simulink model "kinovaMicoSimscapeModel"  (R2021b)
(part 39 of 50)

Y3_5_1=dq5*dqr2*sin(q5)*((300773*3^(1/2))/80000000 - 1369/4000000) - (25433*dq2*dqr2*sin(q3))/400000 - (25433*dq1*dqr1*sin(q3))/800000 + (25433*dq1*dqr1*cos(2*q2)*sin(q3))/800000 - (25433*dq1*dqr1*sin(2*q2)*cos(q3))/800000 - (1369*dq4*dqr2*cos(2*q5)*sin(2*q4))/3200000 + (1369*dq5*dqr1*cos(q2)*sin(q3))/4000000 - (1369*dq5*dqr1*cos(q3)*sin(q2))/4000000 - (4107*dq4*dqr1*cos(2*q5)*cos(q2)*sin(q3))/16000000 + (4107*dq4*dqr1*cos(2*q5)*cos(q3)*sin(q2))/16000000 + dq1*dqr1*cos(2*q2)*sin(2*q3)*((23717*3^(1/2))/40000000 - 36744657/1600000000) - dq1*dqr1*cos(2*q3)*sin(2*q2)*((23717*3^(1/2))/40000000 - 36744657/1600000000) + dq4*dqr1*cos(q2)*sin(q3)*((23717*3^(1/2))/20000000 + 2122493/800000000) - dq4*dqr1*cos(q3)*sin(q2)*((23717*3^(1/2))/20000000 + 2122493/800000000) - (1073*3^(1/2)*dq1*dqr1*cos(q5)*sin(q3))/400000 - (1073*3^(1/2)*dq2*dqr2*cos(q5)*sin(q3))/200000 + dq4*dqr2*cos(2*q4)*sin(q5)*((23717*3^(1/2))/20000000 + 1369/1000000) + dq4*dqr2*sin(2*q4)*cos(q5)*((23717*3^(1/2))/40000000 + 1369/2000000) + dq5*dqr2*sin(2*q4)*cos(q5)*((23717*3^(1/2))/40000000 + 1369/2000000) + dq5*dqr2*cos(2*q4)*sin(q5)*((23717*3^(1/2))/80000000 + 1369/4000000) + (1073*dq1*dqr1*cos(q3)*cos(q4)*sin(q5))/200000 + (1073*dq1*dqr1*cos(q3)*cos(q5)*sin(q4))/400000 + (1073*dq2*dqr2*cos(q3)*cos(q4)*sin(q5))/100000 + (1073*dq2*dqr2*cos(q3)*cos(q5)*sin(q4))/200000 - (12321*dq1*dqr1*cos(2*q2)*cos(2*q5)*sin(2*q3))/32000000 + (12321*dq1*dqr1*cos(2*q3)*cos(2*q5)*sin(2*q2))/32000000 - dq2*dqr2*cos(q3)*sin(q4)*((18589*3^(1/2))/2000000 + 1073/100000) - dq1*dqr1*cos(q3)*sin(q4)*((18589*3^(1/2))/4000000 + 1073/200000) - (1369*dq1*dqr1*cos(2*q2)*cos(2*q4)*cos(2*q5)*sin(2*q3))/6400000 + (1369*dq1*dqr1*cos(2*q3)*cos(2*q4)*cos(2*q5)*sin(2*q2))/6400000 - (1073*dq1*dqr1*sin(2*q2)*cos(q4)*sin(q3)*sin(q5))/200000 - (1073*dq1*dqr1*sin(2*q2)*cos(q5)*sin(q3)*sin(q4))/400000 + (1369*3^(1/2)*dq5*dqr1*cos(q2)*cos(q3)*sin(q4))/4000000 + (1369*dq1*dqr1*cos(2*q2)*sin(2*q3)*sin(2*q4)*sin(2*q5))/8000000 - (1369*dq1*dqr1*cos(2*q3)*sin(2*q2)*sin(2*q4)*sin(2*q5))/8000000 + dq1*dqr1*cos(2*q2)*cos(q3)*sin(q4)*((18589*3^(1/2))/4000000 + 1073/200000) + (1369*3^(1/2)*dq5*dqr1*sin(q2)*sin(q3)*sin(q4))/4000000 + (32449*dq1*dqr1*cos(2*q2)*cos(2*q3)*cos(q4)*sin(q5))/4000000 - (1369*dq4*dqr1*cos(2*q4)*cos(2*q5)*cos(q2)*sin(q3))/3200000 + (1369*dq4*dqr1*cos(2*q4)*cos(2*q5)*cos(q3)*sin(q2))/3200000 - (1369*dq5*dqr1*cos(2*q4)*cos(2*q5)*cos(q2)*sin(q3))/4000000 + (1369*dq5*dqr1*cos(2*q4)*cos(2*q5)*cos(q3)*sin(q2))/4000000 + dq1*dqr1*sin(2*q2)*sin(q3)*sin(q4)*((18589*3^(1/2))/4000000 + 1073/200000) - dq1*dqr1*cos(2*q2)*cos(2*q4)*sin(2*q3)*((23717*3^(1/2))/40000000 + 1574893/1600000000) + dq1*dqr1*cos(2*q3)*cos(2*q4)*sin(2*q2)*((23717*3^(1/2))/40000000 + 1574893/1600000000) - dq4*dqr1*cos(2*q4)*cos(q2)*sin(q3)*((23717*3^(1/2))/20000000 + 1574893/800000000) + dq4*dqr1*cos(2*q4)*cos(q3)*sin(q2)*((23717*3^(1/2))/20000000 + 1574893/800000000) + (32449*dq1*dqr1*sin(2*q2)*sin(2*q3)*cos(q4)*sin(q5))/4000000 + (1369*dq4*dqr1*sin(2*q4)*sin(2*q5)*cos(q2)*sin(q3))/4000000 - (1369*dq4*dqr1*sin(2*q4)*sin(2*q5)*cos(q3)*sin(q2))/4000000 + (1369*dq5*dqr1*sin(2*q4)*sin(2*q5)*cos(q2)*sin(q3))/3200000 - (1369*dq5*dqr1*sin(2*q4)*sin(2*q5)*cos(q3)*sin(q2))/3200000 + (1073*3^(1/2)*dq1*dqr1*cos(2*q2)*cos(q5)*sin(q3))/400000 - (1073*3^(1/2)*dq1*dqr1*sin(2*q2)*cos(q3)*cos(q5))/400000 + (32449*dq4*dqr1*cos(q2)*cos(q3)*cos(q4)*sin(q5))/4000000 + (32449*dq5*dqr1*cos(q2)*cos(q3)*cos(q4)*sin(q5))/8000000 + (32449*dq5*dqr1*cos(q2)*cos(q3)*cos(q5)*sin(q4))/4000000 - dq1*dqr1*cos(2*q2)*sin(2*q3)*cos(q5)*((348207*3^(1/2))/80000000 + 1369/4000000) + dq1*dqr1*cos(2*q3)*sin(2*q2)*cos(q5)*((348207*3^(1/2))/80000000 + 1369/4000000) - dq1*dqr1*cos(2*q2)*cos(2*q3)*sin(q4)*((548467*3^(1/2))/80000000 + 32449/4000000) + (32449*dq4*dqr1*cos(q4)*sin(q2)*sin(q3)*sin(q5))/4000000 + (32449*dq5*dqr1*cos(q4)*sin(q2)*sin(q3)*sin(q5))/8000000 + (32449*dq5*dqr1*cos(q5)*sin(q2)*sin(q3)*sin(q4))/4000000 - dq1*dqr1*sin(2*q2)*sin(2*q3)*sin(q4)*((548467*3^(1/2))/80000000 + 32449/4000000) - dq4*dqr1*cos(q2)*cos(q5)*sin(q3)*((23717*3^(1/2))/40000000 + 1369/2000000) + dq4*dqr1*cos(q3)*cos(q5)*sin(q2)*((23717*3^(1/2))/40000000 + 1369/2000000) - dq5*dqr1*cos(q2)*cos(q5)*sin(q3)*((23717*3^(1/2))/40000000 + 1369/2000000) + dq5*dqr1*cos(q3)*cos(q5)*sin(q2)*((23717*3^(1/2))/40000000 + 1369/2000000) - dq4*dqr1*cos(q2)*cos(q3)*sin(q4)*((548467*3^(1/2))/80000000 + 32449/4000000) - (1073*dq1*dqr1*cos(2*q2)*cos(q3)*cos(q4)*sin(q5))/200000 - (1073*dq1*dqr1*cos(2*q2)*cos(q3)*cos(q5)*sin(q4))/400000 - dq4*dqr1*sin(q2)*sin(q3)*sin(q4)*((548467*3^(1/2))/80000000 + 32449/4000000) + (1369*3^(1/2)*dq1*dqr1*cos(2*q2)*cos(2*q3)*cos(2*q5)*sin(q4))/8000000 + (1369*3^(1/2)*dq1*dqr1*cos(2*q2)*cos(2*q3)*sin(2*q5)*cos(q4))/4000000 + dq4*dqr1*cos(2*q4)*cos(q2)*cos(q5)*sin(q3)*((23717*3^(1/2))/40000000 + 1369/2000000) - dq4*dqr1*cos(2*q4)*cos(q3)*cos(q5)*sin(q2)*((23717*3^(1/2))/40000000 + 1369/2000000) + dq5*dqr1*cos(2*q4)*cos(q2)*cos(q5)*sin(q3)*((23717*3^(1/2))/40000000 + 1369/2000000) - dq5*dqr1*cos(2*q4)*cos(q3)*cos(q5)*sin(q2)*((23717*3^(1/2))/40000000 + 1369/2000000) + (1369*3^(1/2)*dq1*dqr1*cos(2*q5)*sin(2*q2)*sin(2*q3)*sin(q4))/8000000 + (1369*3^(1/2)*dq1*dqr1*sin(2*q2)*sin(2*q3)*sin(2*q5)*cos(q4))/4000000 - dq4*dqr1*sin(2*q4)*cos(q2)*sin(q3)*sin(q5)*((23717*3^(1/2))/20000000 + 1369/1000000) + dq4*dqr1*sin(2*q4)*cos(q3)*sin(q2)*sin(q5)*((23717*3^(1/2))/20000000 + 1369/1000000) - dq5*dqr1*sin(2*q4)*cos(q2)*sin(q3)*sin(q5)*((23717*3^(1/2))/80000000 + 1369/4000000) + dq5*dqr1*sin(2*q4)*cos(q3)*sin(q2)*sin(q5)*((23717*3^(1/2))/80000000 + 1369/4000000) + (1369*3^(1/2)*dq4*dqr1*cos(2*q5)*cos(q2)*cos(q3)*sin(q4))/8000000 + (1369*3^(1/2)*dq4*dqr1*sin(2*q5)*cos(q2)*cos(q3)*cos(q4))/4000000 + (1369*3^(1/2)*dq5*dqr1*cos(2*q5)*cos(q2)*cos(q3)*sin(q4))/4000000 + (1369*3^(1/2)*dq5*dqr1*sin(2*q5)*cos(q2)*cos(q3)*cos(q4))/8000000 - dq1*dqr1*cos(2*q2)*cos(2*q3)*cos(q5)*sin(q4)*((1369*3^(1/2))/2000000 - 45547/20000000) + (1369*3^(1/2)*dq4*dqr1*cos(2*q5)*sin(q2)*sin(q3)*sin(q4))/8000000 + (1369*3^(1/2)*dq4*dqr1*sin(2*q5)*cos(q4)*sin(q2)*sin(q3))/4000000 + (1369*3^(1/2)*dq5*dqr1*cos(2*q5)*sin(q2)*sin(q3)*sin(q4))/4000000 + (1369*3^(1/2)*dq5*dqr1*sin(2*q5)*cos(q4)*sin(q2)*sin(q3))/8000000 - dq1*dqr1*sin(2*q2)*sin(2*q3)*cos(q5)*sin(q4)*((1369*3^(1/2))/2000000 - 45547/20000000) - dq4*dqr1*cos(q2)*cos(q3)*cos(q5)*sin(q4)*((1369*3^(1/2))/2000000 - 45547/20000000) - dq4*dqr1*cos(q5)*sin(q2)*sin(q3)*sin(q4)*((1369*3^(1/2))/2000000 - 45547/20000000) + dq1*dqr1*cos(2*q2)*cos(2*q4)*sin(2*q3)*cos(q5)*((23717*3^(1/2))/80000000 + 1369/4000000) - dq1*dqr1*cos(2*q3)*cos(2*q4)*sin(2*q2)*cos(q5)*((23717*3^(1/2))/80000000 + 1369/4000000) - dq1*dqr1*cos(2*q2)*sin(2*q3)*sin(2*q4)*sin(q5)*((23717*3^(1/2))/40000000 + 1369/2000000) + dq1*dqr1*cos(2*q3)*sin(2*q2)*sin(2*q4)*sin(q5)*((23717*3^(1/2))/40000000 + 1369/2000000);
Y3_5_2=(4107*dq2*dqr5*sin(2*q5))/16000000 + (4107*dq5*dqr2*sin(2*q5))/16000000 - (4107*dq5*dqr3*sin(2*q5))/16000000 + dq2*dqr5*sin(q5)*((300773*3^(1/2))/80000000 - 1369/4000000) - dq3*dqr5*sin(q5)*((300773*3^(1/2))/80000000 - 1369/4000000) - dq5*dqr3*sin(q5)*((300773*3^(1/2))/80000000 - 1369/4000000) - dq4*dqr4*sin(q4)*((548467*3^(1/2))/80000000 + 32449/4000000) + (1369*3^(1/2)*dq4*dqr5*sin(q4))/4000000 + (1369*3^(1/2)*dq5*dqr4*sin(q4))/4000000 - (1369*dq2*dqr4*cos(2*q4)*sin(2*q5))/4000000 - (1369*dq2*dqr4*cos(2*q5)*sin(2*q4))/3200000 - (1369*dq4*dqr2*cos(2*q4)*sin(2*q5))/4000000 - (1369*dq2*dqr5*cos(2*q4)*sin(2*q5))/3200000 - (1369*dq2*dqr5*cos(2*q5)*sin(2*q4))/4000000 + (1369*dq3*dqr4*cos(2*q4)*sin(2*q5))/4000000 + (1369*dq3*dqr4*cos(2*q5)*sin(2*q4))/3200000 + (1369*dq4*dqr3*cos(2*q4)*sin(2*q5))/4000000 + (1369*dq4*dqr3*cos(2*q5)*sin(2*q4))/3200000 - (1369*dq5*dqr2*cos(2*q4)*sin(2*q5))/3200000 - (1369*dq5*dqr2*cos(2*q5)*sin(2*q4))/4000000 + (1369*dq5*dqr3*cos(2*q4)*sin(2*q5))/3200000 + (1369*dq5*dqr3*cos(2*q5)*sin(2*q4))/4000000 - dq2*dqr4*sin(2*q4)*((23717*3^(1/2))/20000000 + 1574893/800000000) - dq4*dqr2*sin(2*q4)*((23717*3^(1/2))/20000000 + 1574893/800000000) + dq3*dqr4*sin(2*q4)*((23717*3^(1/2))/20000000 + 1574893/800000000) + dq4*dqr3*sin(2*q4)*((23717*3^(1/2))/20000000 + 1574893/800000000) + (1369*dq1*dqr5*cos(q2)*sin(q3))/4000000 - (1369*dq1*dqr5*cos(q3)*sin(q2))/4000000 + (32449*dq4*dqr4*cos(q4)*sin(q5))/4000000 + (32449*dq4*dqr5*cos(q4)*sin(q5))/8000000 + (32449*dq4*dqr5*cos(q5)*sin(q4))/4000000 + (32449*dq5*dqr4*cos(q4)*sin(q5))/8000000 + (32449*dq5*dqr4*cos(q5)*sin(q4))/4000000 + (32449*dq5*dqr5*cos(q4)*sin(q5))/4000000 + dq5*dqr5*cos(q5)*sin(q4)*((1369*3^(1/2))/2000000 + 58349/10000000) - dq4*dqr4*cos(q5)*sin(q4)*((1369*3^(1/2))/2000000 - 45547/20000000) - (4107*dq1*dqr4*cos(2*q5)*cos(q2)*sin(q3))/16000000 + (4107*dq1*dqr4*cos(2*q5)*cos(q3)*sin(q2))/16000000 + dq1*dqr4*cos(q2)*sin(q3)*((23717*3^(1/2))/20000000 + 2122493/800000000) - dq1*dqr4*cos(q3)*sin(q2)*((23717*3^(1/2))/20000000 + 2122493/800000000) + dq2*dqr4*cos(2*q4)*sin(q5)*((23717*3^(1/2))/20000000 + 1369/1000000) - dq3*dqr4*cos(2*q4)*sin(q5)*((23717*3^(1/2))/20000000 + 1369/1000000) - dq4*dqr3*cos(2*q4)*sin(q5)*((23717*3^(1/2))/20000000 + 1369/1000000) + dq2*dqr4*sin(2*q4)*cos(q5)*((23717*3^(1/2))/40000000 + 1369/2000000) + dq2*dqr5*sin(2*q4)*cos(q5)*((23717*3^(1/2))/40000000 + 1369/2000000) - dq3*dqr4*sin(2*q4)*cos(q5)*((23717*3^(1/2))/40000000 + 1369/2000000) - dq4*dqr3*sin(2*q4)*cos(q5)*((23717*3^(1/2))/40000000 + 1369/2000000) - dq3*dqr5*sin(2*q4)*cos(q5)*((23717*3^(1/2))/40000000 + 1369/2000000) - dq5*dqr3*sin(2*q4)*cos(q5)*((23717*3^(1/2))/40000000 + 1369/2000000) + dq2*dqr5*cos(2*q4)*sin(q5)*((23717*3^(1/2))/80000000 + 1369/4000000) - dq3*dqr5*cos(2*q4)*sin(q5)*((23717*3^(1/2))/80000000 + 1369/4000000) - dq5*dqr3*cos(2*q4)*sin(q5)*((23717*3^(1/2))/80000000 + 1369/4000000) + (1369*3^(1/2)*dq4*dqr4*cos(2*q5)*sin(q4))/8000000 + (1369*3^(1/2)*dq4*dqr4*sin(2*q5)*cos(q4))/4000000 + (1369*3^(1/2)*dq4*dqr5*cos(2*q5)*sin(q4))/4000000 + (1369*3^(1/2)*dq4*dqr5*sin(2*q5)*cos(q4))/8000000 + (1369*3^(1/2)*dq5*dqr4*cos(2*q5)*sin(q4))/4000000 + (1369*3^(1/2)*dq5*dqr4*sin(2*q5)*cos(q4))/8000000 + (1369*3^(1/2)*dq1*dqr5*cos(q2)*cos(q3)*sin(q4))/4000000 + (1369*3^(1/2)*dq1*dqr5*sin(q2)*sin(q3)*sin(q4))/4000000 - (1369*dq1*dqr4*cos(2*q4)*cos(2*q5)*cos(q2)*sin(q3))/3200000 + (1369*dq1*dqr4*cos(2*q4)*cos(2*q5)*cos(q3)*sin(q2))/3200000 - (1369*dq1*dqr5*cos(2*q4)*cos(2*q5)*cos(q2)*sin(q3))/4000000 + (1369*dq1*dqr5*cos(2*q4)*cos(2*q5)*cos(q3)*sin(q2))/4000000 - dq1*dqr4*cos(2*q4)*cos(q2)*sin(q3)*((23717*3^(1/2))/20000000 + 1574893/800000000) + dq1*dqr4*cos(2*q4)*cos(q3)*sin(q2)*((23717*3^(1/2))/20000000 + 1574893/800000000) + (1369*dq1*dqr4*sin(2*q4)*sin(2*q5)*cos(q2)*sin(q3))/4000000 - (1369*dq1*dqr4*sin(2*q4)*sin(2*q5)*cos(q3)*sin(q2))/4000000 + (1369*dq1*dqr5*sin(2*q4)*sin(2*q5)*cos(q2)*sin(q3))/3200000 - (1369*dq1*dqr5*sin(2*q4)*sin(2*q5)*cos(q3)*sin(q2))/3200000 + (32449*dq1*dqr4*cos(q2)*cos(q3)*cos(q4)*sin(q5))/4000000 + (32449*dq1*dqr5*cos(q2)*cos(q3)*cos(q4)*sin(q5))/8000000 + (32449*dq1*dqr5*cos(q2)*cos(q3)*cos(q5)*sin(q4))/4000000 + (32449*dq1*dqr4*cos(q4)*sin(q2)*sin(q3)*sin(q5))/4000000 + (32449*dq1*dqr5*cos(q4)*sin(q2)*sin(q3)*sin(q5))/8000000 + (32449*dq1*dqr5*cos(q5)*sin(q2)*sin(q3)*sin(q4))/4000000 - dq1*dqr4*cos(q2)*cos(q5)*sin(q3)*((23717*3^(1/2))/40000000 + 1369/2000000) + dq1*dqr4*cos(q3)*cos(q5)*sin(q2)*((23717*3^(1/2))/40000000 + 1369/2000000) - dq1*dqr5*cos(q2)*cos(q5)*sin(q3)*((23717*3^(1/2))/40000000 + 1369/2000000) + dq1*dqr5*cos(q3)*cos(q5)*sin(q2)*((23717*3^(1/2))/40000000 + 1369/2000000) - dq1*dqr4*cos(q2)*cos(q3)*sin(q4)*((548467*3^(1/2))/80000000 + 32449/4000000) - dq1*dqr4*sin(q2)*sin(q3)*sin(q4)*((548467*3^(1/2))/80000000 + 32449/4000000) + dq1*dqr4*cos(2*q4)*cos(q2)*cos(q5)*sin(q3)*((23717*3^(1/2))/40000000 + 1369/2000000) - dq1*dqr4*cos(2*q4)*cos(q3)*cos(q5)*sin(q2)*((23717*3^(1/2))/40000000 + 1369/2000000) + dq1*dqr5*cos(2*q4)*cos(q2)*cos(q5)*sin(q3)*((23717*3^(1/2))/40000000 + 1369/2000000) - dq1*dqr5*cos(2*q4)*cos(q3)*cos(q5)*sin(q2)*((23717*3^(1/2))/40000000 + 1369/2000000) - dq1*dqr4*sin(2*q4)*cos(q2)*sin(q3)*sin(q5)*((23717*3^(1/2))/20000000 + 1369/1000000) + dq1*dqr4*sin(2*q4)*cos(q3)*sin(q2)*sin(q5)*((23717*3^(1/2))/20000000 + 1369/1000000) - dq1*dqr5*sin(2*q4)*cos(q2)*sin(q3)*sin(q5)*((23717*3^(1/2))/80000000 + 1369/4000000) + dq1*dqr5*sin(2*q4)*cos(q3)*sin(q2)*sin(q5)*((23717*3^(1/2))/80000000 + 1369/4000000) + (1369*3^(1/2)*dq1*dqr4*cos(2*q5)*cos(q2)*cos(q3)*sin(q4))/8000000 + (1369*3^(1/2)*dq1*dqr4*sin(2*q5)*cos(q2)*cos(q3)*cos(q4))/4000000 + (1369*3^(1/2)*dq1*dqr5*cos(2*q5)*cos(q2)*cos(q3)*sin(q4))/4000000 + (1369*3^(1/2)*dq1*dqr5*sin(2*q5)*cos(q2)*cos(q3)*cos(q4))/8000000 + (1369*3^(1/2)*dq1*dqr4*cos(2*q5)*sin(q2)*sin(q3)*sin(q4))/8000000 + (1369*3^(1/2)*dq1*dqr4*sin(2*q5)*cos(q4)*sin(q2)*sin(q3))/4000000 + (1369*3^(1/2)*dq1*dqr5*cos(2*q5)*sin(q2)*sin(q3)*sin(q4))/4000000 + (1369*3^(1/2)*dq1*dqr5*sin(2*q5)*cos(q4)*sin(q2)*sin(q3))/8000000 - dq1*dqr4*cos(q2)*cos(q3)*cos(q5)*sin(q4)*((1369*3^(1/2))/2000000 - 45547/20000000) - dq1*dqr4*cos(q5)*sin(q2)*sin(q3)*sin(q4)*((1369*3^(1/2))/2000000 - 45547/20000000);
Y3_5_3=(25433*ddqr2*cos(q3))/400000 - ddqr2*((23717*3^(1/2))/10000000 + 5252117/100000000) + ddqr3*((23717*3^(1/2))/10000000 + 5252117/100000000) - (1369*ddqr2*cos(q5)^2)/1000000 + (1369*ddqr3*cos(q5)^2)/1000000 + (1369*ddqr2*cos(q4)^2*cos(q5)^2)/800000 - (1369*ddqr3*cos(q4)^2*cos(q5)^2)/800000 + ddqr2*cos(q4)^2*((23717*3^(1/2))/10000000 + 1232643/400000000) - ddqr3*cos(q4)^2*((23717*3^(1/2))/10000000 + 1232643/400000000) - (4107*dq3*dqr5*sin(2*q5))/16000000 - (6139*ddqr1*cos(q2)*cos(q3))/4000000 - (32449*ddqr5*cos(q4)*cos(q5))/4000000 - (6139*ddqr1*sin(q2)*sin(q3))/4000000 + (32449*ddqr4*sin(q4)*sin(q5))/4000000 - ddqr2*cos(q5)*((4329*3^(1/2))/625000 - 1369/1000000) + ddqr3*cos(q5)*((4329*3^(1/2))/625000 - 1369/1000000) + ddqr4*cos(q4)*((562157*3^(1/2))/80000000 + 32449/4000000) - (1369*3^(1/2)*ddqr5*cos(q4))/2000000 - (1369*3^(1/2)*ddqr4*cos(q4)*cos(q5)^2)/4000000 + (1073*ddqr2*cos(q4)*sin(q3)*sin(q5))/100000 + (1073*ddqr2*cos(q5)*sin(q3)*sin(q4))/200000 + ddqr4*cos(q4)*cos(q5)*((1369*3^(1/2))/2000000 - 45547/20000000) + (1369*dq3*dqr5*cos(2*q4)*sin(2*q5))/3200000 + (1369*dq3*dqr5*cos(2*q5)*sin(2*q4))/4000000 - ddqr2*sin(q3)*sin(q4)*((18589*3^(1/2))/2000000 + 1073/100000) + ddqr5*sin(q4)*sin(q5)*((1369*3^(1/2))/2000000 + 58349/10000000) + (1073*3^(1/2)*ddqr2*cos(q3)*cos(q5))/200000 - ddqr2*cos(q4)^2*cos(q5)*((23717*3^(1/2))/20000000 + 1369/1000000) + ddqr3*cos(q4)^2*cos(q5)*((23717*3^(1/2))/20000000 + 1369/1000000) + (32449*ddqr1*cos(q2)*cos(q3)*sin(q4)*sin(q5))/4000000 - (259*ddqr1*cos(q2)*cos(q4)*sin(q3)*sin(q5))/1000000 - (259*ddqr1*cos(q2)*cos(q5)*sin(q3)*sin(q4))/2000000 + (259*ddqr1*cos(q3)*cos(q4)*sin(q2)*sin(q5))/1000000 + (259*ddqr1*cos(q3)*cos(q5)*sin(q2)*sin(q4))/2000000 + (1369*ddqr1*cos(q2)*cos(q5)*sin(q3)*sin(q5))/2000000 - (1369*ddqr1*cos(q3)*cos(q5)*sin(q2)*sin(q5))/2000000 - (1369*ddqr2*cos(q4)*cos(q5)*sin(q4)*sin(q5))/1000000 + (1369*ddqr3*cos(q4)*cos(q5)*sin(q4)*sin(q5))/1000000 + (32449*ddqr1*sin(q2)*sin(q3)*sin(q4)*sin(q5))/4000000 + ddqr1*cos(q2)*cos(q3)*cos(q4)*((562157*3^(1/2))/80000000 + 32449/4000000) + ddqr2*cos(q4)*sin(q4)*sin(q5)*((23717*3^(1/2))/10000000 + 1369/500000) - ddqr3*cos(q4)*sin(q4)*sin(q5)*((23717*3^(1/2))/10000000 + 1369/500000) + ddqr1*cos(q2)*sin(q3)*sin(q4)*((4487*3^(1/2))/20000000 + 259/1000000) - ddqr1*cos(q3)*sin(q2)*sin(q4)*((4487*3^(1/2))/20000000 + 259/1000000) - ddqr1*cos(q2)*sin(q3)*sin(q5)*((23717*3^(1/2))/20000000 + 1369/1000000) + ddqr1*cos(q3)*sin(q2)*sin(q5)*((23717*3^(1/2))/20000000 + 1369/1000000) + ddqr1*cos(q4)*sin(q2)*sin(q3)*((562157*3^(1/2))/80000000 + 32449/4000000) - (259*3^(1/2)*ddqr1*cos(q2)*cos(q3)*cos(q5))/2000000 - (259*3^(1/2)*ddqr1*cos(q5)*sin(q2)*sin(q3))/2000000 + (1369*3^(1/2)*ddqr4*cos(q5)*sin(q4)*sin(q5))/2000000 + ddqr1*cos(q2)*cos(q3)*cos(q4)*cos(q5)*((1369*3^(1/2))/2000000 - 45547/20000000) + ddqr1*cos(q4)*cos(q5)*sin(q2)*sin(q3)*((1369*3^(1/2))/2000000 - 45547/20000000) - (1369*ddqr1*cos(q2)*cos(q4)*cos(q5)^2*sin(q3)*sin(q4))/800000 + (1369*ddqr1*cos(q3)*cos(q4)*cos(q5)^2*sin(q2)*sin(q4))/800000 - (1369*ddqr1*cos(q2)*cos(q4)^2*cos(q5)*sin(q3)*sin(q5))/1000000 + (1369*ddqr1*cos(q3)*cos(q4)^2*cos(q5)*sin(q2)*sin(q5))/1000000 - ddqr1*cos(q2)*cos(q4)*sin(q3)*sin(q4)*((23717*3^(1/2))/10000000 + 1232643/400000000) + ddqr1*cos(q3)*cos(q4)*sin(q2)*sin(q4)*((23717*3^(1/2))/10000000 + 1232643/400000000) + ddqr1*cos(q2)*cos(q4)^2*sin(q3)*sin(q5)*((23717*3^(1/2))/10000000 + 1369/500000) - ddqr1*cos(q3)*cos(q4)^2*sin(q2)*sin(q5)*((23717*3^(1/2))/10000000 + 1369/500000) - (1369*3^(1/2)*ddqr1*cos(q2)*cos(q3)*cos(q4)*cos(q5)^2)/4000000 - (1369*3^(1/2)*ddqr1*cos(q4)*cos(q5)^2*sin(q2)*sin(q3))/4000000 + ddqr1*cos(q2)*cos(q4)*cos(q5)*sin(q3)*sin(q4)*((23717*3^(1/2))/20000000 + 1369/1000000) - ddqr1*cos(q3)*cos(q4)*cos(q5)*sin(q2)*sin(q4)*((23717*3^(1/2))/20000000 + 1369/1000000) + (1369*3^(1/2)*ddqr1*cos(q2)*cos(q3)*cos(q5)*sin(q4)*sin(q5))/2000000 + (1369*3^(1/2)*ddqr1*cos(q5)*sin(q2)*sin(q3)*sin(q4)*sin(q5))/2000000;
Y3_7_1=(29*ddqr2*cos(q3))/100 - (29*dq1*dqr1*sin(q3))/200 - (29*dq2*dqr2*sin(q3))/100 + (ddqr1*cos(q2)*cos(q3))/625 + (ddqr1*sin(q2)*sin(q3))/625 + (29*dq1*dqr1*cos(2*q2)*sin(q3))/200 - (29*dq1*dqr1*sin(2*q2)*cos(q3))/200;
Y3_8_1=(1231*dq4*dqr4*sin(q4))/10000 - (1231*ddqr4*cos(q4))/10000 + (29*ddqr2*sin(q3)*sin(q4))/100 - (1231*ddqr1*cos(q2)*cos(q3)*cos(q4))/10000 - (7*ddqr1*cos(q2)*sin(q3)*sin(q4))/1000 + (7*ddqr1*cos(q3)*sin(q2)*sin(q4))/1000 - (1231*ddqr1*cos(q4)*sin(q2)*sin(q3))/10000 + (29*dq1*dqr1*cos(q3)*sin(q4))/200 + (29*dq2*dqr2*cos(q3)*sin(q4))/100 - (29*dq1*dqr1*cos(2*q2)*cos(q3)*sin(q4))/200 - (29*dq1*dqr1*sin(2*q2)*sin(q3)*sin(q4))/200 + (1231*dq1*dqr1*cos(2*q2)*cos(2*q3)*sin(q4))/10000 + (1231*dq1*dqr1*sin(2*q2)*sin(2*q3)*sin(q4))/10000 + (1231*dq1*dqr4*cos(q2)*cos(q3)*sin(q4))/10000 + (1231*dq4*dqr1*cos(q2)*cos(q3)*sin(q4))/10000 + (1231*dq1*dqr4*sin(q2)*sin(q3)*sin(q4))/10000 + (1231*dq4*dqr1*sin(q2)*sin(q3)*sin(q4))/10000;
Y3_9_1=dq3*dqr5*sin(q5)*((117*3^(1/2))/1250 - 37/4000) - dq5*dqr2*sin(q5)*((117*3^(1/2))/1250 - 37/4000) - dq2*dqr5*sin(q5)*((117*3^(1/2))/1250 - 37/4000) + dq5*dqr3*sin(q5)*((117*3^(1/2))/1250 - 37/4000) - (37*dq2*dqr4*cos(2*q4)*sin(q5))/1000 - (37*dq2*dqr4*sin(2*q4)*cos(q5))/2000 - (37*dq4*dqr2*cos(2*q4)*sin(q5))/1000 - (37*dq4*dqr2*sin(2*q4)*cos(q5))/2000 - (37*dq2*dqr5*cos(2*q4)*sin(q5))/4000 - (37*dq2*dqr5*sin(2*q4)*cos(q5))/2000 + (37*dq3*dqr4*cos(2*q4)*sin(q5))/1000 + (37*dq3*dqr4*sin(2*q4)*cos(q5))/2000 + (37*dq4*dqr3*cos(2*q4)*sin(q5))/1000 + (37*dq4*dqr3*sin(2*q4)*cos(q5))/2000 - (37*dq5*dqr2*cos(2*q4)*sin(q5))/4000 - (37*dq5*dqr2*sin(2*q4)*cos(q5))/2000 + (37*dq3*dqr5*cos(2*q4)*sin(q5))/4000 + (37*dq3*dqr5*sin(2*q4)*cos(q5))/2000 + (37*dq5*dqr3*cos(2*q4)*sin(q5))/4000 + (37*dq5*dqr3*sin(2*q4)*cos(q5))/2000 - (37*ddqr1*cos(q3)*sin(q2)*sin(q5))/1000 - (117*dq4*dqr4*cos(q4)*sin(q5))/625 - (117*dq4*dqr5*cos(q4)*sin(q5))/1250 - (117*dq4*dqr5*cos(q5)*sin(q4))/625 - (117*dq5*dqr4*cos(q4)*sin(q5))/1250 - (117*dq5*dqr4*cos(q5)*sin(q4))/625 - (117*dq5*dqr5*cos(q4)*sin(q5))/625 + (7*ddqr1*cos(q2)*cos(q5)*sin(q3)*sin(q4))/2000 - (7*ddqr1*cos(q3)*cos(q4)*sin(q2)*sin(q5))/1000 - (7*ddqr1*cos(q3)*cos(q5)*sin(q2)*sin(q4))/2000 + (29*3^(1/2)*dq1*dqr1*cos(q5)*sin(q3))/400 + (29*3^(1/2)*dq2*dqr2*cos(q5)*sin(q3))/200 - (117*ddqr1*sin(q2)*sin(q3)*sin(q4)*sin(q5))/625 + (37*ddqr1*cos(q3)*cos(q4)^2*sin(q2)*sin(q5))/500 - (29*dq1*dqr1*cos(q3)*cos(q4)*sin(q5))/200 - (29*dq1*dqr1*cos(q3)*cos(q5)*sin(q4))/400 + (37*dq1*dqr4*cos(q2)*cos(q5)*sin(q3))/2000 - (37*dq1*dqr4*cos(q3)*cos(q5)*sin(q2))/2000 + (37*dq4*dqr1*cos(q2)*cos(q5)*sin(q3))/2000 - (37*dq4*dqr1*cos(q3)*cos(q5)*sin(q2))/2000 + (37*dq1*dqr5*cos(q2)*cos(q5)*sin(q3))/2000 - (37*dq1*dqr5*cos(q3)*cos(q5)*sin(q2))/2000 - (29*dq2*dqr2*cos(q3)*cos(q4)*sin(q5))/100 - (29*dq2*dqr2*cos(q3)*cos(q5)*sin(q4))/200 + (37*dq5*dqr1*cos(q2)*cos(q5)*sin(q3))/2000 - (37*dq5*dqr1*cos(q3)*cos(q5)*sin(q2))/2000 + (7*3^(1/2)*ddqr1*cos(q5)*sin(q2)*sin(q3))/2000 + dq4*dqr4*cos(q5)*sin(q4)*((37*3^(1/2))/2000 - 117/1250) - dq5*dqr5*cos(q5)*sin(q4)*((37*3^(1/2))/2000 + 117/1250) + (29*dq1*dqr1*sin(2*q2)*cos(q4)*sin(q3)*sin(q5))/200 + (29*dq1*dqr1*sin(2*q2)*cos(q5)*sin(q3)*sin(q4))/400 + (37*dq1*dqr4*sin(2*q4)*cos(q2)*sin(q3)*sin(q5))/1000 - (37*dq1*dqr4*sin(2*q4)*cos(q3)*sin(q2)*sin(q5))/1000 + (37*dq4*dqr1*sin(2*q4)*cos(q2)*sin(q3)*sin(q5))/1000 - (37*dq4*dqr1*sin(2*q4)*cos(q3)*sin(q2)*sin(q5))/1000 + (37*dq1*dqr5*sin(2*q4)*cos(q2)*sin(q3)*sin(q5))/4000 - (37*dq1*dqr5*sin(2*q4)*cos(q3)*sin(q2)*sin(q5))/4000 + (37*dq5*dqr1*sin(2*q4)*cos(q2)*sin(q3)*sin(q5))/4000 - (37*dq5*dqr1*sin(2*q4)*cos(q3)*sin(q2)*sin(q5))/4000 - (37*ddqr1*cos(q2)*cos(q4)*cos(q5)*sin(q3)*sin(q4))/1000 + (37*ddqr1*cos(q3)*cos(q4)*cos(q5)*sin(q2)*sin(q4))/1000 - (117*dq1*dqr1*cos(2*q2)*cos(2*q3)*cos(q4)*sin(q5))/625 - ddqr1*cos(q4)*cos(q5)*sin(q2)*sin(q3)*((37*3^(1/2))/2000 - 117/1250) - (117*dq1*dqr1*sin(2*q2)*sin(2*q3)*cos(q4)*sin(q5))/625 - (29*3^(1/2)*dq1*dqr1*cos(2*q2)*cos(q5)*sin(q3))/400 + (29*3^(1/2)*dq1*dqr1*sin(2*q2)*cos(q3)*cos(q5))/400 - (117*dq1*dqr4*cos(q2)*cos(q3)*cos(q4)*sin(q5))/625 - (117*dq4*dqr1*cos(q2)*cos(q3)*cos(q4)*sin(q5))/625 - (117*dq1*dqr5*cos(q2)*cos(q3)*cos(q4)*sin(q5))/1250 - (117*dq1*dqr5*cos(q2)*cos(q3)*cos(q5)*sin(q4))/625 - (117*dq5*dqr1*cos(q2)*cos(q3)*cos(q4)*sin(q5))/1250 - (117*dq5*dqr1*cos(q2)*cos(q3)*cos(q5)*sin(q4))/625 + dq1*dqr1*cos(2*q2)*sin(2*q3)*cos(q5)*((117*3^(1/2))/1250 + 37/4000) - dq1*dqr1*cos(2*q3)*sin(2*q2)*cos(q5)*((117*3^(1/2))/1250 + 37/4000) - (37*dq1*dqr1*cos(2*q2)*cos(2*q4)*sin(2*q3)*cos(q5))/4000 + (37*dq1*dqr1*cos(2*q3)*cos(2*q4)*sin(2*q2)*cos(q5))/4000 - (117*dq1*dqr4*cos(q4)*sin(q2)*sin(q3)*sin(q5))/625 - (117*dq4*dqr1*cos(q4)*sin(q2)*sin(q3)*sin(q5))/625 - (117*dq1*dqr5*cos(q4)*sin(q2)*sin(q3)*sin(q5))/1250 - (117*dq1*dqr5*cos(q5)*sin(q2)*sin(q3)*sin(q4))/625 - (117*dq5*dqr1*cos(q4)*sin(q2)*sin(q3)*sin(q5))/1250 - (117*dq5*dqr1*cos(q5)*sin(q2)*sin(q3)*sin(q4))/625 + (37*dq1*dqr1*cos(2*q2)*sin(2*q3)*sin(2*q4)*sin(q5))/2000 - (37*dq1*dqr1*cos(2*q3)*sin(2*q2)*sin(2*q4)*sin(q5))/2000 + (29*dq1*dqr1*cos(2*q2)*cos(q3)*cos(q4)*sin(q5))/200 + (29*dq1*dqr1*cos(2*q2)*cos(q3)*cos(q5)*sin(q4))/400 - (37*dq1*dqr4*cos(2*q4)*cos(q2)*cos(q5)*sin(q3))/2000 + (37*dq1*dqr4*cos(2*q4)*cos(q3)*cos(q5)*sin(q2))/2000 - (37*dq4*dqr1*cos(2*q4)*cos(q2)*cos(q5)*sin(q3))/2000 + (37*dq4*dqr1*cos(2*q4)*cos(q3)*cos(q5)*sin(q2))/2000 - (37*dq1*dqr5*cos(2*q4)*cos(q2)*cos(q5)*sin(q3))/2000 + (37*dq1*dqr5*cos(2*q4)*cos(q3)*cos(q5)*sin(q2))/2000 - (37*dq5*dqr1*cos(2*q4)*cos(q2)*cos(q5)*sin(q3))/2000 + (37*dq5*dqr1*cos(2*q4)*cos(q3)*cos(q5)*sin(q2))/2000 + dq1*dqr1*cos(2*q2)*cos(2*q3)*cos(q5)*sin(q4)*((37*3^(1/2))/2000 - 117/1250) + dq1*dqr1*sin(2*q2)*sin(2*q3)*cos(q5)*sin(q4)*((37*3^(1/2))/2000 - 117/1250) + dq1*dqr4*cos(q2)*cos(q3)*cos(q5)*sin(q4)*((37*3^(1/2))/2000 - 117/1250) + dq4*dqr1*cos(q2)*cos(q3)*cos(q5)*sin(q4)*((37*3^(1/2))/2000 - 117/1250) + dq1*dqr4*cos(q5)*sin(q2)*sin(q3)*sin(q4)*((37*3^(1/2))/2000 - 117/1250) + dq4*dqr1*cos(q5)*sin(q2)*sin(q3)*sin(q4)*((37*3^(1/2))/2000 - 117/1250);
Y3_9_2=(117*ddqr5*cos(q4)*cos(q5))/625 - (117*ddqr4*sin(q4)*sin(q5))/625 + ddqr2*cos(q5)*((117*3^(1/2))/625 - 37/1000) - ddqr3*cos(q5)*((117*3^(1/2))/625 - 37/1000) + (37*ddqr2*cos(q4)^2*cos(q5))/1000 - (37*ddqr3*cos(q4)^2*cos(q5))/1000 + (37*ddqr1*cos(q2)*sin(q3)*sin(q5))/1000 - (29*ddqr2*cos(q4)*sin(q3)*sin(q5))/100 - (29*ddqr2*cos(q5)*sin(q3)*sin(q4))/200 - (37*ddqr2*cos(q4)*sin(q4)*sin(q5))/500 + (37*ddqr3*cos(q4)*sin(q4)*sin(q5))/500 - ddqr4*cos(q4)*cos(q5)*((37*3^(1/2))/2000 - 117/1250) - ddqr5*sin(q4)*sin(q5)*((37*3^(1/2))/2000 + 117/1250) - (29*3^(1/2)*ddqr2*cos(q3)*cos(q5))/200 - (117*ddqr1*cos(q2)*cos(q3)*sin(q4)*sin(q5))/625 + (7*ddqr1*cos(q2)*cos(q4)*sin(q3)*sin(q5))/1000 - (37*ddqr1*cos(q2)*cos(q4)^2*sin(q3)*sin(q5))/500 + (7*3^(1/2)*ddqr1*cos(q2)*cos(q3)*cos(q5))/2000 - ddqr1*cos(q2)*cos(q3)*cos(q4)*cos(q5)*((37*3^(1/2))/2000 - 117/1250);
Y3_10_1=(111*dq4*dqr1*sin(2*q5)*cos(q2)*sin(q3)*sin(q6))/8000 - (37*dq6*dqr1*cos(q3)*cos(q6)*sin(q2))/4000 - (87*dq1*dqr1*sin(2*q2)*cos(q6)*sin(q3)*sin(q4))/800 - (37*dq5*dqr1*cos(q3)*cos(q6)*sin(q2))/4000 - (111*dq4*dqr1*sin(2*q5)*cos(q3)*sin(q2)*sin(q6))/8000 + (29*3^(1/2)*dq1*dqr1*sin(q3)*sin(q5)*sin(q6))/400 + dq4*dqr1*cos(q3)*cos(q6)*sin(q2)*((1923*3^(1/2))/80000 + 259/16000) + (111*dq4*dqr1*cos(2*q5)*cos(q3)*cos(q6)*sin(q2))/16000 - dq4*dqr1*cos(2*q4)*cos(q3)*cos(q6)*sin(q2)*((1923*3^(1/2))/80000 + 111/3200) + (37*3^(1/2)*dq5*dqr1*cos(q6)*sin(q2)*sin(q3)*sin(q4))/4000 + (37*3^(1/2)*dq6*dqr1*cos(q6)*sin(q2)*sin(q3)*sin(q4))/4000 - (37*dq4*dqr1*cos(2*q4)*cos(2*q5)*cos(q2)*cos(q6)*sin(q3))/3200 + (37*dq4*dqr1*cos(2*q4)*cos(2*q5)*cos(q3)*cos(q6)*sin(q2))/3200 + (37*dq5*dqr1*cos(2*q4)*cos(2*q5)*cos(q3)*cos(q6)*sin(q2))/4000 + (37*dq6*dqr1*cos(2*q4)*cos(2*q5)*cos(q3)*cos(q6)*sin(q2))/4000 - dq6*dqr1*sin(2*q4)*cos(q2)*sin(q3)*sin(q6)*((1923*3^(1/2))/160000 + 111/6400) + dq6*dqr1*sin(2*q4)*cos(q3)*sin(q2)*sin(q6)*((1923*3^(1/2))/160000 + 111/6400) + (37*dq4*dqr1*cos(2*q4)*sin(2*q5)*cos(q2)*sin(q3)*sin(q6))/1600 - (37*dq4*dqr1*cos(2*q4)*sin(2*q5)*cos(q3)*sin(q2)*sin(q6))/1600 + (37*dq4*dqr1*cos(2*q5)*sin(2*q4)*cos(q2)*sin(q3)*sin(q6))/2000 - (37*dq4*dqr1*cos(2*q5)*sin(2*q4)*cos(q3)*sin(q2)*sin(q6))/2000 + (37*dq4*dqr1*sin(2*q4)*sin(2*q5)*cos(q2)*cos(q6)*sin(q3))/4000 - (37*dq4*dqr1*sin(2*q4)*sin(2*q5)*cos(q3)*cos(q6)*sin(q2))/4000 + (37*dq5*dqr1*cos(2*q4)*sin(2*q5)*cos(q2)*sin(q3)*sin(q6))/2000 - (37*dq5*dqr1*cos(2*q4)*sin(2*q5)*cos(q3)*sin(q2)*sin(q6))/2000 + (37*dq5*dqr1*cos(2*q5)*sin(2*q4)*cos(q2)*sin(q3)*sin(q6))/1600 - (37*dq5*dqr1*cos(2*q5)*sin(2*q4)*cos(q3)*sin(q2)*sin(q6))/1600 - (37*dq5*dqr1*sin(2*q4)*sin(2*q5)*cos(q3)*cos(q6)*sin(q2))/3200 + (37*dq6*dqr1*cos(2*q4)*sin(2*q5)*cos(q2)*sin(q3)*sin(q6))/8000 - (37*dq6*dqr1*cos(2*q4)*sin(2*q5)*cos(q3)*sin(q2)*sin(q6))/8000 + (37*dq6*dqr1*cos(2*q5)*sin(2*q4)*cos(q2)*sin(q3)*sin(q6))/6400 - (37*dq6*dqr1*cos(2*q5)*sin(2*q4)*cos(q3)*sin(q2)*sin(q6))/6400 - (37*dq6*dqr1*sin(2*q4)*sin(2*q5)*cos(q3)*cos(q6)*sin(q2))/3200 - (29*3^(1/2)*dq1*dqr1*cos(2*q2)*sin(q3)*sin(q5)*sin(q6))/400 + (877*dq4*dqr1*cos(q4)*cos(q5)*sin(q2)*sin(q3)*sin(q6))/4000 + (1231*dq4*dqr1*cos(q5)*cos(q6)*sin(q2)*sin(q3)*sin(q4))/40000 + (877*dq5*dqr1*cos(q4)*cos(q5)*sin(q2)*sin(q3)*sin(q6))/8000 + (877*dq6*dqr1*cos(q4)*cos(q6)*sin(q2)*sin(q3)*sin(q5))/8000 + (877*dq6*dqr1*cos(q5)*cos(q6)*sin(q2)*sin(q3)*sin(q4))/4000 - (877*dq5*dqr1*sin(q2)*sin(q3)*sin(q4)*sin(q5)*sin(q6))/4000 - (877*dq6*dqr1*sin(q2)*sin(q3)*sin(q4)*sin(q5)*sin(q6))/8000 - dq6*dqr1*cos(q2)*cos(q5)*cos(q6)*sin(q3)*((641*3^(1/2))/40000 + 37/2000) + dq6*dqr1*cos(q3)*cos(q5)*cos(q6)*sin(q2)*((641*3^(1/2))/40000 + 37/2000) - dq4*dqr1*cos(q2)*cos(q5)*cos(q6)*sin(q3)*((641*3^(1/2))/80000 - 37/8000) + dq4*dqr1*cos(q3)*cos(q5)*cos(q6)*sin(q2)*((641*3^(1/2))/80000 - 37/8000) - dq5*dqr1*cos(q2)*cos(q5)*cos(q6)*sin(q3)*((641*3^(1/2))/80000 - 37/8000) + dq5*dqr1*cos(q3)*cos(q5)*cos(q6)*sin(q2)*((641*3^(1/2))/80000 - 37/8000) + dq6*dqr1*cos(q4)*sin(q2)*sin(q3)*sin(q6)*((37*3^(1/2))/16000 + 2631/16000) + dq4*dqr1*cos(q2)*sin(q3)*sin(q5)*sin(q6)*((641*3^(1/2))/40000 + 37/2000) - dq4*dqr1*cos(q3)*sin(q2)*sin(q5)*sin(q6)*((641*3^(1/2))/40000 + 37/2000) + dq5*dqr1*cos(q2)*sin(q3)*sin(q5)*sin(q6)*((641*3^(1/2))/40000 + 37/2000) - dq5*dqr1*cos(q3)*sin(q2)*sin(q5)*sin(q6)*((641*3^(1/2))/40000 + 37/2000) + dq4*dqr1*cos(q6)*sin(q2)*sin(q3)*sin(q4)*((111*3^(1/2))/8000 + 7539/40000) + dq6*dqr1*cos(q2)*sin(q3)*sin(q5)*sin(q6)*((641*3^(1/2))/80000 + 37/1600) - dq6*dqr1*cos(q3)*sin(q2)*sin(q5)*sin(q6)*((641*3^(1/2))/80000 + 37/1600) - (29*dq1*dqr1*sin(2*q2)*cos(q4)*cos(q5)*sin(q3)*sin(q6))/200 - (29*dq1*dqr1*sin(2*q2)*cos(q4)*cos(q6)*sin(q3)*sin(q5))/400 - (29*dq1*dqr1*sin(2*q2)*cos(q5)*cos(q6)*sin(q3)*sin(q4))/800 + (29*dq1*dqr1*sin(2*q2)*sin(q3)*sin(q4)*sin(q5)*sin(q6))/400 + (37*3^(1/2)*dq4*dqr1*cos(2*q5)*cos(q4)*sin(q2)*sin(q3)*sin(q6))/2000 + (37*3^(1/2)*dq4*dqr1*cos(2*q5)*cos(q6)*sin(q2)*sin(q3)*sin(q4))/8000 + (37*3^(1/2)*dq4*dqr1*sin(2*q5)*cos(q4)*cos(q6)*sin(q2)*sin(q3))/4000 + (37*3^(1/2)*dq5*dqr1*cos(2*q5)*cos(q4)*sin(q2)*sin(q3)*sin(q6))/4000 + (37*3^(1/2)*dq5*dqr1*cos(2*q5)*cos(q6)*sin(q2)*sin(q3)*sin(q4))/4000 + (37*3^(1/2)*dq5*dqr1*sin(2*q5)*cos(q4)*cos(q6)*sin(q2)*sin(q3))/8000 + (37*3^(1/2)*dq6*dqr1*cos(2*q5)*cos(q4)*sin(q2)*sin(q3)*sin(q6))/16000 + (37*3^(1/2)*dq6*dqr1*cos(2*q5)*cos(q6)*sin(q2)*sin(q3)*sin(q4))/4000 + (37*3^(1/2)*dq6*dqr1*sin(2*q5)*cos(q4)*cos(q6)*sin(q2)*sin(q3))/8000 - (37*3^(1/2)*dq4*dqr1*sin(2*q5)*sin(q2)*sin(q3)*sin(q4)*sin(q6))/4000 - (37*3^(1/2)*dq5*dqr1*sin(2*q5)*sin(q2)*sin(q3)*sin(q4)*sin(q6))/2000 - (37*3^(1/2)*dq6*dqr1*sin(2*q5)*sin(q2)*sin(q3)*sin(q4)*sin(q6))/8000 - dq4*dqr1*cos(q4)*cos(q6)*sin(q2)*sin(q3)*sin(q5)*((37*3^(1/2))/4000 - 877/8000) - dq5*dqr1*cos(q5)*cos(q6)*sin(q2)*sin(q3)*sin(q4)*((37*3^(1/2))/4000 - 877/8000) - dq5*dqr1*cos(q4)*cos(q6)*sin(q2)*sin(q3)*sin(q5)*((37*3^(1/2))/8000 - 877/16000) + dq6*dqr1*cos(q4)*cos(q5)*sin(q2)*sin(q3)*sin(q6)*((111*3^(1/2))/8000 + 877/16000) + dq4*dqr1*sin(q2)*sin(q3)*sin(q4)*sin(q5)*sin(q6)*((37*3^(1/2))/2000 - 1231/20000) + dq6*dqr1*cos(2*q4)*cos(q2)*cos(q5)*cos(q6)*sin(q3)*((641*3^(1/2))/40000 + 37/2000) - dq6*dqr1*cos(2*q4)*cos(q3)*cos(q5)*cos(q6)*sin(q2)*((641*3^(1/2))/40000 + 37/2000) + dq4*dqr1*cos(2*q4)*cos(q2)*cos(q5)*cos(q6)*sin(q3)*((641*3^(1/2))/80000 - 37/8000) - dq4*dqr1*cos(2*q4)*cos(q3)*cos(q5)*cos(q6)*sin(q2)*((641*3^(1/2))/80000 - 37/8000) + dq5*dqr1*cos(2*q4)*cos(q2)*cos(q5)*cos(q6)*sin(q3)*((641*3^(1/2))/80000 - 37/8000) - dq5*dqr1*cos(2*q4)*cos(q3)*cos(q5)*cos(q6)*sin(q2)*((641*3^(1/2))/80000 - 37/8000) - dq4*dqr1*sin(2*q4)*cos(q2)*cos(q5)*sin(q3)*sin(q6)*((641*3^(1/2))/20000 + 37/1000) + dq4*dqr1*sin(2*q4)*cos(q3)*cos(q5)*sin(q2)*sin(q6)*((641*3^(1/2))/20000 + 37/1000) - dq4*dqr1*cos(2*q4)*cos(q2)*sin(q3)*sin(q5)*sin(q6)*((641*3^(1/2))/40000 + 37/2000) + dq4*dqr1*cos(2*q4)*cos(q3)*sin(q2)*sin(q5)*sin(q6)*((641*3^(1/2))/40000 + 37/2000) - dq5*dqr1*cos(2*q4)*cos(q2)*sin(q3)*sin(q5)*sin(q6)*((641*3^(1/2))/40000 + 37/2000) + dq5*dqr1*cos(2*q4)*cos(q3)*sin(q2)*sin(q5)*sin(q6)*((641*3^(1/2))/40000 + 37/2000) - dq4*dqr1*sin(2*q4)*cos(q2)*cos(q6)*sin(q3)*sin(q5)*((641*3^(1/2))/40000 - 37/4000) + dq4*dqr1*sin(2*q4)*cos(q3)*cos(q6)*sin(q2)*sin(q5)*((641*3^(1/2))/40000 - 37/4000) - dq5*dqr1*sin(2*q4)*cos(q2)*cos(q5)*sin(q3)*sin(q6)*((641*3^(1/2))/80000 + 37/4000) + dq5*dqr1*sin(2*q4)*cos(q3)*cos(q5)*sin(q2)*sin(q6)*((641*3^(1/2))/80000 + 37/4000) - dq6*dqr1*sin(2*q4)*cos(q2)*cos(q6)*sin(q3)*sin(q5)*((641*3^(1/2))/80000 + 37/4000) + dq6*dqr1*sin(2*q4)*cos(q3)*cos(q6)*sin(q2)*sin(q5)*((641*3^(1/2))/80000 + 37/4000) - dq6*dqr1*cos(2*q4)*cos(q2)*sin(q3)*sin(q5)*sin(q6)*((641*3^(1/2))/80000 - 37/8000) + dq6*dqr1*cos(2*q4)*cos(q3)*sin(q2)*sin(q5)*sin(q6)*((641*3^(1/2))/80000 - 37/8000) - dq5*dqr1*sin(2*q4)*cos(q2)*cos(q6)*sin(q3)*sin(q5)*((641*3^(1/2))/160000 - 37/16000) + dq5*dqr1*sin(2*q4)*cos(q3)*cos(q6)*sin(q2)*sin(q5)*((641*3^(1/2))/160000 - 37/16000) - dq6*dqr1*sin(2*q4)*cos(q2)*cos(q5)*sin(q3)*sin(q6)*((641*3^(1/2))/160000 - 37/16000) + dq6*dqr1*sin(2*q4)*cos(q3)*cos(q5)*sin(q2)*sin(q6)*((641*3^(1/2))/160000 - 37/16000);
Y3_10_2=(29*3^(1/2)*dq1*dqr1*cos(q6)*sin(q3))/800 + (87*dq1*dqr1*cos(q3)*cos(q6)*sin(q4))/800 + (37*dq5*dqr1*cos(q2)*cos(q6)*sin(q3))/4000 + (37*dq6*dqr1*cos(q2)*cos(q6)*sin(q3))/4000 - (29*3^(1/2)*dq1*dqr1*cos(q5)*cos(q6)*sin(q3))/800 - (29*3^(1/2)*dq1*dqr1*cos(2*q2)*cos(q6)*sin(q3))/800 + (29*3^(1/2)*dq1*dqr1*sin(2*q2)*cos(q3)*cos(q6))/800 + (29*dq1*dqr1*cos(q3)*cos(q4)*cos(q5)*sin(q6))/200 + (29*dq1*dqr1*cos(q3)*cos(q4)*cos(q6)*sin(q5))/400 + (29*dq1*dqr1*cos(q3)*cos(q5)*cos(q6)*sin(q4))/800 + dq1*dqr1*cos(2*q2)*sin(2*q3)*cos(q6)*((6847*3^(1/2))/160000 - 481/32000) - dq1*dqr1*cos(2*q3)*sin(2*q2)*cos(q6)*((6847*3^(1/2))/160000 - 481/32000) - (333*dq1*dqr1*cos(2*q2)*cos(2*q5)*sin(2*q3)*cos(q6))/32000 + (333*dq1*dqr1*cos(2*q3)*cos(2*q5)*sin(2*q2)*cos(q6))/32000 - (29*dq1*dqr1*cos(q3)*sin(q4)*sin(q5)*sin(q6))/400 + (333*dq1*dqr1*cos(2*q2)*sin(2*q3)*sin(2*q5)*sin(q6))/16000 - (333*dq1*dqr1*cos(2*q3)*sin(2*q2)*sin(2*q5)*sin(q6))/16000 - dq4*dqr1*cos(q2)*cos(q6)*sin(q3)*((1923*3^(1/2))/80000 + 259/16000) - (87*dq1*dqr1*cos(2*q2)*cos(q3)*cos(q6)*sin(q4))/800 - (111*dq4*dqr1*cos(2*q5)*cos(q2)*cos(q6)*sin(q3))/16000 + dq4*dqr1*cos(2*q4)*cos(q2)*cos(q6)*sin(q3)*((1923*3^(1/2))/80000 + 111/3200) + (877*dq1*dqr1*cos(2*q2)*cos(2*q3)*cos(q4)*cos(q5)*sin(q6))/4000 + (1231*dq1*dqr1*cos(2*q2)*cos(2*q3)*cos(q5)*cos(q6)*sin(q4))/40000 - (37*dq5*dqr1*cos(2*q4)*cos(2*q5)*cos(q2)*cos(q6)*sin(q3))/4000 - (37*dq6*dqr1*cos(2*q4)*cos(2*q5)*cos(q2)*cos(q6)*sin(q3))/4000 + (877*dq1*dqr1*sin(2*q2)*sin(2*q3)*cos(q4)*cos(q5)*sin(q6))/4000 + (1231*dq1*dqr1*sin(2*q2)*sin(2*q3)*cos(q5)*cos(q6)*sin(q4))/40000 + (37*dq5*dqr1*sin(2*q4)*sin(2*q5)*cos(q2)*cos(q6)*sin(q3))/3200 + (37*dq6*dqr1*sin(2*q4)*sin(2*q5)*cos(q2)*cos(q6)*sin(q3))/3200 + (29*3^(1/2)*dq1*dqr1*cos(2*q2)*cos(q5)*cos(q6)*sin(q3))/800 - (29*3^(1/2)*dq1*dqr1*sin(2*q2)*cos(q3)*cos(q5)*cos(q6))/800 + (877*dq4*dqr1*cos(q2)*cos(q3)*cos(q4)*cos(q5)*sin(q6))/4000 + (1231*dq4*dqr1*cos(q2)*cos(q3)*cos(q5)*cos(q6)*sin(q4))/40000 + (877*dq5*dqr1*cos(q2)*cos(q3)*cos(q4)*cos(q5)*sin(q6))/8000 + (877*dq6*dqr1*cos(q2)*cos(q3)*cos(q4)*cos(q6)*sin(q5))/8000 + (877*dq6*dqr1*cos(q2)*cos(q3)*cos(q5)*cos(q6)*sin(q4))/4000 + dq1*dqr1*cos(2*q2)*cos(2*q3)*cos(q6)*sin(q4)*((111*3^(1/2))/8000 + 7539/40000) - dq1*dqr1*cos(2*q2)*sin(2*q3)*cos(q5)*cos(q6)*((9411*3^(1/2))/160000 - 259/16000) + dq1*dqr1*cos(2*q3)*sin(2*q2)*cos(q5)*cos(q6)*((9411*3^(1/2))/160000 - 259/16000) + (29*3^(1/2)*dq1*dqr1*sin(2*q2)*cos(q3)*sin(q5)*sin(q6))/400 - (877*dq5*dqr1*cos(q2)*cos(q3)*sin(q4)*sin(q5)*sin(q6))/4000 - (877*dq6*dqr1*cos(q2)*cos(q3)*sin(q4)*sin(q5)*sin(q6))/8000 + dq1*dqr1*sin(2*q2)*sin(2*q3)*cos(q6)*sin(q4)*((111*3^(1/2))/8000 + 7539/40000) + dq1*dqr1*cos(2*q2)*sin(2*q3)*sin(q5)*sin(q6)*((9411*3^(1/2))/80000 + 37/4000) - dq1*dqr1*cos(2*q3)*sin(2*q2)*sin(q5)*sin(q6)*((9411*3^(1/2))/80000 + 37/4000) + dq6*dqr1*cos(q2)*cos(q3)*cos(q4)*sin(q6)*((37*3^(1/2))/16000 + 2631/16000) + dq4*dqr1*cos(q2)*cos(q3)*cos(q6)*sin(q4)*((111*3^(1/2))/8000 + 7539/40000) - (29*dq1*dqr1*cos(2*q2)*cos(q3)*cos(q4)*cos(q5)*sin(q6))/200 - (29*dq1*dqr1*cos(2*q2)*cos(q3)*cos(q4)*cos(q6)*sin(q5))/400 - (29*dq1*dqr1*cos(2*q2)*cos(q3)*cos(q5)*cos(q6)*sin(q4))/800 + dq1*dqr1*cos(2*q2)*cos(2*q4)*sin(2*q3)*cos(q6)*((1923*3^(1/2))/160000 + 111/6400) - dq1*dqr1*cos(2*q3)*cos(2*q4)*sin(2*q2)*cos(q6)*((1923*3^(1/2))/160000 + 111/6400) - (37*dq1*dqr1*cos(2*q2)*cos(2*q4)*cos(2*q5)*sin(2*q3)*cos(q6))/6400 + (37*dq1*dqr1*cos(2*q3)*cos(2*q4)*cos(2*q5)*sin(2*q2)*cos(q6))/6400 + (29*dq1*dqr1*cos(2*q2)*cos(q3)*sin(q4)*sin(q5)*sin(q6))/400 + (37*3^(1/2)*dq5*dqr1*cos(q2)*cos(q3)*cos(q6)*sin(q4))/4000 + (37*3^(1/2)*dq6*dqr1*cos(q2)*cos(q3)*cos(q6)*sin(q4))/4000 + (37*dq1*dqr1*cos(2*q2)*cos(2*q4)*sin(2*q3)*sin(2*q5)*sin(q6))/3200 + (37*dq1*dqr1*cos(2*q2)*cos(2*q5)*sin(2*q3)*sin(2*q4)*sin(q6))/4000 + (37*dq1*dqr1*cos(2*q2)*sin(2*q3)*sin(2*q4)*sin(2*q5)*cos(q6))/8000 - (37*dq1*dqr1*cos(2*q3)*cos(2*q4)*sin(2*q2)*sin(2*q5)*sin(q6))/3200 - (37*dq1*dqr1*cos(2*q3)*cos(2*q5)*sin(2*q2)*sin(2*q4)*sin(q6))/4000 - (37*dq1*dqr1*cos(2*q3)*sin(2*q2)*sin(2*q4)*sin(2*q5)*cos(q6))/8000 - (37*3^(1/2)*dq1*dqr1*sin(2*q2)*sin(2*q3)*sin(2*q5)*sin(q4)*sin(q6))/4000 + (37*3^(1/2)*dq4*dqr1*cos(2*q5)*cos(q2)*cos(q3)*cos(q4)*sin(q6))/2000 + (37*3^(1/2)*dq4*dqr1*cos(2*q5)*cos(q2)*cos(q3)*cos(q6)*sin(q4))/8000 + (37*3^(1/2)*dq4*dqr1*sin(2*q5)*cos(q2)*cos(q3)*cos(q4)*cos(q6))/4000 + (37*3^(1/2)*dq5*dqr1*cos(2*q5)*cos(q2)*cos(q3)*cos(q4)*sin(q6))/4000 + (37*3^(1/2)*dq5*dqr1*cos(2*q5)*cos(q2)*cos(q3)*cos(q6)*sin(q4))/4000 + (37*3^(1/2)*dq5*dqr1*sin(2*q5)*cos(q2)*cos(q3)*cos(q4)*cos(q6))/8000 + (37*3^(1/2)*dq6*dqr1*cos(2*q5)*cos(q2)*cos(q3)*cos(q4)*sin(q6))/16000 + (37*3^(1/2)*dq6*dqr1*cos(2*q5)*cos(q2)*cos(q3)*cos(q6)*sin(q4))/4000 + (37*3^(1/2)*dq6*dqr1*sin(2*q5)*cos(q2)*cos(q3)*cos(q4)*cos(q6))/8000 - dq1*dqr1*cos(2*q2)*cos(2*q3)*cos(q4)*cos(q6)*sin(q5)*((37*3^(1/2))/4000 - 877/8000) - (37*3^(1/2)*dq4*dqr1*sin(2*q5)*cos(q2)*cos(q3)*sin(q4)*sin(q6))/4000 - (37*3^(1/2)*dq5*dqr1*sin(2*q5)*cos(q2)*cos(q3)*sin(q4)*sin(q6))/2000 - (37*3^(1/2)*dq6*dqr1*sin(2*q5)*cos(q2)*cos(q3)*sin(q4)*sin(q6))/8000 - dq1*dqr1*sin(2*q2)*sin(2*q3)*cos(q4)*cos(q6)*sin(q5)*((37*3^(1/2))/4000 - 877/8000) + dq1*dqr1*cos(2*q2)*cos(2*q3)*sin(q4)*sin(q5)*sin(q6)*((37*3^(1/2))/2000 - 1231/20000) + dq1*dqr1*sin(2*q2)*sin(2*q3)*sin(q4)*sin(q5)*sin(q6)*((37*3^(1/2))/2000 - 1231/20000) - dq4*dqr1*cos(q2)*cos(q3)*cos(q4)*cos(q6)*sin(q5)*((37*3^(1/2))/4000 - 877/8000) - dq5*dqr1*cos(q2)*cos(q3)*cos(q5)*cos(q6)*sin(q4)*((37*3^(1/2))/4000 - 877/8000) - dq5*dqr1*cos(q2)*cos(q3)*cos(q4)*cos(q6)*sin(q5)*((37*3^(1/2))/8000 - 877/16000) + dq6*dqr1*cos(q2)*cos(q3)*cos(q4)*cos(q5)*sin(q6)*((111*3^(1/2))/8000 + 877/16000) + dq1*dqr1*cos(2*q2)*cos(2*q4)*sin(2*q3)*cos(q5)*cos(q6)*((641*3^(1/2))/160000 - 37/16000) - dq1*dqr1*cos(2*q3)*cos(2*q4)*sin(2*q2)*cos(q5)*cos(q6)*((641*3^(1/2))/160000 - 37/16000) + dq4*dqr1*cos(q2)*cos(q3)*sin(q4)*sin(q5)*sin(q6)*((37*3^(1/2))/2000 - 1231/20000) - dq1*dqr1*cos(2*q2)*sin(2*q3)*sin(2*q4)*cos(q5)*sin(q6)*((641*3^(1/2))/40000 + 37/2000) + dq1*dqr1*cos(2*q3)*sin(2*q2)*sin(2*q4)*cos(q5)*sin(q6)*((641*3^(1/2))/40000 + 37/2000) - dq1*dqr1*cos(2*q2)*cos(2*q4)*sin(2*q3)*sin(q5)*sin(q6)*((641*3^(1/2))/80000 + 37/4000) + dq1*dqr1*cos(2*q3)*cos(2*q4)*sin(2*q2)*sin(q5)*sin(q6)*((641*3^(1/2))/80000 + 37/4000) - dq1*dqr1*cos(2*q2)*sin(2*q3)*sin(2*q4)*cos(q6)*sin(q5)*((641*3^(1/2))/80000 - 37/8000) + dq1*dqr1*cos(2*q3)*sin(2*q2)*sin(2*q4)*cos(q6)*sin(q5)*((641*3^(1/2))/80000 - 37/8000) + (37*3^(1/2)*dq1*dqr1*cos(2*q2)*cos(2*q3)*cos(2*q5)*cos(q4)*sin(q6))/2000 + (37*3^(1/2)*dq1*dqr1*cos(2*q2)*cos(2*q3)*cos(2*q5)*cos(q6)*sin(q4))/8000 + (37*3^(1/2)*dq1*dqr1*cos(2*q2)*cos(2*q3)*sin(2*q5)*cos(q4)*cos(q6))/4000 - (37*3^(1/2)*dq1*dqr1*cos(2*q2)*cos(2*q3)*sin(2*q5)*sin(q4)*sin(q6))/4000 + (37*3^(1/2)*dq1*dqr1*cos(2*q5)*sin(2*q2)*sin(2*q3)*cos(q4)*sin(q6))/2000 + (37*3^(1/2)*dq1*dqr1*cos(2*q5)*sin(2*q2)*sin(2*q3)*cos(q6)*sin(q4))/8000 + (37*3^(1/2)*dq1*dqr1*sin(2*q2)*sin(2*q3)*sin(2*q5)*cos(q4)*cos(q6))/4000;
Y3_10_3=dq6*dqr3*sin(q6)*((10693*3^(1/2))/160000 + 37/32000) - dq6*dqr2*sin(q6)*((10693*3^(1/2))/160000 + 37/32000) + (111*dq5*dqr2*cos(2*q5)*sin(q6))/8000 + (111*dq5*dqr2*sin(2*q5)*cos(q6))/16000 - (111*dq5*dqr3*cos(2*q5)*sin(q6))/8000 - (111*dq5*dqr3*sin(2*q5)*cos(q6))/16000 + (111*dq6*dqr2*cos(2*q5)*sin(q6))/32000 + (111*dq6*dqr2*sin(2*q5)*cos(q6))/16000 - (111*dq6*dqr3*cos(2*q5)*sin(q6))/32000 - (111*dq6*dqr3*sin(2*q5)*cos(q6))/16000 + (29*3^(1/2)*dq2*dqr2*cos(q6)*sin(q3))/400 + dq4*dqr2*sin(2*q4)*cos(q6)*((1923*3^(1/2))/80000 + 111/3200) - dq4*dqr3*sin(2*q4)*cos(q6)*((1923*3^(1/2))/80000 + 111/3200) + dq6*dqr2*cos(2*q4)*sin(q6)*((1923*3^(1/2))/160000 + 111/6400) - dq6*dqr3*cos(2*q4)*sin(q6)*((1923*3^(1/2))/160000 + 111/6400) - (37*dq4*dqr2*cos(2*q4)*cos(2*q5)*sin(q6))/2000 - (37*dq4*dqr2*cos(2*q4)*sin(2*q5)*cos(q6))/4000 - (37*dq4*dqr2*cos(2*q5)*sin(2*q4)*cos(q6))/3200 + (37*dq4*dqr3*cos(2*q4)*cos(2*q5)*sin(q6))/2000 + (37*dq4*dqr3*cos(2*q4)*sin(2*q5)*cos(q6))/4000 + (37*dq4*dqr3*cos(2*q5)*sin(2*q4)*cos(q6))/3200 - (37*dq5*dqr2*cos(2*q4)*cos(2*q5)*sin(q6))/1600 - (37*dq5*dqr2*cos(2*q4)*sin(2*q5)*cos(q6))/3200 - (37*dq5*dqr2*cos(2*q5)*sin(2*q4)*cos(q6))/4000 + (37*dq5*dqr3*cos(2*q4)*cos(2*q5)*sin(q6))/1600 + (37*dq5*dqr3*cos(2*q4)*sin(2*q5)*cos(q6))/3200 + (37*dq5*dqr3*cos(2*q5)*sin(2*q4)*cos(q6))/4000 - (37*dq6*dqr2*cos(2*q4)*cos(2*q5)*sin(q6))/6400 - (37*dq6*dqr2*cos(2*q4)*sin(2*q5)*cos(q6))/3200 - (37*dq6*dqr2*cos(2*q5)*sin(2*q4)*cos(q6))/4000 + (37*dq6*dqr3*cos(2*q4)*cos(2*q5)*sin(q6))/6400 + (37*dq6*dqr3*cos(2*q4)*sin(2*q5)*cos(q6))/3200 + (37*dq6*dqr3*cos(2*q5)*sin(2*q4)*cos(q6))/4000 + (37*dq4*dqr2*sin(2*q4)*sin(2*q5)*sin(q6))/1600 - (37*dq4*dqr3*sin(2*q4)*sin(2*q5)*sin(q6))/1600 + (37*dq5*dqr2*sin(2*q4)*sin(2*q5)*sin(q6))/2000 - (37*dq5*dqr3*sin(2*q4)*sin(2*q5)*sin(q6))/2000 + (37*dq6*dqr2*sin(2*q4)*sin(2*q5)*sin(q6))/8000 - (37*dq6*dqr3*sin(2*q4)*sin(2*q5)*sin(q6))/8000 + (87*dq2*dqr2*cos(q3)*cos(q6)*sin(q4))/400 + dq5*dqr2*cos(q5)*sin(q6)*((8129*3^(1/2))/80000 - 37/4000) - dq5*dqr3*cos(q5)*sin(q6)*((8129*3^(1/2))/80000 - 37/4000) + dq6*dqr2*cos(q6)*sin(q5)*((8129*3^(1/2))/80000 - 37/4000) - dq6*dqr3*cos(q6)*sin(q5)*((8129*3^(1/2))/80000 - 37/4000) + dq5*dqr2*cos(q6)*sin(q5)*((8129*3^(1/2))/160000 - 37/3200) - dq5*dqr3*cos(q6)*sin(q5)*((8129*3^(1/2))/160000 - 37/3200) + dq6*dqr2*cos(q5)*sin(q6)*((8129*3^(1/2))/160000 - 37/3200) - dq6*dqr3*cos(q5)*sin(q6)*((8129*3^(1/2))/160000 - 37/3200) - (111*dq1*dqr4*sin(2*q5)*cos(q3)*sin(q2)*sin(q6))/8000 - (29*3^(1/2)*dq2*dqr2*cos(q5)*cos(q6)*sin(q3))/400 + dq4*dqr2*cos(2*q4)*cos(q5)*sin(q6)*((641*3^(1/2))/20000 + 37/1000) - dq4*dqr3*cos(2*q4)*cos(q5)*sin(q6)*((641*3^(1/2))/20000 + 37/1000) + dq6*dqr2*sin(2*q4)*cos(q5)*cos(q6)*((641*3^(1/2))/40000 + 37/2000) - dq6*dqr3*sin(2*q4)*cos(q5)*cos(q6)*((641*3^(1/2))/40000 + 37/2000) + dq4*dqr2*cos(2*q4)*cos(q6)*sin(q5)*((641*3^(1/2))/40000 - 37/4000) - dq4*dqr3*cos(2*q4)*cos(q6)*sin(q5)*((641*3^(1/2))/40000 - 37/4000) + dq5*dqr2*cos(2*q4)*cos(q5)*sin(q6)*((641*3^(1/2))/80000 + 37/4000) - dq5*dqr3*cos(2*q4)*cos(q5)*sin(q6)*((641*3^(1/2))/80000 + 37/4000) + dq6*dqr2*cos(2*q4)*cos(q6)*sin(q5)*((641*3^(1/2))/80000 + 37/4000) - dq6*dqr3*cos(2*q4)*cos(q6)*sin(q5)*((641*3^(1/2))/80000 + 37/4000) + dq4*dqr2*sin(2*q4)*cos(q5)*cos(q6)*((641*3^(1/2))/80000 - 37/8000) - dq4*dqr3*sin(2*q4)*cos(q5)*cos(q6)*((641*3^(1/2))/80000 - 37/8000) + dq5*dqr2*sin(2*q4)*cos(q5)*cos(q6)*((641*3^(1/2))/80000 - 37/8000) - dq5*dqr3*sin(2*q4)*cos(q5)*cos(q6)*((641*3^(1/2))/80000 - 37/8000) + dq5*dqr2*cos(2*q4)*cos(q6)*sin(q5)*((641*3^(1/2))/160000 - 37/16000) - dq5*dqr3*cos(2*q4)*cos(q6)*sin(q5)*((641*3^(1/2))/160000 - 37/16000) + dq6*dqr2*cos(2*q4)*cos(q5)*sin(q6)*((641*3^(1/2))/160000 - 37/16000) - dq6*dqr3*cos(2*q4)*cos(q5)*sin(q6)*((641*3^(1/2))/160000 - 37/16000) + (29*3^(1/2)*dq2*dqr2*sin(q3)*sin(q5)*sin(q6))/200 - dq4*dqr2*sin(2*q4)*sin(q5)*sin(q6)*((641*3^(1/2))/40000 + 37/2000) + dq4*dqr3*sin(2*q4)*sin(q5)*sin(q6)*((641*3^(1/2))/40000 + 37/2000) - dq5*dqr2*sin(2*q4)*sin(q5)*sin(q6)*((641*3^(1/2))/40000 + 37/2000) + dq5*dqr3*sin(2*q4)*sin(q5)*sin(q6)*((641*3^(1/2))/40000 + 37/2000) - dq6*dqr2*sin(2*q4)*sin(q5)*sin(q6)*((641*3^(1/2))/80000 - 37/8000) + dq6*dqr3*sin(2*q4)*sin(q5)*sin(q6)*((641*3^(1/2))/80000 - 37/8000) + (29*dq2*dqr2*cos(q3)*cos(q4)*cos(q5)*sin(q6))/100 + (29*dq2*dqr2*cos(q3)*cos(q4)*cos(q6)*sin(q5))/200 + (29*dq2*dqr2*cos(q3)*cos(q5)*cos(q6)*sin(q4))/400 - (29*dq2*dqr2*cos(q3)*sin(q4)*sin(q5)*sin(q6))/200 + (111*dq1*dqr4*cos(2*q5)*cos(q3)*cos(q6)*sin(q2))/16000 - dq1*dqr4*cos(2*q4)*cos(q3)*cos(q6)*sin(q2)*((1923*3^(1/2))/80000 + 111/3200) + (37*dq1*dqr4*cos(2*q4)*cos(2*q5)*cos(q3)*cos(q6)*sin(q2))/3200 - (37*dq1*dqr4*cos(2*q4)*sin(2*q5)*cos(q3)*sin(q2)*sin(q6))/1600 - (37*dq1*dqr4*cos(2*q5)*sin(2*q4)*cos(q3)*sin(q2)*sin(q6))/2000 - (37*dq1*dqr4*sin(2*q4)*sin(2*q5)*cos(q3)*cos(q6)*sin(q2))/4000 + (877*dq1*dqr4*cos(q4)*cos(q5)*sin(q2)*sin(q3)*sin(q6))/4000 + (1231*dq1*dqr4*cos(q5)*cos(q6)*sin(q2)*sin(q3)*sin(q4))/40000 + dq1*dqr4*cos(q3)*cos(q5)*cos(q6)*sin(q2)*((641*3^(1/2))/80000 - 37/8000) - dq1*dqr4*cos(q3)*sin(q2)*sin(q5)*sin(q6)*((641*3^(1/2))/40000 + 37/2000) + dq1*dqr4*cos(q6)*sin(q2)*sin(q3)*sin(q4)*((111*3^(1/2))/8000 + 7539/40000) + (37*3^(1/2)*dq1*dqr4*cos(2*q5)*cos(q4)*sin(q2)*sin(q3)*sin(q6))/2000 + (37*3^(1/2)*dq1*dqr4*cos(2*q5)*cos(q6)*sin(q2)*sin(q3)*sin(q4))/8000 + (37*3^(1/2)*dq1*dqr4*sin(2*q5)*cos(q4)*cos(q6)*sin(q2)*sin(q3))/4000 - (37*3^(1/2)*dq1*dqr4*sin(2*q5)*sin(q2)*sin(q3)*sin(q4)*sin(q6))/4000 - dq1*dqr4*cos(q4)*cos(q6)*sin(q2)*sin(q3)*sin(q5)*((37*3^(1/2))/4000 - 877/8000) + dq1*dqr4*sin(q2)*sin(q3)*sin(q4)*sin(q5)*sin(q6)*((37*3^(1/2))/2000 - 1231/20000) - dq1*dqr4*cos(2*q4)*cos(q3)*cos(q5)*cos(q6)*sin(q2)*((641*3^(1/2))/80000 - 37/8000) + dq1*dqr4*sin(2*q4)*cos(q3)*cos(q5)*sin(q2)*sin(q6)*((641*3^(1/2))/20000 + 37/1000) + dq1*dqr4*cos(2*q4)*cos(q3)*sin(q2)*sin(q5)*sin(q6)*((641*3^(1/2))/40000 + 37/2000) + dq1*dqr4*sin(2*q4)*cos(q3)*cos(q6)*sin(q2)*sin(q5)*((641*3^(1/2))/40000 - 37/4000);
Y3_10_4=(37*3^(1/2)*dq5*dqr4*cos(q6)*sin(q4))/4000 + (37*3^(1/2)*dq6*dqr4*cos(q6)*sin(q4))/4000 + dq2*dqr4*sin(2*q4)*cos(q6)*((1923*3^(1/2))/80000 + 111/3200) - dq3*dqr4*sin(2*q4)*cos(q6)*((1923*3^(1/2))/80000 + 111/3200) - (37*dq2*dqr4*cos(2*q4)*cos(2*q5)*sin(q6))/2000 - (37*dq2*dqr4*cos(2*q4)*sin(2*q5)*cos(q6))/4000 - (37*dq2*dqr4*cos(2*q5)*sin(2*q4)*cos(q6))/3200 + (37*dq3*dqr4*cos(2*q4)*cos(2*q5)*sin(q6))/2000 + (37*dq3*dqr4*cos(2*q4)*sin(2*q5)*cos(q6))/4000 + (37*dq3*dqr4*cos(2*q5)*sin(2*q4)*cos(q6))/3200 + (37*dq2*dqr4*sin(2*q4)*sin(2*q5)*sin(q6))/1600 - (37*dq3*dqr4*sin(2*q4)*sin(2*q5)*sin(q6))/1600 - (37*dq1*dqr5*cos(q3)*cos(q6)*sin(q2))/4000 + (877*dq4*dqr4*cos(q4)*cos(q5)*sin(q6))/4000 + (1231*dq4*dqr4*cos(q5)*cos(q6)*sin(q4))/40000 + (877*dq5*dqr4*cos(q4)*cos(q5)*sin(q6))/8000 + (877*dq6*dqr4*cos(q4)*cos(q6)*sin(q5))/8000 + (877*dq6*dqr4*cos(q5)*cos(q6)*sin(q4))/4000 - (877*dq5*dqr4*sin(q4)*sin(q5)*sin(q6))/4000 - (877*dq6*dqr4*sin(q4)*sin(q5)*sin(q6))/8000 + dq6*dqr4*cos(q4)*sin(q6)*((37*3^(1/2))/16000 + 2631/16000) + dq4*dqr4*cos(q6)*sin(q4)*((111*3^(1/2))/8000 + 7539/40000) + (111*dq1*dqr4*sin(2*q5)*cos(q2)*sin(q3)*sin(q6))/8000 + dq2*dqr4*cos(2*q4)*cos(q5)*sin(q6)*((641*3^(1/2))/20000 + 37/1000) - dq3*dqr4*cos(2*q4)*cos(q5)*sin(q6)*((641*3^(1/2))/20000 + 37/1000) + dq2*dqr4*cos(2*q4)*cos(q6)*sin(q5)*((641*3^(1/2))/40000 - 37/4000) - dq3*dqr4*cos(2*q4)*cos(q6)*sin(q5)*((641*3^(1/2))/40000 - 37/4000) + dq2*dqr4*sin(2*q4)*cos(q5)*cos(q6)*((641*3^(1/2))/80000 - 37/8000) - dq3*dqr4*sin(2*q4)*cos(q5)*cos(q6)*((641*3^(1/2))/80000 - 37/8000) - dq2*dqr4*sin(2*q4)*sin(q5)*sin(q6)*((641*3^(1/2))/40000 + 37/2000) + dq3*dqr4*sin(2*q4)*sin(q5)*sin(q6)*((641*3^(1/2))/40000 + 37/2000) + (37*3^(1/2)*dq4*dqr4*cos(2*q5)*cos(q4)*sin(q6))/2000 + (37*3^(1/2)*dq4*dqr4*cos(2*q5)*cos(q6)*sin(q4))/8000 + (37*3^(1/2)*dq4*dqr4*sin(2*q5)*cos(q4)*cos(q6))/4000 + (37*3^(1/2)*dq5*dqr4*cos(2*q5)*cos(q4)*sin(q6))/4000 + (37*3^(1/2)*dq5*dqr4*cos(2*q5)*cos(q6)*sin(q4))/4000 + (37*3^(1/2)*dq5*dqr4*sin(2*q5)*cos(q4)*cos(q6))/8000 + (37*3^(1/2)*dq6*dqr4*cos(2*q5)*cos(q4)*sin(q6))/16000 + (37*3^(1/2)*dq6*dqr4*cos(2*q5)*cos(q6)*sin(q4))/4000 + (37*3^(1/2)*dq6*dqr4*sin(2*q5)*cos(q4)*cos(q6))/8000 - (37*3^(1/2)*dq4*dqr4*sin(2*q5)*sin(q4)*sin(q6))/4000 - (37*3^(1/2)*dq5*dqr4*sin(2*q5)*sin(q4)*sin(q6))/2000 - (37*3^(1/2)*dq6*dqr4*sin(2*q5)*sin(q4)*sin(q6))/8000 - dq4*dqr4*cos(q4)*cos(q6)*sin(q5)*((37*3^(1/2))/4000 - 877/8000) - dq5*dqr4*cos(q5)*cos(q6)*sin(q4)*((37*3^(1/2))/4000 - 877/8000) - dq5*dqr4*cos(q4)*cos(q6)*sin(q5)*((37*3^(1/2))/8000 - 877/16000) + dq6*dqr4*cos(q4)*cos(q5)*sin(q6)*((111*3^(1/2))/8000 + 877/16000) - dq1*dqr4*cos(q2)*cos(q6)*sin(q3)*((1923*3^(1/2))/80000 + 259/16000) + dq1*dqr4*cos(q3)*cos(q6)*sin(q2)*((1923*3^(1/2))/80000 + 259/16000) - (111*dq1*dqr4*cos(2*q5)*cos(q2)*cos(q6)*sin(q3))/16000 + dq4*dqr4*sin(q4)*sin(q5)*sin(q6)*((37*3^(1/2))/2000 - 1231/20000) + dq1*dqr4*cos(2*q4)*cos(q2)*cos(q6)*sin(q3)*((1923*3^(1/2))/80000 + 111/3200) + (37*3^(1/2)*dq1*dqr5*cos(q6)*sin(q2)*sin(q3)*sin(q4))/4000 - (37*dq1*dqr4*cos(2*q4)*cos(2*q5)*cos(q2)*cos(q6)*sin(q3))/3200 - (37*dq1*dqr5*cos(2*q4)*cos(2*q5)*cos(q2)*cos(q6)*sin(q3))/4000 + (37*dq1*dqr5*cos(2*q4)*cos(2*q5)*cos(q3)*cos(q6)*sin(q2))/4000 + (37*dq1*dqr4*cos(2*q4)*sin(2*q5)*cos(q2)*sin(q3)*sin(q6))/1600 + (37*dq1*dqr4*cos(2*q5)*sin(2*q4)*cos(q2)*sin(q3)*sin(q6))/2000 + (37*dq1*dqr4*sin(2*q4)*sin(2*q5)*cos(q2)*cos(q6)*sin(q3))/4000 + (37*dq1*dqr5*cos(2*q4)*sin(2*q5)*cos(q2)*sin(q3)*sin(q6))/2000 - (37*dq1*dqr5*cos(2*q4)*sin(2*q5)*cos(q3)*sin(q2)*sin(q6))/2000 + (37*dq1*dqr5*cos(2*q5)*sin(2*q4)*cos(q2)*sin(q3)*sin(q6))/1600 - (37*dq1*dqr5*cos(2*q5)*sin(2*q4)*cos(q3)*sin(q2)*sin(q6))/1600 + (37*dq1*dqr5*sin(2*q4)*sin(2*q5)*cos(q2)*cos(q6)*sin(q3))/3200 - (37*dq1*dqr5*sin(2*q4)*sin(2*q5)*cos(q3)*cos(q6)*sin(q2))/3200 + (877*dq1*dqr4*cos(q2)*cos(q3)*cos(q4)*cos(q5)*sin(q6))/4000 + (1231*dq1*dqr4*cos(q2)*cos(q3)*cos(q5)*cos(q6)*sin(q4))/40000 + (877*dq1*dqr5*cos(q4)*cos(q5)*sin(q2)*sin(q3)*sin(q6))/8000 - (877*dq1*dqr5*sin(q2)*sin(q3)*sin(q4)*sin(q5)*sin(q6))/4000 + dq1*dqr4*cos(q2)*cos(q3)*cos(q6)*sin(q4)*((111*3^(1/2))/8000 + 7539/40000) - dq1*dqr4*cos(q2)*cos(q5)*cos(q6)*sin(q3)*((641*3^(1/2))/80000 - 37/8000) - dq1*dqr5*cos(q2)*cos(q5)*cos(q6)*sin(q3)*((641*3^(1/2))/80000 - 37/8000) + dq1*dqr5*cos(q3)*cos(q5)*cos(q6)*sin(q2)*((641*3^(1/2))/80000 - 37/8000) + dq1*dqr4*cos(q2)*sin(q3)*sin(q5)*sin(q6)*((641*3^(1/2))/40000 + 37/2000) + dq1*dqr5*cos(q2)*sin(q3)*sin(q5)*sin(q6)*((641*3^(1/2))/40000 + 37/2000) - dq1*dqr5*cos(q3)*sin(q2)*sin(q5)*sin(q6)*((641*3^(1/2))/40000 + 37/2000) + (37*3^(1/2)*dq1*dqr4*cos(2*q5)*cos(q2)*cos(q3)*cos(q4)*sin(q6))/2000 + (37*3^(1/2)*dq1*dqr4*cos(2*q5)*cos(q2)*cos(q3)*cos(q6)*sin(q4))/8000 + (37*3^(1/2)*dq1*dqr4*sin(2*q5)*cos(q2)*cos(q3)*cos(q4)*cos(q6))/4000 - (37*3^(1/2)*dq1*dqr4*sin(2*q5)*cos(q2)*cos(q3)*sin(q4)*sin(q6))/4000 + (37*3^(1/2)*dq1*dqr5*cos(2*q5)*cos(q4)*sin(q2)*sin(q3)*sin(q6))/4000 + (37*3^(1/2)*dq1*dqr5*cos(2*q5)*cos(q6)*sin(q2)*sin(q3)*sin(q4))/4000 + (37*3^(1/2)*dq1*dqr5*sin(2*q5)*cos(q4)*cos(q6)*sin(q2)*sin(q3))/8000 - (37*3^(1/2)*dq1*dqr5*sin(2*q5)*sin(q2)*sin(q3)*sin(q4)*sin(q6))/2000 - dq1*dqr4*cos(q2)*cos(q3)*cos(q4)*cos(q6)*sin(q5)*((37*3^(1/2))/4000 - 877/8000) - dq1*dqr5*cos(q5)*cos(q6)*sin(q2)*sin(q3)*sin(q4)*((37*3^(1/2))/4000 - 877/8000) + dq1*dqr4*cos(q2)*cos(q3)*sin(q4)*sin(q5)*sin(q6)*((37*3^(1/2))/2000 - 1231/20000) - dq1*dqr5*cos(q4)*cos(q6)*sin(q2)*sin(q3)*sin(q5)*((37*3^(1/2))/8000 - 877/16000) + dq1*dqr4*cos(2*q4)*cos(q2)*cos(q5)*cos(q6)*sin(q3)*((641*3^(1/2))/80000 - 37/8000) + dq1*dqr5*cos(2*q4)*cos(q2)*cos(q5)*cos(q6)*sin(q3)*((641*3^(1/2))/80000 - 37/8000) - dq1*dqr5*cos(2*q4)*cos(q3)*cos(q5)*cos(q6)*sin(q2)*((641*3^(1/2))/80000 - 37/8000) - dq1*dqr4*sin(2*q4)*cos(q2)*cos(q5)*sin(q3)*sin(q6)*((641*3^(1/2))/20000 + 37/1000) - dq1*dqr4*cos(2*q4)*cos(q2)*sin(q3)*sin(q5)*sin(q6)*((641*3^(1/2))/40000 + 37/2000) - dq1*dqr5*cos(2*q4)*cos(q2)*sin(q3)*sin(q5)*sin(q6)*((641*3^(1/2))/40000 + 37/2000) + dq1*dqr5*cos(2*q4)*cos(q3)*sin(q2)*sin(q5)*sin(q6)*((641*3^(1/2))/40000 + 37/2000) - dq1*dqr4*sin(2*q4)*cos(q2)*cos(q6)*sin(q3)*sin(q5)*((641*3^(1/2))/40000 - 37/4000) - dq1*dqr5*sin(2*q4)*cos(q2)*cos(q5)*sin(q3)*sin(q6)*((641*3^(1/2))/80000 + 37/4000) + dq1*dqr5*sin(2*q4)*cos(q3)*cos(q5)*sin(q2)*sin(q6)*((641*3^(1/2))/80000 + 37/4000) - dq1*dqr5*sin(2*q4)*cos(q2)*cos(q6)*sin(q3)*sin(q5)*((641*3^(1/2))/160000 - 37/16000) + dq1*dqr5*sin(2*q4)*cos(q3)*cos(q6)*sin(q2)*sin(q5)*((641*3^(1/2))/160000 - 37/16000);
Y3_10_5=(111*dq2*dqr5*cos(2*q5)*sin(q6))/8000 + (111*dq2*dqr5*sin(2*q5)*cos(q6))/16000 - (111*dq3*dqr5*cos(2*q5)*sin(q6))/8000 - (111*dq3*dqr5*sin(2*q5)*cos(q6))/16000 + (37*3^(1/2)*dq4*dqr5*cos(q6)*sin(q4))/4000 + (37*3^(1/2)*dq4*dqr6*cos(q6)*sin(q4))/4000 + (37*3^(1/2)*dq6*dqr5*cos(q4)*sin(q6))/4000 - (37*dq2*dqr5*cos(2*q4)*cos(2*q5)*sin(q6))/1600 - (37*dq2*dqr5*cos(2*q4)*sin(2*q5)*cos(q6))/3200 - (37*dq2*dqr5*cos(2*q5)*sin(2*q4)*cos(q6))/4000 + (37*dq3*dqr5*cos(2*q4)*cos(2*q5)*sin(q6))/1600 + (37*dq3*dqr5*cos(2*q4)*sin(2*q5)*cos(q6))/3200 + (37*dq3*dqr5*cos(2*q5)*sin(2*q4)*cos(q6))/4000 + (37*dq2*dqr5*sin(2*q4)*sin(2*q5)*sin(q6))/2000 - (37*dq3*dqr5*sin(2*q4)*sin(2*q5)*sin(q6))/2000 + (37*dq1*dqr5*cos(q2)*cos(q6)*sin(q3))/4000 + (37*dq1*dqr6*cos(q2)*cos(q6)*sin(q3))/4000 - (37*dq1*dqr6*cos(q3)*cos(q6)*sin(q2))/4000 + (877*dq4*dqr5*cos(q4)*cos(q5)*sin(q6))/8000 + (877*dq4*dqr6*cos(q5)*cos(q6)*sin(q4))/4000 + (877*dq5*dqr5*cos(q4)*cos(q5)*sin(q6))/4000 + (877*dq6*dqr5*cos(q4)*cos(q5)*sin(q6))/8000 + (877*dq6*dqr5*cos(q4)*cos(q6)*sin(q5))/4000 - (877*dq4*dqr5*sin(q4)*sin(q5)*sin(q6))/4000 - (877*dq4*dqr6*sin(q4)*sin(q5)*sin(q6))/8000 + dq2*dqr5*cos(q5)*sin(q6)*((8129*3^(1/2))/80000 - 37/4000) - dq3*dqr5*cos(q5)*sin(q6)*((8129*3^(1/2))/80000 - 37/4000) + dq2*dqr5*cos(q6)*sin(q5)*((8129*3^(1/2))/160000 - 37/3200) - dq3*dqr5*cos(q6)*sin(q5)*((8129*3^(1/2))/160000 - 37/3200) + dq2*dqr5*cos(2*q4)*cos(q5)*sin(q6)*((641*3^(1/2))/80000 + 37/4000) - dq3*dqr5*cos(2*q4)*cos(q5)*sin(q6)*((641*3^(1/2))/80000 + 37/4000) + dq2*dqr5*sin(2*q4)*cos(q5)*cos(q6)*((641*3^(1/2))/80000 - 37/8000) - dq3*dqr5*sin(2*q4)*cos(q5)*cos(q6)*((641*3^(1/2))/80000 - 37/8000) + dq2*dqr5*cos(2*q4)*cos(q6)*sin(q5)*((641*3^(1/2))/160000 - 37/16000) - dq3*dqr5*cos(2*q4)*cos(q6)*sin(q5)*((641*3^(1/2))/160000 - 37/16000) - dq2*dqr5*sin(2*q4)*sin(q5)*sin(q6)*((641*3^(1/2))/40000 + 37/2000) + dq3*dqr5*sin(2*q4)*sin(q5)*sin(q6)*((641*3^(1/2))/40000 + 37/2000) + (37*3^(1/2)*dq4*dqr5*cos(2*q5)*cos(q4)*sin(q6))/4000 + (37*3^(1/2)*dq4*dqr5*cos(2*q5)*cos(q6)*sin(q4))/4000 + (37*3^(1/2)*dq4*dqr5*sin(2*q5)*cos(q4)*cos(q6))/8000 + (37*3^(1/2)*dq4*dqr6*cos(2*q5)*cos(q6)*sin(q4))/4000 - (37*3^(1/2)*dq4*dqr5*sin(2*q5)*sin(q4)*sin(q6))/2000 - (37*3^(1/2)*dq4*dqr6*sin(2*q5)*sin(q4)*sin(q6))/8000 - dq4*dqr5*cos(q5)*cos(q6)*sin(q4)*((37*3^(1/2))/4000 - 877/8000) - dq5*dqr5*cos(q4)*cos(q6)*sin(q5)*((37*3^(1/2))/4000 - 877/8000) + dq5*dqr6*cos(q5)*cos(q6)*sin(q4)*((37*3^(1/2))/2000 + 1577/10000) + dq6*dqr5*cos(q5)*cos(q6)*sin(q4)*((37*3^(1/2))/2000 + 1577/10000) - dq4*dqr5*cos(q4)*cos(q6)*sin(q5)*((37*3^(1/2))/8000 - 877/16000) - dq5*dqr5*cos(q5)*cos(q6)*sin(q4)*((37*3^(1/2))/4000 - 1577/20000) + dq6*dqr6*cos(q5)*cos(q6)*sin(q4)*((111*3^(1/2))/4000 + 1577/20000) - dq5*dqr5*sin(q4)*sin(q5)*sin(q6)*((37*3^(1/2))/2000 + 1577/10000) - dq6*dqr6*sin(q4)*sin(q5)*sin(q6)*((37*3^(1/2))/2000 + 1577/10000) - dq5*dqr6*sin(q4)*sin(q5)*sin(q6)*((37*3^(1/2))/4000 + 1577/20000) - dq6*dqr5*sin(q4)*sin(q5)*sin(q6)*((37*3^(1/2))/4000 + 1577/20000) + (37*3^(1/2)*dq1*dqr6*cos(q6)*sin(q2)*sin(q3)*sin(q4))/4000 - (37*dq1*dqr6*cos(2*q4)*cos(2*q5)*cos(q2)*cos(q6)*sin(q3))/4000 + (37*dq1*dqr6*cos(2*q4)*cos(2*q5)*cos(q3)*cos(q6)*sin(q2))/4000 - dq1*dqr6*sin(2*q4)*cos(q2)*sin(q3)*sin(q6)*((1923*3^(1/2))/160000 + 111/6400) + dq1*dqr6*sin(2*q4)*cos(q3)*sin(q2)*sin(q6)*((1923*3^(1/2))/160000 + 111/6400) + (37*dq1*dqr6*cos(2*q4)*sin(2*q5)*cos(q2)*sin(q3)*sin(q6))/8000 - (37*dq1*dqr6*cos(2*q4)*sin(2*q5)*cos(q3)*sin(q2)*sin(q6))/8000 + (37*dq1*dqr6*cos(2*q5)*sin(2*q4)*cos(q2)*sin(q3)*sin(q6))/6400 - (37*dq1*dqr6*cos(2*q5)*sin(2*q4)*cos(q3)*sin(q2)*sin(q6))/6400 + (37*dq1*dqr6*sin(2*q4)*sin(2*q5)*cos(q2)*cos(q6)*sin(q3))/3200 - (37*dq1*dqr6*sin(2*q4)*sin(2*q5)*cos(q3)*cos(q6)*sin(q2))/3200 + (877*dq1*dqr5*cos(q2)*cos(q3)*cos(q4)*cos(q5)*sin(q6))/8000 + (877*dq1*dqr6*cos(q2)*cos(q3)*cos(q5)*cos(q6)*sin(q4))/4000 - (877*dq1*dqr5*cos(q2)*cos(q3)*sin(q4)*sin(q5)*sin(q6))/4000 - (877*dq1*dqr6*cos(q2)*cos(q3)*sin(q4)*sin(q5)*sin(q6))/8000 + (877*dq1*dqr6*cos(q4)*cos(q6)*sin(q2)*sin(q3)*sin(q5))/8000 + (877*dq1*dqr6*cos(q5)*cos(q6)*sin(q2)*sin(q3)*sin(q4))/4000 - (877*dq1*dqr6*sin(q2)*sin(q3)*sin(q4)*sin(q5)*sin(q6))/8000 - dq1*dqr6*cos(q2)*cos(q5)*cos(q6)*sin(q3)*((641*3^(1/2))/40000 + 37/2000) + dq1*dqr6*cos(q3)*cos(q5)*cos(q6)*sin(q2)*((641*3^(1/2))/40000 + 37/2000) + dq1*dqr6*cos(q4)*sin(q2)*sin(q3)*sin(q6)*((37*3^(1/2))/16000 + 2631/16000) + dq1*dqr6*cos(q2)*sin(q3)*sin(q5)*sin(q6)*((641*3^(1/2))/80000 + 37/1600) - dq1*dqr6*cos(q3)*sin(q2)*sin(q5)*sin(q6)*((641*3^(1/2))/80000 + 37/1600) + (37*3^(1/2)*dq1*dqr5*cos(q2)*cos(q3)*cos(q6)*sin(q4))/4000 + (37*3^(1/2)*dq1*dqr6*cos(q2)*cos(q3)*cos(q6)*sin(q4))/4000 + (37*3^(1/2)*dq1*dqr5*cos(2*q5)*cos(q2)*cos(q3)*cos(q4)*sin(q6))/4000 + (37*3^(1/2)*dq1*dqr5*cos(2*q5)*cos(q2)*cos(q3)*cos(q6)*sin(q4))/4000 + (37*3^(1/2)*dq1*dqr5*sin(2*q5)*cos(q2)*cos(q3)*cos(q4)*cos(q6))/8000 + (37*3^(1/2)*dq1*dqr6*cos(2*q5)*cos(q2)*cos(q3)*cos(q6)*sin(q4))/4000 - (37*3^(1/2)*dq1*dqr5*sin(2*q5)*cos(q2)*cos(q3)*sin(q4)*sin(q6))/2000 + (37*3^(1/2)*dq1*dqr6*cos(2*q5)*cos(q4)*sin(q2)*sin(q3)*sin(q6))/16000 + (37*3^(1/2)*dq1*dqr6*cos(2*q5)*cos(q6)*sin(q2)*sin(q3)*sin(q4))/4000 - (37*3^(1/2)*dq1*dqr6*sin(2*q5)*cos(q2)*cos(q3)*sin(q4)*sin(q6))/8000 + (37*3^(1/2)*dq1*dqr6*sin(2*q5)*cos(q4)*cos(q6)*sin(q2)*sin(q3))/8000 - (37*3^(1/2)*dq1*dqr6*sin(2*q5)*sin(q2)*sin(q3)*sin(q4)*sin(q6))/8000 - dq1*dqr5*cos(q2)*cos(q3)*cos(q5)*cos(q6)*sin(q4)*((37*3^(1/2))/4000 - 877/8000) - dq1*dqr5*cos(q2)*cos(q3)*cos(q4)*cos(q6)*sin(q5)*((37*3^(1/2))/8000 - 877/16000) + dq1*dqr6*cos(q4)*cos(q5)*sin(q2)*sin(q3)*sin(q6)*((111*3^(1/2))/8000 + 877/16000) + dq1*dqr6*cos(2*q4)*cos(q2)*cos(q5)*cos(q6)*sin(q3)*((641*3^(1/2))/40000 + 37/2000) - dq1*dqr6*cos(2*q4)*cos(q3)*cos(q5)*cos(q6)*sin(q2)*((641*3^(1/2))/40000 + 37/2000) - dq1*dqr6*sin(2*q4)*cos(q2)*cos(q6)*sin(q3)*sin(q5)*((641*3^(1/2))/80000 + 37/4000) + dq1*dqr6*sin(2*q4)*cos(q3)*cos(q6)*sin(q2)*sin(q5)*((641*3^(1/2))/80000 + 37/4000) - dq1*dqr6*cos(2*q4)*cos(q2)*sin(q3)*sin(q5)*sin(q6)*((641*3^(1/2))/80000 - 37/8000) + dq1*dqr6*cos(2*q4)*cos(q3)*sin(q2)*sin(q5)*sin(q6)*((641*3^(1/2))/80000 - 37/8000) - dq1*dqr6*sin(2*q4)*cos(q2)*cos(q5)*sin(q3)*sin(q6)*((641*3^(1/2))/160000 - 37/16000) + dq1*dqr6*sin(2*q4)*cos(q3)*cos(q5)*sin(q2)*sin(q6)*((641*3^(1/2))/160000 - 37/16000);
Y3_10_6=dq3*dqr6*sin(q6)*((10693*3^(1/2))/160000 + 37/32000) - dq2*dqr6*sin(q6)*((10693*3^(1/2))/160000 + 37/32000) + (111*dq2*dqr6*cos(2*q5)*sin(q6))/32000 + (111*dq2*dqr6*sin(2*q5)*cos(q6))/16000 - (111*dq3*dqr6*cos(2*q5)*sin(q6))/32000 - (111*dq3*dqr6*sin(2*q5)*cos(q6))/16000 + (37*ddqr1*cos(q3)*sin(q2)*sin(q6))/2000 + (87*ddqr2*cos(q6)*sin(q3)*sin(q4))/400 - (21*ddqr1*cos(q2)*cos(q6)*sin(q3)*sin(q4))/4000 + (21*ddqr1*cos(q3)*cos(q6)*sin(q2)*sin(q4))/4000 + (29*ddqr2*cos(q4)*cos(q6)*sin(q3)*sin(q5))/200 + (29*ddqr2*cos(q5)*cos(q6)*sin(q3)*sin(q4))/400 + (37*3^(1/2)*dq5*dqr6*cos(q4)*sin(q6))/4000 + (37*3^(1/2)*dq6*dqr6*cos(q4)*sin(q6))/2000 - (29*ddqr2*sin(q3)*sin(q4)*sin(q5)*sin(q6))/200 + dq2*dqr6*cos(2*q4)*sin(q6)*((1923*3^(1/2))/160000 + 111/6400) - dq3*dqr6*cos(2*q4)*sin(q6)*((1923*3^(1/2))/160000 + 111/6400) - (37*dq2*dqr6*cos(2*q4)*cos(2*q5)*sin(q6))/6400 - (37*dq2*dqr6*cos(2*q4)*sin(2*q5)*cos(q6))/3200 - (37*dq2*dqr6*cos(2*q5)*sin(2*q4)*cos(q6))/4000 + (37*dq3*dqr6*cos(2*q4)*cos(2*q5)*sin(q6))/6400 + (37*dq3*dqr6*cos(2*q4)*sin(2*q5)*cos(q6))/3200 + (37*dq3*dqr6*cos(2*q5)*sin(2*q4)*cos(q6))/4000 + (37*dq2*dqr6*sin(2*q4)*sin(2*q5)*sin(q6))/8000 - (37*dq3*dqr6*sin(2*q4)*sin(2*q5)*sin(q6))/8000 + (37*ddqr1*cos(q2)*cos(q4)^2*sin(q3)*sin(q6))/1000 - (37*ddqr1*cos(q3)*cos(q4)^2*sin(q2)*sin(q6))/1000 + (37*ddqr1*cos(q2)*cos(q5)^2*sin(q3)*sin(q6))/1000 - (37*ddqr1*cos(q3)*cos(q5)^2*sin(q2)*sin(q6))/1000 + (877*dq4*dqr6*cos(q4)*cos(q6)*sin(q5))/8000 + (877*dq5*dqr6*cos(q4)*cos(q5)*sin(q6))/8000 + (877*dq5*dqr6*cos(q4)*cos(q6)*sin(q5))/4000 + (877*dq6*dqr6*cos(q4)*cos(q5)*sin(q6))/4000 + (7*3^(1/2)*ddqr1*cos(q6)*sin(q2)*sin(q3))/4000 - dq6*dqr6*cos(q6)*sin(q4)*((37*3^(1/2))/4000 - 351/2500) + dq4*dqr6*cos(q4)*sin(q6)*((37*3^(1/2))/16000 + 2631/16000) + dq2*dqr6*cos(q6)*sin(q5)*((8129*3^(1/2))/80000 - 37/4000) - dq3*dqr6*cos(q6)*sin(q5)*((8129*3^(1/2))/80000 - 37/4000) + dq2*dqr6*cos(q5)*sin(q6)*((8129*3^(1/2))/160000 - 37/3200) - dq3*dqr6*cos(q5)*sin(q6)*((8129*3^(1/2))/160000 - 37/3200) - (7*ddqr1*cos(q2)*cos(q4)*cos(q5)*sin(q3)*sin(q6))/1000 - (7*ddqr1*cos(q2)*cos(q4)*cos(q6)*sin(q3)*sin(q5))/2000 - (7*ddqr1*cos(q2)*cos(q5)*cos(q6)*sin(q3)*sin(q4))/4000 + (7*ddqr1*cos(q3)*cos(q4)*cos(q5)*sin(q2)*sin(q6))/1000 + (7*ddqr1*cos(q3)*cos(q4)*cos(q6)*sin(q2)*sin(q5))/2000 + (7*ddqr1*cos(q3)*cos(q5)*cos(q6)*sin(q2)*sin(q4))/4000 - (1231*ddqr1*cos(q4)*cos(q5)*cos(q6)*sin(q2)*sin(q3))/40000 + (37*ddqr1*cos(q2)*cos(q5)*cos(q6)*sin(q3)*sin(q5))/2000 - (37*ddqr1*cos(q3)*cos(q5)*cos(q6)*sin(q2)*sin(q5))/2000 + (7*ddqr1*cos(q2)*sin(q3)*sin(q4)*sin(q5)*sin(q6))/2000 - (7*ddqr1*cos(q3)*sin(q2)*sin(q4)*sin(q5)*sin(q6))/2000 + (877*ddqr1*cos(q5)*sin(q2)*sin(q3)*sin(q4)*sin(q6))/4000 + dq2*dqr6*sin(2*q4)*cos(q5)*cos(q6)*((641*3^(1/2))/40000 + 37/2000) - dq3*dqr6*sin(2*q4)*cos(q5)*cos(q6)*((641*3^(1/2))/40000 + 37/2000) + dq2*dqr6*cos(2*q4)*cos(q6)*sin(q5)*((641*3^(1/2))/80000 + 37/4000) - dq3*dqr6*cos(2*q4)*cos(q6)*sin(q5)*((641*3^(1/2))/80000 + 37/4000) + dq2*dqr6*cos(2*q4)*cos(q5)*sin(q6)*((641*3^(1/2))/160000 - 37/16000) - dq3*dqr6*cos(2*q4)*cos(q5)*sin(q6)*((641*3^(1/2))/160000 - 37/16000) - dq2*dqr6*sin(2*q4)*sin(q5)*sin(q6)*((641*3^(1/2))/80000 - 37/8000) + dq3*dqr6*sin(2*q4)*sin(q5)*sin(q6)*((641*3^(1/2))/80000 - 37/8000) + ddqr1*cos(q3)*cos(q5)*sin(q2)*sin(q6)*((641*3^(1/2))/20000 + 37/1000) - ddqr1*cos(q2)*cos(q6)*sin(q3)*sin(q5)*((641*3^(1/2))/40000 - 37/4000) + ddqr1*cos(q3)*cos(q6)*sin(q2)*sin(q5)*((641*3^(1/2))/40000 - 37/4000) - ddqr1*cos(q4)*cos(q6)*sin(q2)*sin(q3)*((37*3^(1/2))/4000 + 7539/40000) + (37*3^(1/2)*dq4*dqr6*cos(2*q5)*cos(q4)*sin(q6))/16000 + (37*3^(1/2)*dq4*dqr6*sin(2*q5)*cos(q4)*cos(q6))/8000 - (7*3^(1/2)*ddqr1*cos(q5)*cos(q6)*sin(q2)*sin(q3))/4000 - (37*3^(1/2)*ddqr1*sin(q2)*sin(q3)*sin(q4)*sin(q6))/2000 + (7*3^(1/2)*ddqr1*sin(q2)*sin(q3)*sin(q5)*sin(q6))/2000 - (37*ddqr1*cos(q2)*cos(q4)^2*cos(q5)^2*sin(q3)*sin(q6))/500 + (37*ddqr1*cos(q3)*cos(q4)^2*cos(q5)^2*sin(q2)*sin(q6))/500 + dq6*dqr6*cos(q4)*cos(q6)*sin(q5)*((37*3^(1/2))/4000 + 877/8000) + dq4*dqr6*cos(q4)*cos(q5)*sin(q6)*((111*3^(1/2))/8000 + 877/16000) + ddqr1*cos(q2)*cos(q4)*cos(q6)*sin(q3)*sin(q4)*((1923*3^(1/2))/40000 + 37/400) - ddqr1*cos(q3)*cos(q4)*cos(q6)*sin(q2)*sin(q4)*((1923*3^(1/2))/40000 + 37/400) - (37*ddqr1*cos(q2)*cos(q4)*cos(q5)^2*cos(q6)*sin(q3)*sin(q4))/800 + (37*ddqr1*cos(q3)*cos(q4)*cos(q5)^2*cos(q6)*sin(q2)*sin(q4))/800 - (37*ddqr1*cos(q2)*cos(q4)^2*cos(q5)*cos(q6)*sin(q3)*sin(q5))/1000 + (37*ddqr1*cos(q3)*cos(q4)^2*cos(q5)*cos(q6)*sin(q2)*sin(q5))/1000 - ddqr1*cos(q6)*sin(q2)*sin(q3)*sin(q4)*sin(q5)*((37*3^(1/2))/4000 - 877/8000) - ddqr1*cos(q4)*sin(q2)*sin(q3)*sin(q5)*sin(q6)*((37*3^(1/2))/2000 - 1231/20000) + (877*dq1*dqr6*cos(q2)*cos(q3)*cos(q4)*cos(q6)*sin(q5))/8000 + ddqr1*cos(q2)*cos(q4)^2*cos(q5)*sin(q3)*sin(q6)*((641*3^(1/2))/10000 + 37/500) - ddqr1*cos(q3)*cos(q4)^2*cos(q5)*sin(q2)*sin(q6)*((641*3^(1/2))/10000 + 37/500) + ddqr1*cos(q2)*cos(q4)^2*cos(q6)*sin(q3)*sin(q5)*((641*3^(1/2))/20000 - 37/2000) - ddqr1*cos(q3)*cos(q4)^2*cos(q6)*sin(q2)*sin(q5)*((641*3^(1/2))/20000 - 37/2000) + dq1*dqr6*cos(q2)*cos(q3)*cos(q4)*sin(q6)*((37*3^(1/2))/16000 + 2631/16000) - (37*3^(1/2)*ddqr1*cos(q4)*cos(q5)^2*cos(q6)*sin(q2)*sin(q3))/4000 + (37*3^(1/2)*ddqr1*cos(q5)^2*sin(q2)*sin(q3)*sin(q4)*sin(q6))/1000 - ddqr1*cos(q2)*cos(q4)*sin(q3)*sin(q4)*sin(q5)*sin(q6)*((641*3^(1/2))/20000 + 37/1000) + ddqr1*cos(q3)*cos(q4)*sin(q2)*sin(q4)*sin(q5)*sin(q6)*((641*3^(1/2))/20000 + 37/1000) + (37*3^(1/2)*dq1*dqr6*cos(2*q5)*cos(q2)*cos(q3)*cos(q4)*sin(q6))/16000 + (37*3^(1/2)*dq1*dqr6*sin(2*q5)*cos(q2)*cos(q3)*cos(q4)*cos(q6))/8000 + (37*3^(1/2)*ddqr1*cos(q4)*cos(q5)*sin(q2)*sin(q3)*sin(q5)*sin(q6))/2000 + (37*3^(1/2)*ddqr1*cos(q5)*cos(q6)*sin(q2)*sin(q3)*sin(q4)*sin(q5))/2000 + dq1*dqr6*cos(q2)*cos(q3)*cos(q4)*cos(q5)*sin(q6)*((111*3^(1/2))/8000 + 877/16000) + (37*ddqr1*cos(q2)*cos(q4)*cos(q5)*sin(q3)*sin(q4)*sin(q5)*sin(q6))/400 - (37*ddqr1*cos(q3)*cos(q4)*cos(q5)*sin(q2)*sin(q4)*sin(q5)*sin(q6))/400 + ddqr1*cos(q2)*cos(q4)*cos(q5)*cos(q6)*sin(q3)*sin(q4)*((641*3^(1/2))/40000 - 37/4000) - ddqr1*cos(q3)*cos(q4)*cos(q5)*cos(q6)*sin(q2)*sin(q4)*((641*3^(1/2))/40000 - 37/4000);
Y3_10_7=ddqr2*cos(q6)*((1577*3^(1/2))/10000 + 111/2000) - ddqr3*cos(q6)*((1577*3^(1/2))/10000 + 111/2000) - (37*ddqr2*cos(q5)^2*cos(q6))/1000 + (37*ddqr3*cos(q5)^2*cos(q6))/1000 + (37*ddqr2*cos(q4)^2*cos(q5)^2*cos(q6))/800 - (37*ddqr3*cos(q4)^2*cos(q5)^2*cos(q6))/800 - (1231*ddqr4*cos(q4)*cos(q5)*cos(q6))/40000 - (877*ddqr6*cos(q4)*cos(q5)*cos(q6))/4000 - (37*ddqr1*cos(q2)*sin(q3)*sin(q6))/2000 + (37*ddqr2*cos(q4)*sin(q4)*sin(q6))/1000 - (37*ddqr3*cos(q4)*sin(q4)*sin(q6))/1000 + (37*ddqr2*cos(q5)*sin(q5)*sin(q6))/500 - (37*ddqr3*cos(q5)*sin(q5)*sin(q6))/500 + (877*ddqr4*cos(q5)*sin(q4)*sin(q6))/4000 + (877*ddqr5*cos(q4)*sin(q5)*sin(q6))/4000 - ddqr2*cos(q5)*cos(q6)*((117*3^(1/2))/1250 - 37/2000) + ddqr3*cos(q5)*cos(q6)*((117*3^(1/2))/1250 - 37/2000) - ddqr4*cos(q4)*cos(q6)*((37*3^(1/2))/4000 + 7539/40000) + ddqr2*sin(q5)*sin(q6)*((117*3^(1/2))/625 - 37/1000) - ddqr3*sin(q5)*sin(q6)*((117*3^(1/2))/625 - 37/1000) - ddqr6*sin(q4)*sin(q6)*((37*3^(1/2))/4000 - 351/2500) - (29*3^(1/2)*ddqr2*cos(q3)*cos(q6))/400 - (37*3^(1/2)*ddqr5*cos(q4)*cos(q6))/2000 - (37*3^(1/2)*ddqr6*cos(q4)*cos(q6))/2000 - ddqr2*cos(q4)^2*cos(q6)*((1923*3^(1/2))/40000 + 37/400) + ddqr3*cos(q4)^2*cos(q6)*((1923*3^(1/2))/40000 + 37/400) - (37*3^(1/2)*ddqr4*sin(q4)*sin(q6))/2000 - (37*3^(1/2)*ddqr4*cos(q4)*cos(q5)^2*cos(q6))/4000 + (37*3^(1/2)*ddqr4*cos(q5)^2*sin(q4)*sin(q6))/1000 + (29*ddqr2*cos(q4)*cos(q5)*sin(q3)*sin(q6))/100 + ddqr5*cos(q4)*cos(q5)*cos(q6)*((37*3^(1/2))/4000 - 877/8000) - ddqr4*cos(q6)*sin(q4)*sin(q5)*((37*3^(1/2))/4000 - 877/8000) + ddqr6*cos(q4)*sin(q5)*sin(q6)*((37*3^(1/2))/4000 + 877/8000) + ddqr5*cos(q5)*sin(q4)*sin(q6)*((37*3^(1/2))/2000 + 1577/10000) + ddqr6*cos(q6)*sin(q4)*sin(q5)*((37*3^(1/2))/2000 + 1577/10000) - ddqr4*cos(q4)*sin(q5)*sin(q6)*((37*3^(1/2))/2000 - 1231/20000) - ddqr5*cos(q6)*sin(q4)*sin(q5)*((37*3^(1/2))/4000 - 1577/20000) + ddqr6*cos(q5)*sin(q4)*sin(q6)*((111*3^(1/2))/4000 + 1577/20000) - (37*ddqr2*cos(q4)*cos(q5)^2*sin(q4)*sin(q6))/500 - (37*ddqr2*cos(q4)^2*cos(q5)*sin(q5)*sin(q6))/400 + (37*ddqr3*cos(q4)*cos(q5)^2*sin(q4)*sin(q6))/500 + (37*ddqr3*cos(q4)^2*cos(q5)*sin(q5)*sin(q6))/400 + (7*3^(1/2)*ddqr1*cos(q2)*cos(q3)*cos(q6))/4000 + (29*3^(1/2)*ddqr2*cos(q3)*cos(q5)*cos(q6))/400 - ddqr2*cos(q4)^2*cos(q5)*cos(q6)*((641*3^(1/2))/40000 - 37/4000) + ddqr3*cos(q4)^2*cos(q5)*cos(q6)*((641*3^(1/2))/40000 - 37/4000) - (29*3^(1/2)*ddqr2*cos(q3)*sin(q5)*sin(q6))/200 + ddqr2*cos(q4)^2*sin(q5)*sin(q6)*((641*3^(1/2))/20000 + 37/1000) - ddqr3*cos(q4)^2*sin(q5)*sin(q6)*((641*3^(1/2))/20000 + 37/1000) + (877*ddqr1*cos(q2)*cos(q3)*cos(q5)*sin(q4)*sin(q6))/4000 - (37*ddqr2*cos(q4)*cos(q5)*cos(q6)*sin(q4)*sin(q5))/1000 + (37*ddqr3*cos(q4)*cos(q5)*cos(q6)*sin(q4)*sin(q5))/1000 - ddqr1*cos(q2)*cos(q3)*cos(q4)*cos(q6)*((37*3^(1/2))/4000 + 7539/40000) + ddqr2*cos(q4)*cos(q5)*sin(q4)*sin(q6)*((641*3^(1/2))/10000 + 37/500) - ddqr3*cos(q4)*cos(q5)*sin(q4)*sin(q6)*((641*3^(1/2))/10000 + 37/500) - ddqr1*cos(q2)*cos(q5)*sin(q3)*sin(q6)*((641*3^(1/2))/20000 + 37/1000) + ddqr2*cos(q4)*cos(q6)*sin(q4)*sin(q5)*((641*3^(1/2))/20000 - 37/2000) - ddqr3*cos(q4)*cos(q6)*sin(q4)*sin(q5)*((641*3^(1/2))/20000 - 37/2000) - (7*3^(1/2)*ddqr1*cos(q2)*cos(q3)*cos(q5)*cos(q6))/4000 - (37*3^(1/2)*ddqr1*cos(q2)*cos(q3)*sin(q4)*sin(q6))/2000 + (7*3^(1/2)*ddqr1*cos(q2)*cos(q3)*sin(q5)*sin(q6))/2000 + (37*3^(1/2)*ddqr4*cos(q4)*cos(q5)*sin(q5)*sin(q6))/2000 + (37*3^(1/2)*ddqr4*cos(q5)*cos(q6)*sin(q4)*sin(q5))/2000 - (1231*ddqr1*cos(q2)*cos(q3)*cos(q4)*cos(q5)*cos(q6))/40000 - ddqr1*cos(q2)*cos(q3)*cos(q6)*sin(q4)*sin(q5)*((37*3^(1/2))/4000 - 877/8000) - ddqr1*cos(q2)*cos(q3)*cos(q4)*sin(q5)*sin(q6)*((37*3^(1/2))/2000 - 1231/20000) - (37*3^(1/2)*ddqr1*cos(q2)*cos(q3)*cos(q4)*cos(q5)^2*cos(q6))/4000 + (37*3^(1/2)*ddqr1*cos(q2)*cos(q3)*cos(q5)^2*sin(q4)*sin(q6))/1000 + (37*3^(1/2)*ddqr1*cos(q2)*cos(q3)*cos(q4)*cos(q5)*sin(q5)*sin(q6))/2000 + (37*3^(1/2)*ddqr1*cos(q2)*cos(q3)*cos(q5)*cos(q6)*sin(q4)*sin(q5))/2000;
Y3_12_1=(1231*cos(q3)*sin(q2))/10000 - (1231*cos(q2)*sin(q3))/10000;
Y3_13_1=(117*cos(q3)*sin(q2))/625 - (117*cos(q2)*sin(q3))/625 - (37*sin(q2)*sin(q3)*sin(q4))/1000 - (37*cos(q2)*cos(q3)*sin(q4))/1000;
Y3_14_1=(877*cos(q3)*sin(q2))/4000 - (877*cos(q2)*sin(q3))/4000 - cos(q2)*cos(q3)*sin(q4)*((641*3^(1/2))/20000 + 37/1000) - sin(q2)*sin(q3)*sin(q4)*((641*3^(1/2))/20000 + 37/1000) - (37*3^(1/2)*cos(q2)*cos(q5)*sin(q3))/2000 + (37*3^(1/2)*cos(q3)*cos(q5)*sin(q2))/2000 + (37*cos(q2)*cos(q3)*cos(q4)*sin(q5))/1000 + (37*cos(q2)*cos(q3)*cos(q5)*sin(q4))/2000 + (37*cos(q4)*sin(q2)*sin(q3)*sin(q5))/1000 + (37*cos(q5)*sin(q2)*sin(q3)*sin(q4))/2000;
Y3_17_1=ddqr3 - ddqr2 - (dq1*dqr1*cos(2*q2)*sin(2*q3))/2 + (dq1*dqr1*cos(2*q3)*sin(2*q2))/2;
Y3_18_1=ddqr3 - ddqr2 + ddqr2*cos(q4)^2 - ddqr3*cos(q4)^2 - (dq2*dqr4*sin(2*q4))/2 - (dq4*dqr2*sin(2*q4))/2 + (dq3*dqr4*sin(2*q4))/2 + (dq4*dqr3*sin(2*q4))/2 + (dq1*dqr1*cos(2*q2)*sin(2*q3))/4 - (dq1*dqr1*cos(2*q3)*sin(2*q2))/4 + (dq1*dqr4*cos(q2)*sin(q3))/2 - (dq1*dqr4*cos(q3)*sin(q2))/2 + (dq4*dqr1*cos(q2)*sin(q3))/2 - (dq4*dqr1*cos(q3)*sin(q2))/2 - (dq1*dqr4*cos(2*q4)*cos(q2)*sin(q3))/2 + (dq1*dqr4*cos(2*q4)*cos(q3)*sin(q2))/2 - (dq4*dqr1*cos(2*q4)*cos(q2)*sin(q3))/2 + (dq4*dqr1*cos(2*q4)*cos(q3)*sin(q2))/2 - ddqr1*cos(q2)*cos(q4)*sin(q3)*sin(q4) + ddqr1*cos(q3)*cos(q4)*sin(q2)*sin(q4) - (dq1*dqr1*cos(2*q2)*cos(2*q4)*sin(2*q3))/4 + (dq1*dqr1*cos(2*q3)*cos(2*q4)*sin(2*q2))/4;
Y3_19_1=(3*dq2*dqr4*sin(2*q4))/16 + (3*dq4*dqr2*sin(2*q4))/16 - (3*dq3*dqr4*sin(2*q4))/16 - (3*dq4*dqr3*sin(2*q4))/16 + (3*dq5*dqr2*sin(2*q5))/16 - (3*dq5*dqr3*sin(2*q5))/16 + (3^(1/2)*dq4*dqr4*sin(q4))/8 + (3^(1/2)*dq4*dqr5*sin(q4))/4 + (3^(1/2)*dq5*dqr4*sin(q4))/4 - (dq1*dqr1*cos(2*q2)*sin(2*q3))/32 + (dq1*dqr1*cos(2*q3)*sin(2*q2))/32 - (dq2*dqr4*cos(2*q4)*sin(2*q5))/4 - (5*dq2*dqr4*cos(2*q5)*sin(2*q4))/16 - (dq4*dqr2*cos(2*q4)*sin(2*q5))/4 - (5*dq4*dqr2*cos(2*q5)*sin(2*q4))/16 - (dq2*dqr5*cos(2*q5)*sin(2*q4))/4 + (dq3*dqr4*cos(2*q4)*sin(2*q5))/4 + (5*dq3*dqr4*cos(2*q5)*sin(2*q4))/16 + (dq4*dqr3*cos(2*q4)*sin(2*q5))/4 + (5*dq4*dqr3*cos(2*q5)*sin(2*q4))/16 - (5*dq5*dqr2*cos(2*q4)*sin(2*q5))/16 - (dq5*dqr2*cos(2*q5)*sin(2*q4))/4 + (5*dq5*dqr3*cos(2*q4)*sin(2*q5))/16 + (dq5*dqr3*cos(2*q5)*sin(2*q4))/4 + (5*dq1*dqr4*cos(q2)*sin(q3))/16 - (5*dq1*dqr4*cos(q3)*sin(q2))/16 + (5*dq4*dqr1*cos(q2)*sin(q3))/16 - (5*dq4*dqr1*cos(q3)*sin(q2))/16 + (dq1*dqr5*cos(q2)*sin(q3))/4 - (dq1*dqr5*cos(q3)*sin(q2))/4 + (dq5*dqr1*cos(q2)*sin(q3))/4 - (dq5*dqr1*cos(q3)*sin(q2))/4 + (3*dq1*dqr4*cos(2*q4)*cos(q2)*sin(q3))/16 - (3*dq1*dqr4*cos(2*q4)*cos(q3)*sin(q2))/16 + (3*dq4*dqr1*cos(2*q4)*cos(q2)*sin(q3))/16 - (3*dq4*dqr1*cos(2*q4)*cos(q3)*sin(q2))/16 - (3*dq1*dqr4*cos(2*q5)*cos(q2)*sin(q3))/16 + (3*dq1*dqr4*cos(2*q5)*cos(q3)*sin(q2))/16 - (3*dq4*dqr1*cos(2*q5)*cos(q2)*sin(q3))/16 + (3*dq4*dqr1*cos(2*q5)*cos(q3)*sin(q2))/16 + (3^(1/2)*dq4*dqr4*cos(2*q5)*sin(q4))/8 + (3^(1/2)*dq4*dqr4*sin(2*q5)*cos(q4))/4 + (3^(1/2)*dq4*dqr5*cos(2*q5)*sin(q4))/4 + (3^(1/2)*dq4*dqr5*sin(2*q5)*cos(q4))/8 + (3^(1/2)*dq5*dqr4*cos(2*q5)*sin(q4))/4 + (3^(1/2)*dq5*dqr4*sin(2*q5)*cos(q4))/8 + (3*dq1*dqr1*cos(2*q2)*cos(2*q4)*sin(2*q3))/32 - (3*dq1*dqr1*cos(2*q3)*cos(2*q4)*sin(2*q2))/32 - (9*dq1*dqr1*cos(2*q2)*cos(2*q5)*sin(2*q3))/32 + (9*dq1*dqr1*cos(2*q3)*cos(2*q5)*sin(2*q2))/32 - (5*dq1*dqr1*cos(2*q2)*cos(2*q4)*cos(2*q5)*sin(2*q3))/32 + (5*dq1*dqr1*cos(2*q3)*cos(2*q4)*cos(2*q5)*sin(2*q2))/32 + (3^(1/2)*dq1*dqr4*cos(q2)*cos(q3)*sin(q4))/8 + (3^(1/2)*dq4*dqr1*cos(q2)*cos(q3)*sin(q4))/8 + (3^(1/2)*dq1*dqr5*cos(q2)*cos(q3)*sin(q4))/4 + (3^(1/2)*dq5*dqr1*cos(q2)*cos(q3)*sin(q4))/4 + (dq1*dqr1*cos(2*q2)*sin(2*q3)*sin(2*q4)*sin(2*q5))/8 - (dq1*dqr1*cos(2*q3)*sin(2*q2)*sin(2*q4)*sin(2*q5))/8 + (3^(1/2)*dq1*dqr4*sin(q2)*sin(q3)*sin(q4))/8 + (3^(1/2)*dq4*dqr1*sin(q2)*sin(q3)*sin(q4))/8 + (3^(1/2)*dq1*dqr5*sin(q2)*sin(q3)*sin(q4))/4 + (3^(1/2)*dq5*dqr1*sin(q2)*sin(q3)*sin(q4))/4 - (5*dq1*dqr4*cos(2*q4)*cos(2*q5)*cos(q2)*sin(q3))/16 + (5*dq1*dqr4*cos(2*q4)*cos(2*q5)*cos(q3)*sin(q2))/16 - (5*dq4*dqr1*cos(2*q4)*cos(2*q5)*cos(q2)*sin(q3))/16 + (5*dq4*dqr1*cos(2*q4)*cos(2*q5)*cos(q3)*sin(q2))/16 - (dq1*dqr5*cos(2*q4)*cos(2*q5)*cos(q2)*sin(q3))/4 + (dq1*dqr5*cos(2*q4)*cos(2*q5)*cos(q3)*sin(q2))/4 - (dq5*dqr1*cos(2*q4)*cos(2*q5)*cos(q2)*sin(q3))/4 + (dq5*dqr1*cos(2*q4)*cos(2*q5)*cos(q3)*sin(q2))/4 + (dq1*dqr4*sin(2*q4)*sin(2*q5)*cos(q2)*sin(q3))/4 - (dq1*dqr4*sin(2*q4)*sin(2*q5)*cos(q3)*sin(q2))/4 + (dq4*dqr1*sin(2*q4)*sin(2*q5)*cos(q2)*sin(q3))/4 - (dq4*dqr1*sin(2*q4)*sin(2*q5)*cos(q3)*sin(q2))/4 + (5*dq1*dqr5*sin(2*q4)*sin(2*q5)*cos(q2)*sin(q3))/16 - (5*dq1*dqr5*sin(2*q4)*sin(2*q5)*cos(q3)*sin(q2))/16 + (5*dq5*dqr1*sin(2*q4)*sin(2*q5)*cos(q2)*sin(q3))/16 - (5*dq5*dqr1*sin(2*q4)*sin(2*q5)*cos(q3)*sin(q2))/16 + (3^(1/2)*dq1*dqr1*cos(2*q2)*cos(2*q3)*sin(q4))/8 + (3^(1/2)*dq1*dqr1*sin(2*q2)*sin(2*q3)*sin(q4))/8 + (3^(1/2)*dq1*dqr1*cos(2*q2)*cos(2*q3)*cos(2*q5)*sin(q4))/8 + (3^(1/2)*dq1*dqr1*cos(2*q2)*cos(2*q3)*sin(2*q5)*cos(q4))/4 + (3^(1/2)*dq1*dqr1*cos(2*q5)*sin(2*q2)*sin(2*q3)*sin(q4))/8 + (3^(1/2)*dq1*dqr1*sin(2*q2)*sin(2*q3)*sin(2*q5)*cos(q4))/4 + (3^(1/2)*dq1*dqr4*cos(2*q5)*cos(q2)*cos(q3)*sin(q4))/8 + (3^(1/2)*dq1*dqr4*sin(2*q5)*cos(q2)*cos(q3)*cos(q4))/4 + (3^(1/2)*dq4*dqr1*cos(2*q5)*cos(q2)*cos(q3)*sin(q4))/8 + (3^(1/2)*dq4*dqr1*sin(2*q5)*cos(q2)*cos(q3)*cos(q4))/4 + (3^(1/2)*dq1*dqr5*cos(2*q5)*cos(q2)*cos(q3)*sin(q4))/4 + (3^(1/2)*dq1*dqr5*sin(2*q5)*cos(q2)*cos(q3)*cos(q4))/8 + (3^(1/2)*dq5*dqr1*cos(2*q5)*cos(q2)*cos(q3)*sin(q4))/4 + (3^(1/2)*dq5*dqr1*sin(2*q5)*cos(q2)*cos(q3)*cos(q4))/8 + (3^(1/2)*dq1*dqr4*cos(2*q5)*sin(q2)*sin(q3)*sin(q4))/8 + (3^(1/2)*dq1*dqr4*sin(2*q5)*cos(q4)*sin(q2)*sin(q3))/4 + (3^(1/2)*dq4*dqr1*cos(2*q5)*sin(q2)*sin(q3)*sin(q4))/8 + (3^(1/2)*dq4*dqr1*sin(2*q5)*cos(q4)*sin(q2)*sin(q3))/4 + (3^(1/2)*dq1*dqr5*cos(2*q5)*sin(q2)*sin(q3)*sin(q4))/4 + (3^(1/2)*dq1*dqr5*sin(2*q5)*cos(q4)*sin(q2)*sin(q3))/8 + (3^(1/2)*dq5*dqr1*cos(2*q5)*sin(q2)*sin(q3)*sin(q4))/4 + (3^(1/2)*dq5*dqr1*sin(2*q5)*cos(q4)*sin(q2)*sin(q3))/8;
Y3_19_2=ddqr3*cos(q4)^2 - ddqr2*cos(q5)^2 - ddqr2*cos(q4)^2 + ddqr3*cos(q5)^2 + (5*ddqr2*cos(q4)^2*cos(q5)^2)/4 - (5*ddqr3*cos(q4)^2*cos(q5)^2)/4 + (3*dq2*dqr5*sin(2*q5))/16 - (3*dq3*dqr5*sin(2*q5))/16 - (3^(1/2)*ddqr5*cos(q4))/2 - (3^(1/2)*ddqr4*cos(q4)*cos(q5)^2)/4 - (5*dq2*dqr5*cos(2*q4)*sin(2*q5))/16 + (5*dq3*dqr5*cos(2*q4)*sin(2*q5))/16 + (dq3*dqr5*cos(2*q5)*sin(2*q4))/4 + ddqr1*cos(q2)*cos(q4)*sin(q3)*sin(q4) - ddqr1*cos(q3)*cos(q4)*sin(q2)*sin(q4) + (ddqr1*cos(q2)*cos(q5)*sin(q3)*sin(q5))/2 - (ddqr1*cos(q3)*cos(q5)*sin(q2)*sin(q5))/2 - ddqr2*cos(q4)*cos(q5)*sin(q4)*sin(q5) + ddqr3*cos(q4)*cos(q5)*sin(q4)*sin(q5) + (3^(1/2)*ddqr4*cos(q5)*sin(q4)*sin(q5))/2 - (5*ddqr1*cos(q2)*cos(q4)*cos(q5)^2*sin(q3)*sin(q4))/4 + (5*ddqr1*cos(q3)*cos(q4)*cos(q5)^2*sin(q2)*sin(q4))/4 - ddqr1*cos(q2)*cos(q4)^2*cos(q5)*sin(q3)*sin(q5) + ddqr1*cos(q3)*cos(q4)^2*cos(q5)*sin(q2)*sin(q5) - (3^(1/2)*ddqr1*cos(q2)*cos(q3)*cos(q4)*cos(q5)^2)/4 - (3^(1/2)*ddqr1*cos(q4)*cos(q5)^2*sin(q2)*sin(q3))/4 + (3^(1/2)*ddqr1*cos(q2)*cos(q3)*cos(q5)*sin(q4)*sin(q5))/2 + (3^(1/2)*ddqr1*cos(q5)*sin(q2)*sin(q3)*sin(q4)*sin(q5))/2;
Y3_20_1=(3*dq4*dqr1*cos(2*q4)*cos(q3)*sin(q2))/128 - (5*dq5*dqr1*cos(q3)*sin(q2))/32 - (dq6*dqr1*cos(q3)*sin(q2))/8 - (43*dq4*dqr1*cos(q3)*sin(q2))/128 - (9*dq4*dqr1*cos(2*q5)*cos(q3)*sin(q2))/128 - (3*dq4*dqr1*cos(2*q6)*cos(q3)*sin(q2))/128 + (3*dq5*dqr1*cos(2*q6)*cos(q3)*sin(q2))/32 - (3*dq4*dqr1*cos(q3)*cos(q5)*sin(q2))/32 - (3*dq5*dqr1*cos(q3)*cos(q5)*sin(q2))/32 - (3*dq6*dqr1*cos(q3)*cos(q5)*sin(q2))/8 + (3*dq4*dqr1*sin(2*q4)*cos(q2)*sin(q3)*sin(q5))/16 - (3*dq4*dqr1*sin(2*q4)*cos(q3)*sin(q2)*sin(q5))/16 + (3*dq5*dqr1*sin(2*q4)*cos(q2)*sin(q3)*sin(q5))/64 - (3*dq5*dqr1*sin(2*q4)*cos(q3)*sin(q2)*sin(q5))/64 - (3*dq4*dqr1*sin(2*q6)*cos(q2)*sin(q3)*sin(q5))/16 + (3*dq4*dqr1*sin(2*q6)*cos(q3)*sin(q2)*sin(q5))/16 - (3*dq5*dqr1*sin(2*q6)*cos(q2)*sin(q3)*sin(q5))/16 + (3*dq5*dqr1*sin(2*q6)*cos(q3)*sin(q2)*sin(q5))/16 - (3^(1/2)*dq4*dqr1*sin(q2)*sin(q3)*sin(q4))/64 + (5*3^(1/2)*dq5*dqr1*sin(q2)*sin(q3)*sin(q4))/32 + (3^(1/2)*dq6*dqr1*sin(q2)*sin(q3)*sin(q4))/8 - (15*dq4*dqr1*cos(2*q4)*cos(2*q5)*cos(q3)*sin(q2))/128 + (27*dq4*dqr1*cos(2*q4)*cos(2*q6)*cos(q3)*sin(q2))/128 - (3*dq5*dqr1*cos(2*q4)*cos(2*q5)*cos(q3)*sin(q2))/32 + (15*dq4*dqr1*cos(2*q5)*cos(2*q6)*cos(q3)*sin(q2))/128 + (3*dq4*dqr1*sin(2*q4)*sin(2*q5)*cos(q3)*sin(q2))/32 + (15*dq5*dqr1*sin(2*q4)*sin(2*q5)*cos(q3)*sin(q2))/128 - (3*dq4*dqr1*sin(2*q5)*sin(2*q6)*cos(q3)*sin(q2))/32 - (27*dq6*dqr1*sin(2*q4)*sin(2*q6)*cos(q3)*sin(q2))/128 + (3*dq4*dqr1*cos(2*q4)*cos(q3)*cos(q5)*sin(q2))/32 + (3*dq5*dqr1*cos(2*q4)*cos(q3)*cos(q5)*sin(q2))/32 - (3*dq4*dqr1*cos(2*q6)*cos(q3)*cos(q5)*sin(q2))/32 - (3*dq5*dqr1*cos(2*q6)*cos(q3)*cos(q5)*sin(q2))/32 - (3^(1/2)*dq4*dqr1*cos(q4)*sin(q2)*sin(q3)*sin(q5))/16 + (3^(1/2)*dq4*dqr1*cos(q5)*sin(q2)*sin(q3)*sin(q4))/16 - (3^(1/2)*dq5*dqr1*cos(q4)*sin(q2)*sin(q3)*sin(q5))/32 - (3^(1/2)*dq5*dqr1*cos(q5)*sin(q2)*sin(q3)*sin(q4))/16 - (3^(1/2)*dq6*dqr1*cos(q4)*sin(q2)*sin(q3)*sin(q5))/4 - (3^(1/2)*dq6*dqr1*cos(q5)*sin(q2)*sin(q3)*sin(q4))/8 + (3*dq4*dqr1*cos(2*q4)*cos(2*q6)*cos(q3)*cos(q5)*sin(q2))/32 + (3*dq5*dqr1*cos(2*q4)*cos(2*q6)*cos(q3)*cos(q5)*sin(q2))/32 + (3*dq6*dqr1*cos(2*q4)*cos(2*q6)*cos(q3)*cos(q5)*sin(q2))/8 + (3*dq4*dqr1*cos(2*q4)*sin(2*q6)*cos(q2)*sin(q3)*sin(q5))/16 - (3*dq4*dqr1*cos(2*q4)*sin(2*q6)*cos(q3)*sin(q2)*sin(q5))/16 + (3*dq4*dqr1*cos(2*q6)*sin(2*q4)*cos(q2)*sin(q3)*sin(q5))/16 - (3*dq4*dqr1*cos(2*q6)*sin(2*q4)*cos(q3)*sin(q2)*sin(q5))/16 - (3*dq4*dqr1*sin(2*q4)*sin(2*q6)*cos(q3)*cos(q5)*sin(q2))/8 + (3*dq5*dqr1*cos(2*q4)*sin(2*q6)*cos(q2)*sin(q3)*sin(q5))/16 - (3*dq5*dqr1*cos(2*q4)*sin(2*q6)*cos(q3)*sin(q2)*sin(q5))/16 + (3*dq5*dqr1*cos(2*q6)*sin(2*q4)*cos(q2)*sin(q3)*sin(q5))/64 - (3*dq5*dqr1*cos(2*q6)*sin(2*q4)*cos(q3)*sin(q2)*sin(q5))/64 - (3*dq5*dqr1*sin(2*q4)*sin(2*q6)*cos(q3)*cos(q5)*sin(q2))/32 + (3*dq6*dqr1*cos(2*q4)*sin(2*q6)*cos(q2)*sin(q3)*sin(q5))/16 - (3*dq6*dqr1*cos(2*q4)*sin(2*q6)*cos(q3)*sin(q2)*sin(q5))/16 + (3*dq6*dqr1*cos(2*q6)*sin(2*q4)*cos(q2)*sin(q3)*sin(q5))/16 - (3*dq6*dqr1*cos(2*q6)*sin(2*q4)*cos(q3)*sin(q2)*sin(q5))/16 - (3*dq6*dqr1*sin(2*q4)*sin(2*q6)*cos(q3)*cos(q5)*sin(q2))/32 - (3*3^(1/2)*dq4*dqr1*cos(2*q5)*sin(q2)*sin(q3)*sin(q4))/64 - (3*3^(1/2)*dq4*dqr1*sin(2*q5)*cos(q4)*sin(q2)*sin(q3))/32 - (9*3^(1/2)*dq4*dqr1*cos(2*q6)*sin(q2)*sin(q3)*sin(q4))/64 - (3*3^(1/2)*dq5*dqr1*cos(2*q5)*sin(q2)*sin(q3)*sin(q4))/32 - (3*3^(1/2)*dq5*dqr1*sin(2*q5)*cos(q4)*sin(q2)*sin(q3))/64 - (3*3^(1/2)*dq5*dqr1*cos(2*q6)*sin(q2)*sin(q3)*sin(q4))/32 - (9*3^(1/2)*dq6*dqr1*sin(2*q6)*cos(q4)*sin(q2)*sin(q3))/64 + (25*dq4*dqr1*cos(2*q4)*cos(2*q5)*cos(2*q6)*cos(q3)*sin(q2))/128 + (5*dq5*dqr1*cos(2*q4)*cos(2*q5)*cos(2*q6)*cos(q3)*sin(q2))/32 + (dq6*dqr1*cos(2*q4)*cos(2*q5)*cos(2*q6)*cos(q3)*sin(q2))/8 - (5*dq4*dqr1*cos(2*q4)*sin(2*q5)*sin(2*q6)*cos(q3)*sin(q2))/32 - (dq4*dqr1*cos(2*q5)*sin(2*q4)*sin(2*q6)*cos(q3)*sin(q2))/8 - (5*dq4*dqr1*cos(2*q6)*sin(2*q4)*sin(2*q5)*cos(q3)*sin(q2))/32 - (dq5*dqr1*cos(2*q4)*sin(2*q5)*sin(2*q6)*cos(q3)*sin(q2))/8 - (5*dq5*dqr1*cos(2*q5)*sin(2*q4)*sin(2*q6)*cos(q3)*sin(q2))/32 - (25*dq5*dqr1*cos(2*q6)*sin(2*q4)*sin(2*q5)*cos(q3)*sin(q2))/128 - (5*dq6*dqr1*cos(2*q4)*sin(2*q5)*sin(2*q6)*cos(q3)*sin(q2))/32 - (25*dq6*dqr1*cos(2*q5)*sin(2*q4)*sin(2*q6)*cos(q3)*sin(q2))/128 - (5*dq6*dqr1*cos(2*q6)*sin(2*q4)*sin(2*q5)*cos(q3)*sin(q2))/32 - (3^(1/2)*dq4*dqr1*cos(2*q6)*cos(q4)*sin(q2)*sin(q3)*sin(q5))/16 + (3^(1/2)*dq4*dqr1*cos(2*q6)*cos(q5)*sin(q2)*sin(q3)*sin(q4))/16 - (3^(1/2)*dq4*dqr1*sin(2*q6)*cos(q4)*cos(q5)*sin(q2)*sin(q3))/8 - (3^(1/2)*dq5*dqr1*cos(2*q6)*cos(q4)*sin(q2)*sin(q3)*sin(q5))/32 - (3^(1/2)*dq5*dqr1*cos(2*q6)*cos(q5)*sin(q2)*sin(q3)*sin(q4))/16 - (3^(1/2)*dq5*dqr1*sin(2*q6)*cos(q4)*cos(q5)*sin(q2)*sin(q3))/16 + (3^(1/2)*dq6*dqr1*cos(2*q6)*cos(q4)*sin(q2)*sin(q3)*sin(q5))/8 - (3^(1/2)*dq6*dqr1*cos(2*q6)*cos(q5)*sin(q2)*sin(q3)*sin(q4))/8 + (3^(1/2)*dq6*dqr1*sin(2*q6)*cos(q4)*cos(q5)*sin(q2)*sin(q3))/16 - (3^(1/2)*dq4*dqr1*sin(2*q6)*sin(q2)*sin(q3)*sin(q4)*sin(q5))/8 + (3^(1/2)*dq5*dqr1*sin(2*q6)*sin(q2)*sin(q3)*sin(q4)*sin(q5))/8 + (3^(1/2)*dq6*dqr1*sin(2*q6)*sin(q2)*sin(q3)*sin(q4)*sin(q5))/16 + (5*3^(1/2)*dq4*dqr1*cos(2*q5)*cos(2*q6)*sin(q2)*sin(q3)*sin(q4))/64 + (3^(1/2)*dq4*dqr1*cos(2*q5)*sin(2*q6)*cos(q4)*sin(q2)*sin(q3))/8 + (5*3^(1/2)*dq4*dqr1*cos(2*q6)*sin(2*q5)*cos(q4)*sin(q2)*sin(q3))/32 + (5*3^(1/2)*dq5*dqr1*cos(2*q5)*cos(2*q6)*sin(q2)*sin(q3)*sin(q4))/32 + (3^(1/2)*dq5*dqr1*cos(2*q5)*sin(2*q6)*cos(q4)*sin(q2)*sin(q3))/16 + (5*3^(1/2)*dq5*dqr1*cos(2*q6)*sin(2*q5)*cos(q4)*sin(q2)*sin(q3))/64 + (3^(1/2)*dq6*dqr1*cos(2*q5)*cos(2*q6)*sin(q2)*sin(q3)*sin(q4))/8 + (5*3^(1/2)*dq6*dqr1*cos(2*q5)*sin(2*q6)*cos(q4)*sin(q2)*sin(q3))/64 + (3^(1/2)*dq6*dqr1*cos(2*q6)*sin(2*q5)*cos(q4)*sin(q2)*sin(q3))/16 - (3^(1/2)*dq4*dqr1*sin(2*q5)*sin(2*q6)*sin(q2)*sin(q3)*sin(q4))/16 - (3^(1/2)*dq5*dqr1*sin(2*q5)*sin(2*q6)*sin(q2)*sin(q3)*sin(q4))/8 - (5*3^(1/2)*dq6*dqr1*sin(2*q5)*sin(2*q6)*sin(q2)*sin(q3)*sin(q4))/32;
Y3_20_2=(43*dq4*dqr1*cos(q2)*sin(q3))/128 + (5*dq5*dqr1*cos(q2)*sin(q3))/32 + (dq6*dqr1*cos(q2)*sin(q3))/8 - (3*dq4*dqr1*cos(2*q4)*cos(q2)*sin(q3))/128 + (9*dq4*dqr1*cos(2*q5)*cos(q2)*sin(q3))/128 + (3*dq4*dqr1*cos(2*q6)*cos(q2)*sin(q3))/128 - (3*dq5*dqr1*cos(2*q6)*cos(q2)*sin(q3))/32 + (3*dq4*dqr1*cos(q2)*cos(q5)*sin(q3))/32 + (3*dq5*dqr1*cos(q2)*cos(q5)*sin(q3))/32 + (3*dq6*dqr1*cos(q2)*cos(q5)*sin(q3))/8 - (3^(1/2)*dq4*dqr1*cos(q2)*cos(q3)*sin(q4))/64 + (5*3^(1/2)*dq5*dqr1*cos(q2)*cos(q3)*sin(q4))/32 + (3^(1/2)*dq6*dqr1*cos(q2)*cos(q3)*sin(q4))/8 + (15*dq4*dqr1*cos(2*q4)*cos(2*q5)*cos(q2)*sin(q3))/128 - (27*dq4*dqr1*cos(2*q4)*cos(2*q6)*cos(q2)*sin(q3))/128 + (3*dq5*dqr1*cos(2*q4)*cos(2*q5)*cos(q2)*sin(q3))/32 - (15*dq4*dqr1*cos(2*q5)*cos(2*q6)*cos(q2)*sin(q3))/128 - (3*dq4*dqr1*sin(2*q4)*sin(2*q5)*cos(q2)*sin(q3))/32 - (15*dq5*dqr1*sin(2*q4)*sin(2*q5)*cos(q2)*sin(q3))/128 + (3*dq4*dqr1*sin(2*q5)*sin(2*q6)*cos(q2)*sin(q3))/32 + (27*dq6*dqr1*sin(2*q4)*sin(2*q6)*cos(q2)*sin(q3))/128 + (3*dq1*dqr1*cos(2*q2)*sin(2*q3)*sin(2*q4)*sin(q5))/32 - (3*dq1*dqr1*cos(2*q3)*sin(2*q2)*sin(2*q4)*sin(q5))/32 - (9*dq1*dqr1*cos(2*q2)*sin(2*q3)*sin(2*q6)*sin(q5))/32 + (9*dq1*dqr1*cos(2*q3)*sin(2*q2)*sin(2*q6)*sin(q5))/32 - (3^(1/2)*dq1*dqr1*cos(2*q2)*cos(2*q3)*sin(q4))/64 - (3*dq4*dqr1*cos(2*q4)*cos(q2)*cos(q5)*sin(q3))/32 - (3*dq5*dqr1*cos(2*q4)*cos(q2)*cos(q5)*sin(q3))/32 + (3*dq4*dqr1*cos(2*q6)*cos(q2)*cos(q5)*sin(q3))/32 + (3*dq5*dqr1*cos(2*q6)*cos(q2)*cos(q5)*sin(q3))/32 - (3^(1/2)*dq1*dqr1*sin(2*q2)*sin(2*q3)*sin(q4))/64 - (3*3^(1/2)*dq1*dqr1*cos(2*q2)*cos(2*q3)*cos(2*q5)*sin(q4))/64 - (9*3^(1/2)*dq1*dqr1*cos(2*q2)*cos(2*q3)*cos(2*q6)*sin(q4))/64 - (3*dq4*dqr1*cos(2*q4)*cos(2*q6)*cos(q2)*cos(q5)*sin(q3))/32 - (3*dq5*dqr1*cos(2*q4)*cos(2*q6)*cos(q2)*cos(q5)*sin(q3))/32 - (3*dq6*dqr1*cos(2*q4)*cos(2*q6)*cos(q2)*cos(q5)*sin(q3))/8 - (3*3^(1/2)*dq1*dqr1*cos(2*q5)*sin(2*q2)*sin(2*q3)*sin(q4))/64 - (9*3^(1/2)*dq1*dqr1*cos(2*q6)*sin(2*q2)*sin(2*q3)*sin(q4))/64 + (3*dq4*dqr1*sin(2*q4)*sin(2*q6)*cos(q2)*cos(q5)*sin(q3))/8 + (3*dq5*dqr1*sin(2*q4)*sin(2*q6)*cos(q2)*cos(q5)*sin(q3))/32 + (3*dq6*dqr1*sin(2*q4)*sin(2*q6)*cos(q2)*cos(q5)*sin(q3))/32 - (3*3^(1/2)*dq4*dqr1*cos(2*q5)*cos(q2)*cos(q3)*sin(q4))/64 - (9*3^(1/2)*dq4*dqr1*cos(2*q6)*cos(q2)*cos(q3)*sin(q4))/64 - (3*3^(1/2)*dq5*dqr1*cos(2*q5)*cos(q2)*cos(q3)*sin(q4))/32 - (3*3^(1/2)*dq5*dqr1*cos(2*q6)*cos(q2)*cos(q3)*sin(q4))/32 - (25*dq4*dqr1*cos(2*q4)*cos(2*q5)*cos(2*q6)*cos(q2)*sin(q3))/128 - (5*dq5*dqr1*cos(2*q4)*cos(2*q5)*cos(2*q6)*cos(q2)*sin(q3))/32 - (dq6*dqr1*cos(2*q4)*cos(2*q5)*cos(2*q6)*cos(q2)*sin(q3))/8 + (5*dq4*dqr1*cos(2*q4)*sin(2*q5)*sin(2*q6)*cos(q2)*sin(q3))/32 + (dq4*dqr1*cos(2*q5)*sin(2*q4)*sin(2*q6)*cos(q2)*sin(q3))/8 + (5*dq4*dqr1*cos(2*q6)*sin(2*q4)*sin(2*q5)*cos(q2)*sin(q3))/32 + (dq5*dqr1*cos(2*q4)*sin(2*q5)*sin(2*q6)*cos(q2)*sin(q3))/8 + (5*dq5*dqr1*cos(2*q5)*sin(2*q4)*sin(2*q6)*cos(q2)*sin(q3))/32 + (25*dq5*dqr1*cos(2*q6)*sin(2*q4)*sin(2*q5)*cos(q2)*sin(q3))/128 + (5*dq6*dqr1*cos(2*q4)*sin(2*q5)*sin(2*q6)*cos(q2)*sin(q3))/32 + (25*dq6*dqr1*cos(2*q5)*sin(2*q4)*sin(2*q6)*cos(q2)*sin(q3))/128 + (5*dq6*dqr1*cos(2*q6)*sin(2*q4)*sin(2*q5)*cos(q2)*sin(q3))/32 - (3^(1/2)*dq1*dqr1*cos(2*q2)*cos(2*q3)*cos(q4)*sin(q5))/16 + (3^(1/2)*dq1*dqr1*cos(2*q2)*cos(2*q3)*cos(q5)*sin(q4))/16 - (3^(1/2)*dq1*dqr1*sin(2*q2)*sin(2*q3)*cos(q4)*sin(q5))/16 + (3^(1/2)*dq1*dqr1*sin(2*q2)*sin(2*q3)*cos(q5)*sin(q4))/16 - (3^(1/2)*dq4*dqr1*cos(q2)*cos(q3)*cos(q4)*sin(q5))/16 + (3^(1/2)*dq4*dqr1*cos(q2)*cos(q3)*cos(q5)*sin(q4))/16 - (3^(1/2)*dq5*dqr1*cos(q2)*cos(q3)*cos(q4)*sin(q5))/32 - (3^(1/2)*dq5*dqr1*cos(q2)*cos(q3)*cos(q5)*sin(q4))/16 - (3^(1/2)*dq6*dqr1*cos(q2)*cos(q3)*cos(q4)*sin(q5))/4 - (3^(1/2)*dq6*dqr1*cos(q2)*cos(q3)*cos(q5)*sin(q4))/8 + (3*dq1*dqr1*cos(2*q2)*cos(2*q4)*sin(2*q3)*sin(2*q6)*sin(q5))/32 + (3*dq1*dqr1*cos(2*q2)*cos(2*q6)*sin(2*q3)*sin(2*q4)*sin(q5))/32 - (3*dq1*dqr1*cos(2*q3)*cos(2*q4)*sin(2*q2)*sin(2*q6)*sin(q5))/32 - (3*dq1*dqr1*cos(2*q3)*cos(2*q6)*sin(2*q2)*sin(2*q4)*sin(q5))/32 - (3^(1/2)*dq1*dqr1*sin(2*q2)*sin(2*q3)*sin(2*q6)*sin(q4)*sin(q5))/8 - (3^(1/2)*dq4*dqr1*cos(2*q6)*cos(q2)*cos(q3)*cos(q4)*sin(q5))/16 + (3^(1/2)*dq4*dqr1*cos(2*q6)*cos(q2)*cos(q3)*cos(q5)*sin(q4))/16 - (3^(1/2)*dq4*dqr1*sin(2*q6)*cos(q2)*cos(q3)*cos(q4)*cos(q5))/8 - (3^(1/2)*dq5*dqr1*cos(2*q6)*cos(q2)*cos(q3)*cos(q4)*sin(q5))/32 - (3^(1/2)*dq5*dqr1*cos(2*q6)*cos(q2)*cos(q3)*cos(q5)*sin(q4))/16 - (3^(1/2)*dq5*dqr1*sin(2*q6)*cos(q2)*cos(q3)*cos(q4)*cos(q5))/16 + (3^(1/2)*dq6*dqr1*cos(2*q6)*cos(q2)*cos(q3)*cos(q4)*sin(q5))/8 - (3^(1/2)*dq6*dqr1*cos(2*q6)*cos(q2)*cos(q3)*cos(q5)*sin(q4))/8 + (3^(1/2)*dq6*dqr1*sin(2*q6)*cos(q2)*cos(q3)*cos(q4)*cos(q5))/16 + (5*3^(1/2)*dq1*dqr1*cos(2*q2)*cos(2*q3)*cos(2*q5)*cos(2*q6)*sin(q4))/64 - (3^(1/2)*dq4*dqr1*sin(2*q6)*cos(q2)*cos(q3)*sin(q4)*sin(q5))/8 + (3^(1/2)*dq5*dqr1*sin(2*q6)*cos(q2)*cos(q3)*sin(q4)*sin(q5))/8 + (3^(1/2)*dq6*dqr1*sin(2*q6)*cos(q2)*cos(q3)*sin(q4)*sin(q5))/16 - (3^(1/2)*dq1*dqr1*cos(2*q2)*cos(2*q3)*sin(2*q5)*sin(2*q6)*sin(q4))/16 + (5*3^(1/2)*dq1*dqr1*cos(2*q5)*cos(2*q6)*sin(2*q2)*sin(2*q3)*sin(q4))/64 - (3^(1/2)*dq1*dqr1*sin(2*q2)*sin(2*q3)*sin(2*q5)*sin(2*q6)*sin(q4))/16 + (5*3^(1/2)*dq4*dqr1*cos(2*q5)*cos(2*q6)*cos(q2)*cos(q3)*sin(q4))/64 + (5*3^(1/2)*dq4*dqr1*cos(2*q6)*sin(2*q5)*cos(q2)*cos(q3)*cos(q4))/32 + (5*3^(1/2)*dq5*dqr1*cos(2*q5)*cos(2*q6)*cos(q2)*cos(q3)*sin(q4))/32 + (3^(1/2)*dq6*dqr1*cos(2*q5)*cos(2*q6)*cos(q2)*cos(q3)*sin(q4))/8 - (3^(1/2)*dq4*dqr1*sin(2*q5)*sin(2*q6)*cos(q2)*cos(q3)*sin(q4))/16 - (3^(1/2)*dq5*dqr1*sin(2*q5)*sin(2*q6)*cos(q2)*cos(q3)*sin(q4))/8 - (5*3^(1/2)*dq6*dqr1*sin(2*q5)*sin(2*q6)*cos(q2)*cos(q3)*sin(q4))/32 - (3^(1/2)*dq1*dqr1*cos(2*q2)*cos(2*q3)*cos(2*q6)*cos(q4)*sin(q5))/16 + (3^(1/2)*dq1*dqr1*cos(2*q2)*cos(2*q3)*cos(2*q6)*cos(q5)*sin(q4))/16 - (3^(1/2)*dq1*dqr1*cos(2*q2)*cos(2*q3)*sin(2*q6)*sin(q4)*sin(q5))/8 - (3^(1/2)*dq1*dqr1*cos(2*q6)*sin(2*q2)*sin(2*q3)*cos(q4)*sin(q5))/16 + (3^(1/2)*dq1*dqr1*cos(2*q6)*sin(2*q2)*sin(2*q3)*cos(q5)*sin(q4))/16;
Y3_20_3=(dq1*dqr1*cos(2*q2)*sin(2*q3))/256 - (3*dq4*dqr2*sin(2*q4))/128 - (9*dq5*dqr2*sin(2*q5))/128 - (3*dq6*dqr2*sin(2*q6))/128 - (3*dq4*dqr2*cos(2*q4)*sin(q5))/16 - (3*dq4*dqr2*sin(2*q4)*cos(q5))/32 - (3*dq5*dqr2*cos(2*q4)*sin(q5))/64 - (3*dq5*dqr2*sin(2*q4)*cos(q5))/32 - (3*dq5*dqr2*cos(2*q6)*sin(q5))/64 - (3*dq5*dqr2*sin(2*q6)*cos(q5))/32 - (3*dq6*dqr2*cos(2*q6)*sin(q5))/16 - (3*dq6*dqr2*sin(2*q6)*cos(q5))/32 - (3*dq5*dqr2*sin(q5))/64 - (dq1*dqr1*cos(2*q3)*sin(2*q2))/256 + (3*dq4*dqr2*cos(2*q4)*sin(2*q5))/32 + (15*dq4*dqr2*cos(2*q5)*sin(2*q4))/128 - (27*dq4*dqr2*cos(2*q6)*sin(2*q4))/128 + (15*dq5*dqr2*cos(2*q4)*sin(2*q5))/128 + (3*dq5*dqr2*cos(2*q5)*sin(2*q4))/32 + (3*dq5*dqr2*cos(2*q5)*sin(2*q6))/32 + (15*dq5*dqr2*cos(2*q6)*sin(2*q5))/128 - (27*dq6*dqr2*cos(2*q4)*sin(2*q6))/128 + (15*dq6*dqr2*cos(2*q5)*sin(2*q6))/128 + (3*dq6*dqr2*cos(2*q6)*sin(2*q5))/32 + (9*dq1*dqr1*cos(2*q2)*sin(2*q3)*cos(q5))/64 - (9*dq1*dqr1*cos(2*q3)*sin(2*q2)*cos(q5))/64 - (3*dq4*dqr2*cos(2*q4)*cos(2*q6)*sin(q5))/16 - (3*dq4*dqr2*cos(2*q4)*sin(2*q6)*cos(q5))/8 - (3*dq4*dqr2*cos(2*q6)*sin(2*q4)*cos(q5))/32 + (3*dq4*dqr3*cos(2*q4)*cos(2*q6)*sin(q5))/16 - (3*dq5*dqr2*cos(2*q4)*cos(2*q6)*sin(q5))/64 - (3*dq5*dqr2*cos(2*q4)*sin(2*q6)*cos(q5))/32 - (3*dq5*dqr2*cos(2*q6)*sin(2*q4)*cos(q5))/32 - (3*dq6*dqr2*cos(2*q4)*cos(2*q6)*sin(q5))/16 - (3*dq6*dqr2*cos(2*q4)*sin(2*q6)*cos(q5))/32 - (3*dq6*dqr2*cos(2*q6)*sin(2*q4)*cos(q5))/8 + (3*dq4*dqr2*sin(2*q4)*sin(2*q6)*sin(q5))/16 - (3*dq4*dqr3*sin(2*q4)*sin(2*q6)*sin(q5))/16 + (3*dq5*dqr2*sin(2*q4)*sin(2*q6)*sin(q5))/16 + (3*dq6*dqr2*sin(2*q4)*sin(2*q6)*sin(q5))/16 - (3*dq1*dqr1*cos(2*q2)*cos(2*q4)*sin(2*q3))/256 + (3*dq1*dqr1*cos(2*q3)*cos(2*q4)*sin(2*q2))/256 + (27*dq1*dqr1*cos(2*q2)*cos(2*q5)*sin(2*q3))/256 - (27*dq1*dqr1*cos(2*q3)*cos(2*q5)*sin(2*q2))/256 + (9*dq1*dqr1*cos(2*q2)*cos(2*q6)*sin(2*q3))/256 - (9*dq1*dqr1*cos(2*q3)*cos(2*q6)*sin(2*q2))/256 - (dq4*dqr2*cos(2*q4)*cos(2*q5)*sin(2*q6))/8 - (5*dq4*dqr2*cos(2*q4)*cos(2*q6)*sin(2*q5))/32 - (25*dq4*dqr2*cos(2*q5)*cos(2*q6)*sin(2*q4))/128 - (5*dq5*dqr2*cos(2*q4)*cos(2*q5)*sin(2*q6))/32 - (25*dq5*dqr2*cos(2*q4)*cos(2*q6)*sin(2*q5))/128 - (5*dq5*dqr2*cos(2*q5)*cos(2*q6)*sin(2*q4))/32 - (25*dq6*dqr2*cos(2*q4)*cos(2*q5)*sin(2*q6))/128 - (5*dq6*dqr2*cos(2*q4)*cos(2*q6)*sin(2*q5))/32 - (dq6*dqr2*cos(2*q5)*cos(2*q6)*sin(2*q4))/8 + (5*dq4*dqr2*sin(2*q4)*sin(2*q5)*sin(2*q6))/32 + (dq5*dqr2*sin(2*q4)*sin(2*q5)*sin(2*q6))/8 + (5*dq6*dqr2*sin(2*q4)*sin(2*q5)*sin(2*q6))/32 + (15*dq1*dqr1*cos(2*q2)*cos(2*q4)*cos(2*q5)*sin(2*q3))/256 - (15*dq1*dqr1*cos(2*q3)*cos(2*q4)*cos(2*q5)*sin(2*q2))/256 - (27*dq1*dqr1*cos(2*q2)*cos(2*q4)*cos(2*q6)*sin(2*q3))/256 + (27*dq1*dqr1*cos(2*q3)*cos(2*q4)*cos(2*q6)*sin(2*q2))/256 - (45*dq1*dqr1*cos(2*q2)*cos(2*q5)*cos(2*q6)*sin(2*q3))/256 + (45*dq1*dqr1*cos(2*q3)*cos(2*q5)*cos(2*q6)*sin(2*q2))/256 - (3*dq1*dqr1*cos(2*q2)*sin(2*q3)*sin(2*q4)*sin(2*q5))/64 + (3*dq1*dqr1*cos(2*q3)*sin(2*q2)*sin(2*q4)*sin(2*q5))/64 + (9*dq1*dqr1*cos(2*q2)*sin(2*q3)*sin(2*q5)*sin(2*q6))/64 - (9*dq1*dqr1*cos(2*q3)*sin(2*q2)*sin(2*q5)*sin(2*q6))/64 - (3*dq1*dqr1*cos(2*q2)*cos(2*q4)*sin(2*q3)*cos(q5))/64 + (3*dq1*dqr1*cos(2*q3)*cos(2*q4)*sin(2*q2)*cos(q5))/64 + (9*dq1*dqr1*cos(2*q2)*cos(2*q6)*sin(2*q3)*cos(q5))/64 - (9*dq1*dqr1*cos(2*q3)*cos(2*q6)*sin(2*q2)*cos(q5))/64 - (3*3^(1/2)*dq1*dqr1*cos(2*q2)*cos(2*q3)*sin(2*q5)*cos(q4))/32 - (3*3^(1/2)*dq1*dqr1*sin(2*q2)*sin(2*q3)*sin(2*q5)*cos(q4))/32 - (25*dq1*dqr1*cos(2*q2)*cos(2*q4)*cos(2*q5)*cos(2*q6)*sin(2*q3))/256 + (25*dq1*dqr1*cos(2*q3)*cos(2*q4)*cos(2*q5)*cos(2*q6)*sin(2*q2))/256 - (3*3^(1/2)*dq4*dqr1*sin(2*q5)*cos(q2)*cos(q3)*cos(q4))/32 - (3*3^(1/2)*dq5*dqr1*sin(2*q5)*cos(q2)*cos(q3)*cos(q4))/64 - (9*3^(1/2)*dq6*dqr1*sin(2*q6)*cos(q2)*cos(q3)*cos(q4))/64 + (5*dq1*dqr1*cos(2*q2)*cos(2*q4)*sin(2*q3)*sin(2*q5)*sin(2*q6))/64 + (dq1*dqr1*cos(2*q2)*cos(2*q5)*sin(2*q3)*sin(2*q4)*sin(2*q6))/16 + (5*dq1*dqr1*cos(2*q2)*cos(2*q6)*sin(2*q3)*sin(2*q4)*sin(2*q5))/64 - (5*dq1*dqr1*cos(2*q3)*cos(2*q4)*sin(2*q2)*sin(2*q5)*sin(2*q6))/64 - (dq1*dqr1*cos(2*q3)*cos(2*q5)*sin(2*q2)*sin(2*q4)*sin(2*q6))/16 - (5*dq1*dqr1*cos(2*q3)*cos(2*q6)*sin(2*q2)*sin(2*q4)*sin(2*q5))/64 - (3*dq1*dqr1*cos(2*q2)*cos(2*q4)*cos(2*q6)*sin(2*q3)*cos(q5))/64 + (3*dq1*dqr1*cos(2*q3)*cos(2*q4)*cos(2*q6)*sin(2*q2)*cos(q5))/64 + (3*dq1*dqr1*cos(2*q2)*sin(2*q3)*sin(2*q4)*sin(2*q6)*cos(q5))/16 - (3*dq1*dqr1*cos(2*q3)*sin(2*q2)*sin(2*q4)*sin(2*q6)*cos(q5))/16 + (3^(1/2)*dq1*dqr1*cos(2*q2)*cos(2*q3)*cos(2*q5)*sin(2*q6)*cos(q4))/8 + (5*3^(1/2)*dq1*dqr1*cos(2*q2)*cos(2*q3)*cos(2*q6)*sin(2*q5)*cos(q4))/32 + (3^(1/2)*dq1*dqr1*cos(2*q5)*sin(2*q2)*sin(2*q3)*sin(2*q6)*cos(q4))/8 + (5*3^(1/2)*dq1*dqr1*cos(2*q6)*sin(2*q2)*sin(2*q3)*sin(2*q5)*cos(q4))/32 + (3^(1/2)*dq4*dqr1*cos(2*q5)*sin(2*q6)*cos(q2)*cos(q3)*cos(q4))/8 + (3^(1/2)*dq5*dqr1*cos(2*q5)*sin(2*q6)*cos(q2)*cos(q3)*cos(q4))/16 + (5*3^(1/2)*dq5*dqr1*cos(2*q6)*sin(2*q5)*cos(q2)*cos(q3)*cos(q4))/64 + (5*3^(1/2)*dq6*dqr1*cos(2*q5)*sin(2*q6)*cos(q2)*cos(q3)*cos(q4))/64 + (3^(1/2)*dq6*dqr1*cos(2*q6)*sin(2*q5)*cos(q2)*cos(q3)*cos(q4))/16 - (3^(1/2)*dq1*dqr1*cos(2*q2)*cos(2*q3)*sin(2*q6)*cos(q4)*cos(q5))/8 - (3^(1/2)*dq1*dqr1*sin(2*q2)*sin(2*q3)*sin(2*q6)*cos(q4)*cos(q5))/8;
Y3_20_4=(3*dq5*dqr3*sin(q5))/64 + (3*dq4*dqr3*sin(2*q4))/128 + (9*dq5*dqr3*sin(2*q5))/128 + (3*dq6*dqr3*sin(2*q6))/128 + (3*dq4*dqr3*cos(2*q4)*sin(q5))/16 + (3*dq4*dqr3*sin(2*q4)*cos(q5))/32 + (3*dq5*dqr3*cos(2*q4)*sin(q5))/64 + (3*dq5*dqr3*sin(2*q4)*cos(q5))/32 + (3*dq5*dqr3*cos(2*q6)*sin(q5))/64 + (3*dq5*dqr3*sin(2*q6)*cos(q5))/32 + (3*dq6*dqr3*cos(2*q6)*sin(q5))/16 + (3*dq6*dqr3*sin(2*q6)*cos(q5))/32 - (3*dq4*dqr3*cos(2*q4)*sin(2*q5))/32 - (15*dq4*dqr3*cos(2*q5)*sin(2*q4))/128 + (27*dq4*dqr3*cos(2*q6)*sin(2*q4))/128 - (15*dq5*dqr3*cos(2*q4)*sin(2*q5))/128 - (3*dq5*dqr3*cos(2*q5)*sin(2*q4))/32 - (3*dq5*dqr3*cos(2*q5)*sin(2*q6))/32 - (15*dq5*dqr3*cos(2*q6)*sin(2*q5))/128 + (27*dq6*dqr3*cos(2*q4)*sin(2*q6))/128 - (15*dq6*dqr3*cos(2*q5)*sin(2*q6))/128 - (3*dq6*dqr3*cos(2*q6)*sin(2*q5))/32 - (43*dq1*dqr4*cos(q3)*sin(q2))/128 - (3*dq1*dqr4*cos(2*q4)*cos(q2)*sin(q3))/128 + (3*dq1*dqr4*cos(2*q4)*cos(q3)*sin(q2))/128 + (9*dq1*dqr4*cos(2*q5)*cos(q2)*sin(q3))/128 - (9*dq1*dqr4*cos(2*q5)*cos(q3)*sin(q2))/128 - (3*dq1*dqr4*cos(2*q6)*cos(q3)*sin(q2))/128 + (3*dq4*dqr3*cos(2*q4)*sin(2*q6)*cos(q5))/8 + (3*dq4*dqr3*cos(2*q6)*sin(2*q4)*cos(q5))/32 + (3*dq5*dqr3*cos(2*q4)*cos(2*q6)*sin(q5))/64 + (3*dq5*dqr3*cos(2*q4)*sin(2*q6)*cos(q5))/32 + (3*dq5*dqr3*cos(2*q6)*sin(2*q4)*cos(q5))/32 + (3*dq6*dqr3*cos(2*q4)*cos(2*q6)*sin(q5))/16 + (3*dq6*dqr3*cos(2*q4)*sin(2*q6)*cos(q5))/32 + (3*dq6*dqr3*cos(2*q6)*sin(2*q4)*cos(q5))/8 - (3*dq5*dqr3*sin(2*q4)*sin(2*q6)*sin(q5))/16 - (3*dq6*dqr3*sin(2*q4)*sin(2*q6)*sin(q5))/16 + (3*dq1*dqr4*cos(q2)*cos(q5)*sin(q3))/32 - (3*dq1*dqr4*cos(q3)*cos(q5)*sin(q2))/32 + (dq4*dqr3*cos(2*q4)*cos(2*q5)*sin(2*q6))/8 + (5*dq4*dqr3*cos(2*q4)*cos(2*q6)*sin(2*q5))/32 + (25*dq4*dqr3*cos(2*q5)*cos(2*q6)*sin(2*q4))/128 + (5*dq5*dqr3*cos(2*q4)*cos(2*q5)*sin(2*q6))/32 + (25*dq5*dqr3*cos(2*q4)*cos(2*q6)*sin(2*q5))/128 + (5*dq5*dqr3*cos(2*q5)*cos(2*q6)*sin(2*q4))/32 + (25*dq6*dqr3*cos(2*q4)*cos(2*q5)*sin(2*q6))/128 + (5*dq6*dqr3*cos(2*q4)*cos(2*q6)*sin(2*q5))/32 + (dq6*dqr3*cos(2*q5)*cos(2*q6)*sin(2*q4))/8 - (5*dq4*dqr3*sin(2*q4)*sin(2*q5)*sin(2*q6))/32 - (dq5*dqr3*sin(2*q4)*sin(2*q5)*sin(2*q6))/8 - (5*dq6*dqr3*sin(2*q4)*sin(2*q5)*sin(2*q6))/32 + (3*dq1*dqr4*sin(2*q4)*cos(q2)*sin(q3)*sin(q5))/16 - (3*dq1*dqr4*sin(2*q4)*cos(q3)*sin(q2)*sin(q5))/16 - (3*dq1*dqr4*sin(2*q6)*cos(q2)*sin(q3)*sin(q5))/16 + (3*dq1*dqr4*sin(2*q6)*cos(q3)*sin(q2)*sin(q5))/16 - (3^(1/2)*dq1*dqr4*sin(q2)*sin(q3)*sin(q4))/64 + (15*dq1*dqr4*cos(2*q4)*cos(2*q5)*cos(q2)*sin(q3))/128 - (15*dq1*dqr4*cos(2*q4)*cos(2*q5)*cos(q3)*sin(q2))/128 - (27*dq1*dqr4*cos(2*q4)*cos(2*q6)*cos(q2)*sin(q3))/128 + (27*dq1*dqr4*cos(2*q4)*cos(2*q6)*cos(q3)*sin(q2))/128 - (15*dq1*dqr4*cos(2*q5)*cos(2*q6)*cos(q2)*sin(q3))/128 + (15*dq1*dqr4*cos(2*q5)*cos(2*q6)*cos(q3)*sin(q2))/128 - (3*dq1*dqr4*sin(2*q4)*sin(2*q5)*cos(q2)*sin(q3))/32 + (3*dq1*dqr4*sin(2*q4)*sin(2*q5)*cos(q3)*sin(q2))/32 + (3*dq1*dqr4*sin(2*q5)*sin(2*q6)*cos(q2)*sin(q3))/32 - (3*dq1*dqr4*sin(2*q5)*sin(2*q6)*cos(q3)*sin(q2))/32 - (3*dq1*dqr4*cos(2*q4)*cos(q2)*cos(q5)*sin(q3))/32 + (3*dq1*dqr4*cos(2*q4)*cos(q3)*cos(q5)*sin(q2))/32 + (3*dq1*dqr4*cos(2*q6)*cos(q2)*cos(q5)*sin(q3))/32 - (3*dq1*dqr4*cos(2*q6)*cos(q3)*cos(q5)*sin(q2))/32 - (3^(1/2)*dq1*dqr4*cos(q4)*sin(q2)*sin(q3)*sin(q5))/16 + (3^(1/2)*dq1*dqr4*cos(q5)*sin(q2)*sin(q3)*sin(q4))/16 - (3*dq1*dqr4*cos(2*q4)*cos(2*q6)*cos(q2)*cos(q5)*sin(q3))/32 + (3*dq1*dqr4*cos(2*q4)*cos(2*q6)*cos(q3)*cos(q5)*sin(q2))/32 + (3*dq1*dqr4*cos(2*q4)*sin(2*q6)*cos(q2)*sin(q3)*sin(q5))/16 - (3*dq1*dqr4*cos(2*q4)*sin(2*q6)*cos(q3)*sin(q2)*sin(q5))/16 + (3*dq1*dqr4*cos(2*q6)*sin(2*q4)*cos(q2)*sin(q3)*sin(q5))/16 - (3*dq1*dqr4*cos(2*q6)*sin(2*q4)*cos(q3)*sin(q2)*sin(q5))/16 + (3*dq1*dqr4*sin(2*q4)*sin(2*q6)*cos(q2)*cos(q5)*sin(q3))/8 - (3*dq1*dqr4*sin(2*q4)*sin(2*q6)*cos(q3)*cos(q5)*sin(q2))/8 - (3*3^(1/2)*dq1*dqr4*cos(2*q5)*sin(q2)*sin(q3)*sin(q4))/64 - (3*3^(1/2)*dq1*dqr4*sin(2*q5)*cos(q4)*sin(q2)*sin(q3))/32 - (9*3^(1/2)*dq1*dqr4*cos(2*q6)*sin(q2)*sin(q3)*sin(q4))/64 - (25*dq1*dqr4*cos(2*q4)*cos(2*q5)*cos(2*q6)*cos(q2)*sin(q3))/128 + (25*dq1*dqr4*cos(2*q4)*cos(2*q5)*cos(2*q6)*cos(q3)*sin(q2))/128 + (5*dq1*dqr4*cos(2*q4)*sin(2*q5)*sin(2*q6)*cos(q2)*sin(q3))/32 - (5*dq1*dqr4*cos(2*q4)*sin(2*q5)*sin(2*q6)*cos(q3)*sin(q2))/32 + (dq1*dqr4*cos(2*q5)*sin(2*q4)*sin(2*q6)*cos(q2)*sin(q3))/8 - (dq1*dqr4*cos(2*q5)*sin(2*q4)*sin(2*q6)*cos(q3)*sin(q2))/8 + (5*dq1*dqr4*cos(2*q6)*sin(2*q4)*sin(2*q5)*cos(q2)*sin(q3))/32 - (5*dq1*dqr4*cos(2*q6)*sin(2*q4)*sin(2*q5)*cos(q3)*sin(q2))/32 - (3^(1/2)*dq1*dqr4*cos(2*q6)*cos(q4)*sin(q2)*sin(q3)*sin(q5))/16 + (3^(1/2)*dq1*dqr4*cos(2*q6)*cos(q5)*sin(q2)*sin(q3)*sin(q4))/16 - (3^(1/2)*dq1*dqr4*sin(2*q6)*cos(q4)*cos(q5)*sin(q2)*sin(q3))/8 - (3^(1/2)*dq1*dqr4*sin(2*q6)*sin(q2)*sin(q3)*sin(q4)*sin(q5))/8 + (5*3^(1/2)*dq1*dqr4*cos(2*q5)*cos(2*q6)*sin(q2)*sin(q3)*sin(q4))/64 + (3^(1/2)*dq1*dqr4*cos(2*q5)*sin(2*q6)*cos(q4)*sin(q2)*sin(q3))/8 + (5*3^(1/2)*dq1*dqr4*cos(2*q6)*sin(2*q5)*cos(q4)*sin(q2)*sin(q3))/32 - (3^(1/2)*dq1*dqr4*sin(2*q5)*sin(2*q6)*sin(q2)*sin(q3)*sin(q4))/16;
Y3_20_5=(3*dq3*dqr4*sin(2*q4))/128 - (3*dq2*dqr4*sin(2*q4))/128 - (3*dq2*dqr4*cos(2*q4)*sin(q5))/16 - (3*dq2*dqr4*sin(2*q4)*cos(q5))/32 + (3*dq3*dqr4*cos(2*q4)*sin(q5))/16 + (3*dq3*dqr4*sin(2*q4)*cos(q5))/32 - (3^(1/2)*dq4*dqr4*sin(q4))/64 + (5*3^(1/2)*dq5*dqr4*sin(q4))/32 + (3^(1/2)*dq6*dqr4*sin(q4))/8 + (3*dq2*dqr4*cos(2*q4)*sin(2*q5))/32 + (15*dq2*dqr4*cos(2*q5)*sin(2*q4))/128 - (27*dq2*dqr4*cos(2*q6)*sin(2*q4))/128 - (3*dq3*dqr4*cos(2*q4)*sin(2*q5))/32 - (15*dq3*dqr4*cos(2*q5)*sin(2*q4))/128 + (27*dq3*dqr4*cos(2*q6)*sin(2*q4))/128 + (43*dq1*dqr4*cos(q2)*sin(q3))/128 + (3*dq1*dqr4*cos(2*q6)*cos(q2)*sin(q3))/128 - (3^(1/2)*dq4*dqr4*cos(q4)*sin(q5))/16 + (3^(1/2)*dq4*dqr4*cos(q5)*sin(q4))/16 - (3^(1/2)*dq5*dqr4*cos(q4)*sin(q5))/32 - (3^(1/2)*dq5*dqr4*cos(q5)*sin(q4))/16 - (3^(1/2)*dq6*dqr4*cos(q4)*sin(q5))/4 - (3^(1/2)*dq6*dqr4*cos(q5)*sin(q4))/8 - (3*dq2*dqr4*cos(2*q4)*cos(2*q6)*sin(q5))/16 - (3*dq2*dqr4*cos(2*q4)*sin(2*q6)*cos(q5))/8 - (3*dq2*dqr4*cos(2*q6)*sin(2*q4)*cos(q5))/32 + (3*dq3*dqr4*cos(2*q4)*cos(2*q6)*sin(q5))/16 + (3*dq3*dqr4*cos(2*q4)*sin(2*q6)*cos(q5))/8 + (3*dq3*dqr4*cos(2*q6)*sin(2*q4)*cos(q5))/32 + (3*dq2*dqr4*sin(2*q4)*sin(2*q6)*sin(q5))/16 - (3*dq3*dqr4*sin(2*q4)*sin(2*q6)*sin(q5))/16 - (3*3^(1/2)*dq4*dqr4*cos(2*q5)*sin(q4))/64 - (3*3^(1/2)*dq4*dqr4*sin(2*q5)*cos(q4))/32 - (9*3^(1/2)*dq4*dqr4*cos(2*q6)*sin(q4))/64 - (3*3^(1/2)*dq5*dqr4*cos(2*q5)*sin(q4))/32 - (3*3^(1/2)*dq5*dqr4*sin(2*q5)*cos(q4))/64 - (3*3^(1/2)*dq5*dqr4*cos(2*q6)*sin(q4))/32 - (9*3^(1/2)*dq6*dqr4*sin(2*q6)*cos(q4))/64 - (dq2*dqr4*cos(2*q4)*cos(2*q5)*sin(2*q6))/8 - (5*dq2*dqr4*cos(2*q4)*cos(2*q6)*sin(2*q5))/32 - (25*dq2*dqr4*cos(2*q5)*cos(2*q6)*sin(2*q4))/128 + (dq3*dqr4*cos(2*q4)*cos(2*q5)*sin(2*q6))/8 + (5*dq3*dqr4*cos(2*q4)*cos(2*q6)*sin(2*q5))/32 + (25*dq3*dqr4*cos(2*q5)*cos(2*q6)*sin(2*q4))/128 + (5*dq2*dqr4*sin(2*q4)*sin(2*q5)*sin(2*q6))/32 - (5*dq3*dqr4*sin(2*q4)*sin(2*q5)*sin(2*q6))/32 - (3*dq1*dqr5*sin(2*q4)*cos(q3)*sin(q2)*sin(q5))/64 - (3^(1/2)*dq1*dqr4*cos(q2)*cos(q3)*sin(q4))/64 + (5*3^(1/2)*dq1*dqr5*sin(q2)*sin(q3)*sin(q4))/32 - (3^(1/2)*dq4*dqr4*cos(2*q6)*cos(q4)*sin(q5))/16 + (3^(1/2)*dq4*dqr4*cos(2*q6)*cos(q5)*sin(q4))/16 - (3^(1/2)*dq4*dqr4*sin(2*q6)*cos(q4)*cos(q5))/8 - (3^(1/2)*dq5*dqr4*cos(2*q6)*cos(q4)*sin(q5))/32 - (3^(1/2)*dq5*dqr4*cos(2*q6)*cos(q5)*sin(q4))/16 - (3^(1/2)*dq5*dqr4*sin(2*q6)*cos(q4)*cos(q5))/16 + (3^(1/2)*dq6*dqr4*cos(2*q6)*cos(q4)*sin(q5))/8 - (3^(1/2)*dq6*dqr4*cos(2*q6)*cos(q5)*sin(q4))/8 + (3^(1/2)*dq6*dqr4*sin(2*q6)*cos(q4)*cos(q5))/16 - (3^(1/2)*dq4*dqr4*sin(2*q6)*sin(q4)*sin(q5))/8 + (3^(1/2)*dq5*dqr4*sin(2*q6)*sin(q4)*sin(q5))/8 + (3^(1/2)*dq6*dqr4*sin(2*q6)*sin(q4)*sin(q5))/16 + (5*3^(1/2)*dq4*dqr4*cos(2*q5)*cos(2*q6)*sin(q4))/64 + (3^(1/2)*dq4*dqr4*cos(2*q5)*sin(2*q6)*cos(q4))/8 + (5*3^(1/2)*dq4*dqr4*cos(2*q6)*sin(2*q5)*cos(q4))/32 + (5*3^(1/2)*dq5*dqr4*cos(2*q5)*cos(2*q6)*sin(q4))/32 + (3^(1/2)*dq5*dqr4*cos(2*q5)*sin(2*q6)*cos(q4))/16 + (5*3^(1/2)*dq5*dqr4*cos(2*q6)*sin(2*q5)*cos(q4))/64 + (3^(1/2)*dq6*dqr4*cos(2*q5)*cos(2*q6)*sin(q4))/8 + (5*3^(1/2)*dq6*dqr4*cos(2*q5)*sin(2*q6)*cos(q4))/64 + (3^(1/2)*dq6*dqr4*cos(2*q6)*sin(2*q5)*cos(q4))/16 - (3^(1/2)*dq4*dqr4*sin(2*q5)*sin(2*q6)*sin(q4))/16 - (3^(1/2)*dq5*dqr4*sin(2*q5)*sin(2*q6)*sin(q4))/8 - (5*3^(1/2)*dq6*dqr4*sin(2*q5)*sin(2*q6)*sin(q4))/32 - (3^(1/2)*dq1*dqr5*cos(q4)*sin(q2)*sin(q3)*sin(q5))/32 - (3^(1/2)*dq1*dqr5*cos(q5)*sin(q2)*sin(q3)*sin(q4))/16 - (3*dq1*dqr5*cos(2*q6)*sin(2*q4)*cos(q3)*sin(q2)*sin(q5))/64 - (3*3^(1/2)*dq1*dqr4*cos(2*q5)*cos(q2)*cos(q3)*sin(q4))/64 - (3*3^(1/2)*dq1*dqr4*sin(2*q5)*cos(q2)*cos(q3)*cos(q4))/32 - (9*3^(1/2)*dq1*dqr4*cos(2*q6)*cos(q2)*cos(q3)*sin(q4))/64 - (3*3^(1/2)*dq1*dqr5*cos(2*q5)*sin(q2)*sin(q3)*sin(q4))/32 - (3*3^(1/2)*dq1*dqr5*sin(2*q5)*cos(q4)*sin(q2)*sin(q3))/64 - (3*3^(1/2)*dq1*dqr5*cos(2*q6)*sin(q2)*sin(q3)*sin(q4))/32 - (3^(1/2)*dq1*dqr4*cos(q2)*cos(q3)*cos(q4)*sin(q5))/16 + (3^(1/2)*dq1*dqr4*cos(q2)*cos(q3)*cos(q5)*sin(q4))/16 - (3^(1/2)*dq1*dqr4*cos(2*q6)*cos(q2)*cos(q3)*cos(q4)*sin(q5))/16 + (3^(1/2)*dq1*dqr4*cos(2*q6)*cos(q2)*cos(q3)*cos(q5)*sin(q4))/16 - (3^(1/2)*dq1*dqr4*sin(2*q6)*cos(q2)*cos(q3)*cos(q4)*cos(q5))/8 - (3^(1/2)*dq1*dqr4*sin(2*q6)*cos(q2)*cos(q3)*sin(q4)*sin(q5))/8 - (3^(1/2)*dq1*dqr5*cos(2*q6)*cos(q4)*sin(q2)*sin(q3)*sin(q5))/32 - (3^(1/2)*dq1*dqr5*cos(2*q6)*cos(q5)*sin(q2)*sin(q3)*sin(q4))/16 - (3^(1/2)*dq1*dqr5*sin(2*q6)*cos(q4)*cos(q5)*sin(q2)*sin(q3))/16 + (3^(1/2)*dq1*dqr5*sin(2*q6)*sin(q2)*sin(q3)*sin(q4)*sin(q5))/8 + (5*3^(1/2)*dq1*dqr4*cos(2*q5)*cos(2*q6)*cos(q2)*cos(q3)*sin(q4))/64 + (3^(1/2)*dq1*dqr4*cos(2*q5)*sin(2*q6)*cos(q2)*cos(q3)*cos(q4))/8 + (5*3^(1/2)*dq1*dqr4*cos(2*q6)*sin(2*q5)*cos(q2)*cos(q3)*cos(q4))/32 - (3^(1/2)*dq1*dqr4*sin(2*q5)*sin(2*q6)*cos(q2)*cos(q3)*sin(q4))/16 + (5*3^(1/2)*dq1*dqr5*cos(2*q5)*cos(2*q6)*sin(q2)*sin(q3)*sin(q4))/32 + (3^(1/2)*dq1*dqr5*cos(2*q5)*sin(2*q6)*cos(q4)*sin(q2)*sin(q3))/16 + (5*3^(1/2)*dq1*dqr5*cos(2*q6)*sin(2*q5)*cos(q4)*sin(q2)*sin(q3))/64 - (3^(1/2)*dq1*dqr5*sin(2*q5)*sin(2*q6)*sin(q2)*sin(q3)*sin(q4))/8;
Y3_20_6=(3*dq3*dqr5*sin(q5))/64 - (3*dq2*dqr5*sin(q5))/64 - (9*dq2*dqr5*sin(2*q5))/128 - (3*dq2*dqr5*cos(2*q4)*sin(q5))/64 - (3*dq2*dqr5*sin(2*q4)*cos(q5))/32 + (3*dq3*dqr5*cos(2*q4)*sin(q5))/64 + (3*dq3*dqr5*sin(2*q4)*cos(q5))/32 - (3*dq2*dqr5*cos(2*q6)*sin(q5))/64 - (3*dq2*dqr5*sin(2*q6)*cos(q5))/32 + (3*dq3*dqr5*cos(2*q6)*sin(q5))/64 + (3*dq3*dqr5*sin(2*q6)*cos(q5))/32 + (5*3^(1/2)*dq4*dqr5*sin(q4))/32 + (15*dq2*dqr5*cos(2*q4)*sin(2*q5))/128 + (3*dq2*dqr5*cos(2*q5)*sin(2*q4))/32 + (3*dq2*dqr5*cos(2*q5)*sin(2*q6))/32 + (15*dq2*dqr5*cos(2*q6)*sin(2*q5))/128 + (5*dq1*dqr5*cos(q2)*sin(q3))/32 - (5*dq1*dqr5*cos(q3)*sin(q2))/32 - (3*dq1*dqr5*cos(2*q6)*cos(q2)*sin(q3))/32 + (3*dq1*dqr5*cos(2*q6)*cos(q3)*sin(q2))/32 - (3^(1/2)*dq4*dqr5*cos(q4)*sin(q5))/32 - (3^(1/2)*dq4*dqr5*cos(q5)*sin(q4))/16 - (3^(1/2)*dq5*dqr5*cos(q4)*sin(q5))/16 - (3^(1/2)*dq5*dqr5*cos(q5)*sin(q4))/8 - (3^(1/2)*dq6*dqr5*cos(q4)*sin(q5))/8 - (3^(1/2)*dq6*dqr5*cos(q5)*sin(q4))/4 - (3*dq2*dqr5*cos(2*q4)*cos(2*q6)*sin(q5))/64 - (3*dq2*dqr5*cos(2*q4)*sin(2*q6)*cos(q5))/32 - (3*dq2*dqr5*cos(2*q6)*sin(2*q4)*cos(q5))/32 + (3*dq3*dqr5*cos(2*q4)*cos(2*q6)*sin(q5))/64 + (3*dq3*dqr5*cos(2*q4)*sin(2*q6)*cos(q5))/32 + (3*dq3*dqr5*cos(2*q6)*sin(2*q4)*cos(q5))/32 + (3*dq2*dqr5*sin(2*q4)*sin(2*q6)*sin(q5))/16 - (3*dq3*dqr5*sin(2*q4)*sin(2*q6)*sin(q5))/16 - (3*3^(1/2)*dq4*dqr5*cos(2*q5)*sin(q4))/32 - (3*3^(1/2)*dq4*dqr5*sin(2*q5)*cos(q4))/64 - (3*3^(1/2)*dq4*dqr5*cos(2*q6)*sin(q4))/32 - (3*3^(1/2)*dq6*dqr5*sin(2*q6)*cos(q4))/16 + (3*dq1*dqr5*cos(q2)*cos(q5)*sin(q3))/32 - (3*dq1*dqr5*cos(q3)*cos(q5)*sin(q2))/32 - (5*dq2*dqr5*cos(2*q4)*cos(2*q5)*sin(2*q6))/32 - (25*dq2*dqr5*cos(2*q4)*cos(2*q6)*sin(2*q5))/128 - (5*dq2*dqr5*cos(2*q5)*cos(2*q6)*sin(2*q4))/32 + (dq2*dqr5*sin(2*q4)*sin(2*q5)*sin(2*q6))/8 + (3*dq1*dqr5*sin(2*q4)*cos(q2)*sin(q3)*sin(q5))/64 - (3*dq1*dqr5*sin(2*q6)*cos(q2)*sin(q3)*sin(q5))/16 + (3*dq1*dqr5*sin(2*q6)*cos(q3)*sin(q2)*sin(q5))/16 + (5*3^(1/2)*dq1*dqr5*cos(q2)*cos(q3)*sin(q4))/32 + (3*dq1*dqr5*cos(2*q4)*cos(2*q5)*cos(q2)*sin(q3))/32 - (3*dq1*dqr5*cos(2*q4)*cos(2*q5)*cos(q3)*sin(q2))/32 - (15*dq1*dqr5*sin(2*q4)*sin(2*q5)*cos(q2)*sin(q3))/128 + (15*dq1*dqr5*sin(2*q4)*sin(2*q5)*cos(q3)*sin(q2))/128 - (3^(1/2)*dq4*dqr5*cos(2*q6)*cos(q4)*sin(q5))/32 - (3^(1/2)*dq4*dqr5*cos(2*q6)*cos(q5)*sin(q4))/16 - (3^(1/2)*dq4*dqr5*sin(2*q6)*cos(q4)*cos(q5))/16 - (3^(1/2)*dq5*dqr5*cos(2*q6)*cos(q4)*sin(q5))/16 - (3^(1/2)*dq5*dqr5*cos(2*q6)*cos(q5)*sin(q4))/8 - (3^(1/2)*dq5*dqr5*sin(2*q6)*cos(q4)*cos(q5))/8 - (3^(1/2)*dq6*dqr5*cos(2*q6)*cos(q4)*sin(q5))/8 - (3^(1/2)*dq6*dqr5*cos(2*q6)*cos(q5)*sin(q4))/4 - (3^(1/2)*dq6*dqr5*sin(2*q6)*cos(q4)*cos(q5))/16 + (3^(1/2)*dq4*dqr5*sin(2*q6)*sin(q4)*sin(q5))/8 + (3^(1/2)*dq5*dqr5*sin(2*q6)*sin(q4)*sin(q5))/4 + (3^(1/2)*dq6*dqr5*sin(2*q6)*sin(q4)*sin(q5))/8 + (5*3^(1/2)*dq4*dqr5*cos(2*q5)*cos(2*q6)*sin(q4))/32 + (3^(1/2)*dq4*dqr5*cos(2*q5)*sin(2*q6)*cos(q4))/16 + (5*3^(1/2)*dq4*dqr5*cos(2*q6)*sin(2*q5)*cos(q4))/64 - (3*dq1*dqr5*cos(2*q4)*cos(q2)*cos(q5)*sin(q3))/32 + (3*dq1*dqr5*cos(2*q4)*cos(q3)*cos(q5)*sin(q2))/32 + (3*dq1*dqr5*cos(2*q6)*cos(q2)*cos(q5)*sin(q3))/32 - (3*dq1*dqr5*cos(2*q6)*cos(q3)*cos(q5)*sin(q2))/32 - (3^(1/2)*dq4*dqr5*sin(2*q5)*sin(2*q6)*sin(q4))/8 - (3*dq1*dqr5*cos(2*q4)*cos(2*q6)*cos(q2)*cos(q5)*sin(q3))/32 + (3*dq1*dqr5*cos(2*q4)*cos(2*q6)*cos(q3)*cos(q5)*sin(q2))/32 + (3*dq1*dqr5*cos(2*q4)*sin(2*q6)*cos(q2)*sin(q3)*sin(q5))/16 - (3*dq1*dqr5*cos(2*q4)*sin(2*q6)*cos(q3)*sin(q2)*sin(q5))/16 + (3*dq1*dqr5*cos(2*q6)*sin(2*q4)*cos(q2)*sin(q3)*sin(q5))/64 + (3*dq1*dqr5*sin(2*q4)*sin(2*q6)*cos(q2)*cos(q5)*sin(q3))/32 - (3*dq1*dqr5*sin(2*q4)*sin(2*q6)*cos(q3)*cos(q5)*sin(q2))/32 - (3*3^(1/2)*dq1*dqr5*cos(2*q5)*cos(q2)*cos(q3)*sin(q4))/32 - (3*3^(1/2)*dq1*dqr5*sin(2*q5)*cos(q2)*cos(q3)*cos(q4))/64 - (3*3^(1/2)*dq1*dqr5*cos(2*q6)*cos(q2)*cos(q3)*sin(q4))/32 - (5*dq1*dqr5*cos(2*q4)*cos(2*q5)*cos(2*q6)*cos(q2)*sin(q3))/32 + (5*dq1*dqr5*cos(2*q4)*cos(2*q5)*cos(2*q6)*cos(q3)*sin(q2))/32 + (dq1*dqr5*cos(2*q4)*sin(2*q5)*sin(2*q6)*cos(q2)*sin(q3))/8 - (dq1*dqr5*cos(2*q4)*sin(2*q5)*sin(2*q6)*cos(q3)*sin(q2))/8 + (5*dq1*dqr5*cos(2*q5)*sin(2*q4)*sin(2*q6)*cos(q2)*sin(q3))/32 - (5*dq1*dqr5*cos(2*q5)*sin(2*q4)*sin(2*q6)*cos(q3)*sin(q2))/32 + (25*dq1*dqr5*cos(2*q6)*sin(2*q4)*sin(2*q5)*cos(q2)*sin(q3))/128 - (25*dq1*dqr5*cos(2*q6)*sin(2*q4)*sin(2*q5)*cos(q3)*sin(q2))/128 - (3^(1/2)*dq1*dqr5*cos(q2)*cos(q3)*cos(q4)*sin(q5))/32 - (3^(1/2)*dq1*dqr5*cos(q2)*cos(q3)*cos(q5)*sin(q4))/16 - (3^(1/2)*dq1*dqr5*cos(2*q6)*cos(q2)*cos(q3)*cos(q4)*sin(q5))/32 - (3^(1/2)*dq1*dqr5*cos(2*q6)*cos(q2)*cos(q3)*cos(q5)*sin(q4))/16 - (3^(1/2)*dq1*dqr5*sin(2*q6)*cos(q2)*cos(q3)*cos(q4)*cos(q5))/16 + (3^(1/2)*dq1*dqr5*sin(2*q6)*cos(q2)*cos(q3)*sin(q4)*sin(q5))/8 + (5*3^(1/2)*dq1*dqr5*cos(2*q5)*cos(2*q6)*cos(q2)*cos(q3)*sin(q4))/32 + (3^(1/2)*dq1*dqr5*cos(2*q5)*sin(2*q6)*cos(q2)*cos(q3)*cos(q4))/16 + (5*3^(1/2)*dq1*dqr5*cos(2*q6)*sin(2*q5)*cos(q2)*cos(q3)*cos(q4))/64 - (3^(1/2)*dq1*dqr5*sin(2*q5)*sin(2*q6)*cos(q2)*cos(q3)*sin(q4))/8;
Y3_20_7=(9*dq3*dqr5*sin(2*q5))/128 - (3*dq2*dqr6*sin(2*q6))/128 - (3*dq2*dqr6*cos(2*q6)*sin(q5))/16 - (3*dq2*dqr6*sin(2*q6)*cos(q5))/32 + (3*dq3*dqr6*cos(2*q6)*sin(q5))/16 + (3*dq3*dqr6*sin(2*q6)*cos(q5))/32 + (3^(1/2)*dq4*dqr6*sin(q4))/8 - (15*dq3*dqr5*cos(2*q4)*sin(2*q5))/128 - (3*dq3*dqr5*cos(2*q5)*sin(2*q4))/32 - (27*dq2*dqr6*cos(2*q4)*sin(2*q6))/128 + (15*dq2*dqr6*cos(2*q5)*sin(2*q6))/128 + (3*dq2*dqr6*cos(2*q6)*sin(2*q5))/32 - (3*dq3*dqr5*cos(2*q5)*sin(2*q6))/32 - (15*dq3*dqr5*cos(2*q6)*sin(2*q5))/128 + (27*dq3*dqr6*cos(2*q4)*sin(2*q6))/128 - (3*dq3*dqr6*cos(2*q6)*sin(2*q5))/32 + (dq1*dqr6*cos(q2)*sin(q3))/8 - (dq1*dqr6*cos(q3)*sin(q2))/8 - (3^(1/2)*dq4*dqr6*cos(q4)*sin(q5))/4 - (3^(1/2)*dq4*dqr6*cos(q5)*sin(q4))/8 - (3^(1/2)*dq5*dqr6*cos(q4)*sin(q5))/8 - (3^(1/2)*dq5*dqr6*cos(q5)*sin(q4))/4 - (3*dq2*dqr6*cos(2*q4)*cos(2*q6)*sin(q5))/16 - (3*dq2*dqr6*cos(2*q4)*sin(2*q6)*cos(q5))/32 - (3*dq2*dqr6*cos(2*q6)*sin(2*q4)*cos(q5))/8 + (3*dq3*dqr6*cos(2*q4)*cos(2*q6)*sin(q5))/16 + (3*dq3*dqr6*cos(2*q4)*sin(2*q6)*cos(q5))/32 + (3*dq3*dqr6*cos(2*q6)*sin(2*q4)*cos(q5))/8 + (3*dq2*dqr6*sin(2*q4)*sin(2*q6)*sin(q5))/16 - (3*dq3*dqr6*sin(2*q4)*sin(2*q6)*sin(q5))/16 - (9*3^(1/2)*dq4*dqr6*sin(2*q6)*cos(q4))/64 - (3*3^(1/2)*dq5*dqr6*sin(2*q6)*cos(q4))/16 + (3*dq1*dqr6*cos(q2)*cos(q5)*sin(q3))/8 - (3*dq1*dqr6*cos(q3)*cos(q5)*sin(q2))/8 - (25*dq2*dqr6*cos(2*q4)*cos(2*q5)*sin(2*q6))/128 - (5*dq2*dqr6*cos(2*q4)*cos(2*q6)*sin(2*q5))/32 - (dq2*dqr6*cos(2*q5)*cos(2*q6)*sin(2*q4))/8 + (5*dq3*dqr5*cos(2*q4)*cos(2*q5)*sin(2*q6))/32 + (25*dq3*dqr5*cos(2*q4)*cos(2*q6)*sin(2*q5))/128 + (5*dq3*dqr5*cos(2*q5)*cos(2*q6)*sin(2*q4))/32 + (25*dq3*dqr6*cos(2*q4)*cos(2*q5)*sin(2*q6))/128 + (5*dq3*dqr6*cos(2*q4)*cos(2*q6)*sin(2*q5))/32 + (dq3*dqr6*cos(2*q5)*cos(2*q6)*sin(2*q4))/8 + (5*dq2*dqr6*sin(2*q4)*sin(2*q5)*sin(2*q6))/32 - (dq3*dqr5*sin(2*q4)*sin(2*q5)*sin(2*q6))/8 - (5*dq3*dqr6*sin(2*q4)*sin(2*q5)*sin(2*q6))/32 + (3^(1/2)*dq1*dqr6*cos(q2)*cos(q3)*sin(q4))/8 + (3^(1/2)*dq1*dqr6*sin(q2)*sin(q3)*sin(q4))/8 + (27*dq1*dqr6*sin(2*q4)*sin(2*q6)*cos(q2)*sin(q3))/128 - (27*dq1*dqr6*sin(2*q4)*sin(2*q6)*cos(q3)*sin(q2))/128 + (3^(1/2)*dq4*dqr6*cos(2*q6)*cos(q4)*sin(q5))/8 - (3^(1/2)*dq4*dqr6*cos(2*q6)*cos(q5)*sin(q4))/8 + (3^(1/2)*dq4*dqr6*sin(2*q6)*cos(q4)*cos(q5))/16 - (3^(1/2)*dq5*dqr6*cos(2*q6)*cos(q4)*sin(q5))/8 - (3^(1/2)*dq5*dqr6*cos(2*q6)*cos(q5)*sin(q4))/4 - (3^(1/2)*dq5*dqr6*sin(2*q6)*cos(q4)*cos(q5))/16 + (3^(1/2)*dq4*dqr6*sin(2*q6)*sin(q4)*sin(q5))/16 + (3^(1/2)*dq5*dqr6*sin(2*q6)*sin(q4)*sin(q5))/8 + (3^(1/2)*dq4*dqr6*cos(2*q5)*cos(2*q6)*sin(q4))/8 + (5*3^(1/2)*dq4*dqr6*cos(2*q5)*sin(2*q6)*cos(q4))/64 + (3^(1/2)*dq4*dqr6*cos(2*q6)*sin(2*q5)*cos(q4))/16 - (5*3^(1/2)*dq4*dqr6*sin(2*q5)*sin(2*q6)*sin(q4))/32 - (3^(1/2)*dq1*dqr6*cos(q4)*sin(q2)*sin(q3)*sin(q5))/4 - (3^(1/2)*dq1*dqr6*cos(q5)*sin(q2)*sin(q3)*sin(q4))/8 - (3*dq1*dqr6*cos(2*q4)*cos(2*q6)*cos(q2)*cos(q5)*sin(q3))/8 + (3*dq1*dqr6*cos(2*q4)*cos(2*q6)*cos(q3)*cos(q5)*sin(q2))/8 + (3*dq1*dqr6*cos(2*q4)*sin(2*q6)*cos(q2)*sin(q3)*sin(q5))/16 - (3*dq1*dqr6*cos(2*q4)*sin(2*q6)*cos(q3)*sin(q2)*sin(q5))/16 + (3*dq1*dqr6*cos(2*q6)*sin(2*q4)*cos(q2)*sin(q3)*sin(q5))/16 - (3*dq1*dqr6*cos(2*q6)*sin(2*q4)*cos(q3)*sin(q2)*sin(q5))/16 + (3*dq1*dqr6*sin(2*q4)*sin(2*q6)*cos(q2)*cos(q5)*sin(q3))/32 - (3*dq1*dqr6*sin(2*q4)*sin(2*q6)*cos(q3)*cos(q5)*sin(q2))/32 - (9*3^(1/2)*dq1*dqr6*sin(2*q6)*cos(q2)*cos(q3)*cos(q4))/64 - (9*3^(1/2)*dq1*dqr6*sin(2*q6)*cos(q4)*sin(q2)*sin(q3))/64 - (dq1*dqr6*cos(2*q4)*cos(2*q5)*cos(2*q6)*cos(q2)*sin(q3))/8 + (dq1*dqr6*cos(2*q4)*cos(2*q5)*cos(2*q6)*cos(q3)*sin(q2))/8 + (5*dq1*dqr6*cos(2*q4)*sin(2*q5)*sin(2*q6)*cos(q2)*sin(q3))/32 - (5*dq1*dqr6*cos(2*q4)*sin(2*q5)*sin(2*q6)*cos(q3)*sin(q2))/32 + (25*dq1*dqr6*cos(2*q5)*sin(2*q4)*sin(2*q6)*cos(q2)*sin(q3))/128 - (25*dq1*dqr6*cos(2*q5)*sin(2*q4)*sin(2*q6)*cos(q3)*sin(q2))/128 + (5*dq1*dqr6*cos(2*q6)*sin(2*q4)*sin(2*q5)*cos(q2)*sin(q3))/32 - (5*dq1*dqr6*cos(2*q6)*sin(2*q4)*sin(2*q5)*cos(q3)*sin(q2))/32 - (3^(1/2)*dq1*dqr6*cos(q2)*cos(q3)*cos(q4)*sin(q5))/4 - (3^(1/2)*dq1*dqr6*cos(q2)*cos(q3)*cos(q5)*sin(q4))/8 + (3^(1/2)*dq1*dqr6*cos(2*q6)*cos(q2)*cos(q3)*cos(q4)*sin(q5))/8 - (3^(1/2)*dq1*dqr6*cos(2*q6)*cos(q2)*cos(q3)*cos(q5)*sin(q4))/8 + (3^(1/2)*dq1*dqr6*sin(2*q6)*cos(q2)*cos(q3)*cos(q4)*cos(q5))/16 + (3^(1/2)*dq1*dqr6*cos(2*q6)*cos(q4)*sin(q2)*sin(q3)*sin(q5))/8 - (3^(1/2)*dq1*dqr6*cos(2*q6)*cos(q5)*sin(q2)*sin(q3)*sin(q4))/8 + (3^(1/2)*dq1*dqr6*sin(2*q6)*cos(q2)*cos(q3)*sin(q4)*sin(q5))/16 + (3^(1/2)*dq1*dqr6*sin(2*q6)*cos(q4)*cos(q5)*sin(q2)*sin(q3))/16 + (3^(1/2)*dq1*dqr6*sin(2*q6)*sin(q2)*sin(q3)*sin(q4)*sin(q5))/16 + (3^(1/2)*dq1*dqr6*cos(2*q5)*cos(2*q6)*cos(q2)*cos(q3)*sin(q4))/8 + (5*3^(1/2)*dq1*dqr6*cos(2*q5)*sin(2*q6)*cos(q2)*cos(q3)*cos(q4))/64 + (3^(1/2)*dq1*dqr6*cos(2*q6)*sin(2*q5)*cos(q2)*cos(q3)*cos(q4))/16 + (3^(1/2)*dq1*dqr6*cos(2*q5)*cos(2*q6)*sin(q2)*sin(q3)*sin(q4))/8 + (5*3^(1/2)*dq1*dqr6*cos(2*q5)*sin(2*q6)*cos(q4)*sin(q2)*sin(q3))/64 + (3^(1/2)*dq1*dqr6*cos(2*q6)*sin(2*q5)*cos(q4)*sin(q2)*sin(q3))/16 - (5*3^(1/2)*dq1*dqr6*sin(2*q5)*sin(2*q6)*cos(q2)*cos(q3)*sin(q4))/32 - (5*3^(1/2)*dq1*dqr6*sin(2*q5)*sin(2*q6)*sin(q2)*sin(q3)*sin(q4))/32;
Y3_20_8=(ddqr2*cos(q4)^2*cos(q6)^2)/16 - (5*ddqr2*cos(q4)^2*cos(q5)^2)/4 + (3*dq3*dqr6*sin(2*q6))/128 + (3*ddqr2*cos(q4)^2*cos(q5)*cos(q6)^2)/8 + (25*ddqr2*cos(q4)^2*cos(q5)^2*cos(q6)^2)/16 - (15*dq3*dqr6*cos(2*q5)*sin(2*q6))/128 - (3^(1/2)*ddqr6*sin(q4)*sin(q5))/2 - (3^(1/2)*ddqr4*cos(q6)^2*sin(q4)*sin(q5))/8 - (3^(1/2)*ddqr5*cos(q6)^2*sin(q4)*sin(q5))/4 - (ddqr1*cos(q2)*cos(q4)*sin(q3)*sin(q4))/4 + (ddqr1*cos(q3)*cos(q4)*sin(q2)*sin(q4))/4 - (ddqr1*cos(q2)*cos(q5)*sin(q3)*sin(q5))/2 + (ddqr1*cos(q3)*cos(q5)*sin(q2)*sin(q5))/2 - (ddqr1*cos(q2)*cos(q6)*sin(q3)*sin(q6))/4 + (ddqr1*cos(q3)*cos(q6)*sin(q2)*sin(q6))/4 + ddqr2*cos(q4)*cos(q5)*sin(q4)*sin(q5) - ddqr3*cos(q4)*cos(q5)*sin(q4)*sin(q5) + (ddqr2*cos(q4)*cos(q6)*sin(q4)*sin(q6))/2 - (ddqr3*cos(q4)*cos(q6)*sin(q4)*sin(q6))/2 + ddqr2*cos(q5)*cos(q6)*sin(q5)*sin(q6) - ddqr3*cos(q5)*cos(q6)*sin(q5)*sin(q6) + (3*ddqr1*cos(q2)*cos(q6)^2*sin(q3)*sin(q5))/8 - (3*ddqr1*cos(q3)*cos(q6)^2*sin(q2)*sin(q5))/8 - (3*ddqr2*cos(q4)*cos(q6)^2*sin(q4)*sin(q5))/4 + (3*ddqr3*cos(q4)*cos(q6)^2*sin(q4)*sin(q5))/4 - (3*ddqr2*cos(q4)^2*cos(q6)*sin(q5)*sin(q6))/4 + (3*ddqr3*cos(q4)^2*cos(q6)*sin(q5)*sin(q6))/4 - (3^(1/2)*ddqr1*cos(q2)*cos(q3)*cos(q4))/4 - (3^(1/2)*ddqr1*cos(q4)*sin(q2)*sin(q3))/4 - (3^(1/2)*ddqr4*cos(q5)*sin(q4)*sin(q5))/2 - (3^(1/2)*ddqr4*cos(q6)*sin(q4)*sin(q6))/4 + (3*ddqr1*cos(q2)*cos(q5)*cos(q6)*sin(q3)*sin(q6))/4 - (3*ddqr1*cos(q3)*cos(q5)*cos(q6)*sin(q2)*sin(q6))/4 - (3*ddqr2*cos(q4)*cos(q5)*cos(q6)*sin(q4)*sin(q6))/2 + (3*ddqr3*cos(q4)*cos(q5)*cos(q6)*sin(q4)*sin(q6))/2 + (5*ddqr1*cos(q2)*cos(q4)*cos(q5)^2*sin(q3)*sin(q4))/4 - (5*ddqr1*cos(q3)*cos(q4)*cos(q5)^2*sin(q2)*sin(q4))/4 - (ddqr1*cos(q2)*cos(q4)*cos(q6)^2*sin(q3)*sin(q4))/16 + ddqr1*cos(q2)*cos(q4)^2*cos(q5)*sin(q3)*sin(q5) + (ddqr1*cos(q3)*cos(q4)*cos(q6)^2*sin(q2)*sin(q4))/16 - ddqr1*cos(q3)*cos(q4)^2*cos(q5)*sin(q2)*sin(q5) + (5*ddqr1*cos(q2)*cos(q5)*cos(q6)^2*sin(q3)*sin(q5))/8 + (ddqr1*cos(q2)*cos(q4)^2*cos(q6)*sin(q3)*sin(q6))/2 - (5*ddqr1*cos(q3)*cos(q5)*cos(q6)^2*sin(q2)*sin(q5))/8 - (ddqr1*cos(q3)*cos(q4)^2*cos(q6)*sin(q2)*sin(q6))/2 + (ddqr1*cos(q2)*cos(q5)^2*cos(q6)*sin(q3)*sin(q6))/2 - (ddqr1*cos(q3)*cos(q5)^2*cos(q6)*sin(q2)*sin(q6))/2 - (5*ddqr2*cos(q4)*cos(q5)*cos(q6)^2*sin(q4)*sin(q5))/4 - ddqr2*cos(q4)*cos(q5)^2*cos(q6)*sin(q4)*sin(q6) + (5*ddqr3*cos(q4)*cos(q5)*cos(q6)^2*sin(q4)*sin(q5))/4 - (5*ddqr2*cos(q4)^2*cos(q5)*cos(q6)*sin(q5)*sin(q6))/4 + ddqr3*cos(q4)*cos(q5)^2*cos(q6)*sin(q4)*sin(q6) + (5*ddqr3*cos(q4)^2*cos(q5)*cos(q6)*sin(q5)*sin(q6))/4 + (3^(1/2)*ddqr4*cos(q4)*cos(q6)*sin(q5)*sin(q6))/4 - (3^(1/2)*ddqr4*cos(q5)*cos(q6)*sin(q4)*sin(q6))/4 - (3^(1/2)*ddqr5*cos(q4)*cos(q6)*sin(q5)*sin(q6))/4 - (3^(1/2)*ddqr5*cos(q5)*cos(q6)*sin(q4)*sin(q6))/2 - (3*ddqr1*cos(q2)*cos(q4)^2*cos(q6)^2*sin(q3)*sin(q5))/4 + (3*ddqr1*cos(q3)*cos(q4)^2*cos(q6)^2*sin(q2)*sin(q5))/4 + (3^(1/2)*ddqr1*cos(q2)*cos(q3)*cos(q4)*cos(q5)^2)/4 + (7*3^(1/2)*ddqr1*cos(q2)*cos(q3)*cos(q4)*cos(q6)^2)/16 + (3^(1/2)*ddqr1*cos(q4)*cos(q5)^2*sin(q2)*sin(q3))/4 + (7*3^(1/2)*ddqr1*cos(q4)*cos(q6)^2*sin(q2)*sin(q3))/16 + (5*3^(1/2)*ddqr4*cos(q5)*cos(q6)^2*sin(q4)*sin(q5))/8 + (3^(1/2)*ddqr4*cos(q5)^2*cos(q6)*sin(q4)*sin(q6))/2 - (5*3^(1/2)*ddqr1*cos(q2)*cos(q3)*cos(q4)*cos(q5)^2*cos(q6)^2)/16 - (5*3^(1/2)*ddqr1*cos(q4)*cos(q5)^2*cos(q6)^2*sin(q2)*sin(q3))/16 - (3*ddqr1*cos(q2)*cos(q4)*cos(q5)*cos(q6)^2*sin(q3)*sin(q4))/8 + (3*ddqr1*cos(q3)*cos(q4)*cos(q5)*cos(q6)^2*sin(q2)*sin(q4))/8 - (3*ddqr1*cos(q2)*cos(q4)^2*cos(q5)*cos(q6)*sin(q3)*sin(q6))/2 + (3*ddqr1*cos(q3)*cos(q4)^2*cos(q5)*cos(q6)*sin(q2)*sin(q6))/2 - (3^(1/2)*ddqr1*cos(q2)*cos(q3)*cos(q5)*sin(q4)*sin(q5))/2 - (3^(1/2)*ddqr1*cos(q2)*cos(q3)*cos(q6)*sin(q4)*sin(q6))/4 + (3^(1/2)*ddqr4*cos(q4)*cos(q5)*cos(q6)*sin(q5)*sin(q6))/4 - (3^(1/2)*ddqr1*cos(q5)*sin(q2)*sin(q3)*sin(q4)*sin(q5))/2 - (3^(1/2)*ddqr1*cos(q6)*sin(q2)*sin(q3)*sin(q4)*sin(q6))/4 - (25*ddqr1*cos(q2)*cos(q4)*cos(q5)^2*cos(q6)^2*sin(q3)*sin(q4))/16 + (25*ddqr1*cos(q3)*cos(q4)*cos(q5)^2*cos(q6)^2*sin(q2)*sin(q4))/16 - (5*ddqr1*cos(q2)*cos(q4)^2*cos(q5)*cos(q6)^2*sin(q3)*sin(q5))/4 + (5*ddqr1*cos(q3)*cos(q4)^2*cos(q5)*cos(q6)^2*sin(q2)*sin(q5))/4 - ddqr1*cos(q2)*cos(q4)^2*cos(q5)^2*cos(q6)*sin(q3)*sin(q6) + ddqr1*cos(q3)*cos(q4)^2*cos(q5)^2*cos(q6)*sin(q2)*sin(q6) - (3^(1/2)*ddqr1*cos(q2)*cos(q3)*cos(q4)*cos(q5)*cos(q6)^2)/8 - (3^(1/2)*ddqr1*cos(q2)*cos(q3)*cos(q6)^2*sin(q4)*sin(q5))/8 - (3^(1/2)*ddqr1*cos(q4)*cos(q5)*cos(q6)^2*sin(q2)*sin(q3))/8 - (3^(1/2)*ddqr1*cos(q6)^2*sin(q2)*sin(q3)*sin(q4)*sin(q5))/8 + (3^(1/2)*ddqr1*cos(q2)*cos(q3)*cos(q4)*cos(q6)*sin(q5)*sin(q6))/4 - (3^(1/2)*ddqr1*cos(q2)*cos(q3)*cos(q5)*cos(q6)*sin(q4)*sin(q6))/4 + (3^(1/2)*ddqr1*cos(q4)*cos(q6)*sin(q2)*sin(q3)*sin(q5)*sin(q6))/4 - (3^(1/2)*ddqr1*cos(q5)*cos(q6)*sin(q2)*sin(q3)*sin(q4)*sin(q6))/4 + (5*3^(1/2)*ddqr1*cos(q2)*cos(q3)*cos(q5)*cos(q6)^2*sin(q4)*sin(q5))/8 + (3^(1/2)*ddqr1*cos(q2)*cos(q3)*cos(q5)^2*cos(q6)*sin(q4)*sin(q6))/2 + (5*3^(1/2)*ddqr1*cos(q5)*cos(q6)^2*sin(q2)*sin(q3)*sin(q4)*sin(q5))/8 + (3^(1/2)*ddqr1*cos(q5)^2*cos(q6)*sin(q2)*sin(q3)*sin(q4)*sin(q6))/2 + (3*ddqr1*cos(q2)*cos(q4)*cos(q6)*sin(q3)*sin(q4)*sin(q5)*sin(q6))/4 - (3*ddqr1*cos(q3)*cos(q4)*cos(q6)*sin(q2)*sin(q4)*sin(q5)*sin(q6))/4 + (3^(1/2)*ddqr1*cos(q2)*cos(q3)*cos(q4)*cos(q5)*cos(q6)*sin(q5)*sin(q6))/4 + (3^(1/2)*ddqr1*cos(q4)*cos(q5)*cos(q6)*sin(q2)*sin(q3)*sin(q5)*sin(q6))/4 + (5*ddqr1*cos(q2)*cos(q4)*cos(q5)*cos(q6)*sin(q3)*sin(q4)*sin(q5)*sin(q6))/4 - (5*ddqr1*cos(q3)*cos(q4)*cos(q5)*cos(q6)*sin(q2)*sin(q4)*sin(q5)*sin(q6))/4;
Y3_20_9=ddqr3 - ddqr2 + (ddqr2*cos(q4)^2)/4 + ddqr2*cos(q5)^2 - (ddqr3*cos(q4)^2)/4 + (ddqr2*cos(q6)^2)/4 - ddqr3*cos(q5)^2 - (ddqr3*cos(q6)^2)/4 + (5*ddqr3*cos(q4)^2*cos(q5)^2)/4 - (5*ddqr2*cos(q5)^2*cos(q6)^2)/4 - (ddqr3*cos(q4)^2*cos(q6)^2)/16 + (5*ddqr3*cos(q5)^2*cos(q6)^2)/4 - (3^(1/2)*ddqr4*cos(q4))/4 - (3^(1/2)*ddqr5*cos(q4))/2 - (3^(1/2)*ddqr6*cos(q4))/4 - (3*ddqr3*cos(q4)^2*cos(q5)*cos(q6)^2)/8 + (3^(1/2)*ddqr4*cos(q4)*cos(q5)^2)/4 + (7*3^(1/2)*ddqr4*cos(q4)*cos(q6)^2)/16 + (3*3^(1/2)*ddqr5*cos(q4)*cos(q6)^2)/8 - (25*ddqr3*cos(q4)^2*cos(q5)^2*cos(q6)^2)/16 + (3^(1/2)*ddqr6*cos(q4)*cos(q5))/4 - (3^(1/2)*ddqr4*cos(q4)*cos(q5)*cos(q6)^2)/8 + (3^(1/2)*ddqr5*cos(q4)*cos(q5)*cos(q6)^2)/8 - (5*3^(1/2)*ddqr4*cos(q4)*cos(q5)^2*cos(q6)^2)/16;
Y3_22_1=cos(q3)*sin(q2) - cos(q2)*sin(q3);
Y3_23_1=sin(q2)*sin(q3)*sin(q4) + cos(q2)*cos(q3)*sin(q4);
Y3_24_1=(3^(1/2)*cos(q2)*cos(q5)*sin(q3))/2 - (3^(1/2)*cos(q3)*cos(q5)*sin(q2))/2 - cos(q2)*cos(q3)*cos(q4)*sin(q5) - (cos(q2)*cos(q3)*cos(q5)*sin(q4))/2 - cos(q4)*sin(q2)*sin(q3)*sin(q5) - (cos(q5)*sin(q2)*sin(q3)*sin(q4))/2;
Y3_25_1=(3^(1/2)*cos(q2)*cos(q6)*sin(q3))/4 - (3^(1/2)*cos(q3)*cos(q6)*sin(q2))/4 + (3*cos(q2)*cos(q3)*cos(q6)*sin(q4))/4 + (3*cos(q6)*sin(q2)*sin(q3)*sin(q4))/4 - (3^(1/2)*cos(q2)*cos(q5)*cos(q6)*sin(q3))/4 + (3^(1/2)*cos(q3)*cos(q5)*cos(q6)*sin(q2))/4 + (3^(1/2)*cos(q2)*sin(q3)*sin(q5)*sin(q6))/2 - (3^(1/2)*cos(q3)*sin(q2)*sin(q5)*sin(q6))/2 + cos(q2)*cos(q3)*cos(q4)*cos(q5)*sin(q6) + (cos(q2)*cos(q3)*cos(q4)*cos(q6)*sin(q5))/2 + (cos(q2)*cos(q3)*cos(q5)*cos(q6)*sin(q4))/4 - (cos(q2)*cos(q3)*sin(q4)*sin(q5)*sin(q6))/2 + cos(q4)*cos(q5)*sin(q2)*sin(q3)*sin(q6) + (cos(q4)*cos(q6)*sin(q2)*sin(q3)*sin(q5))/2 + (cos(q5)*cos(q6)*sin(q2)*sin(q3)*sin(q4))/4 - (sin(q2)*sin(q3)*sin(q4)*sin(q5)*sin(q6))/2;
Y4_4_1=(1369*ddqr4)/1000000 - (4329*ddqr2*cos(q4))/625000 + (4329*ddqr3*cos(q4))/625000 - (259*dq1*dqr1*sin(q4))/1000000 - (1369*dq2*dqr2*sin(2*q4))/2000000 + (1369*dq2*dqr3*sin(2*q4))/2000000 + (1369*dq3*dqr2*sin(2*q4))/2000000 - (1369*dq3*dqr3*sin(2*q4))/2000000 + (1369*ddqr1*cos(q2)*cos(q3))/1000000 + (1073*ddqr2*cos(q3)*cos(q4))/100000 + (1369*ddqr1*sin(q2)*sin(q3))/1000000 + (1073*ddqr1*sin(q2)*sin(q4))/100000 - (259*ddqr1*cos(q2)*cos(q3)*cos(q4))/1000000 + (4329*ddqr1*cos(q2)*sin(q3)*sin(q4))/625000 - (4329*ddqr1*cos(q3)*sin(q2)*sin(q4))/625000 - (259*ddqr1*cos(q4)*sin(q2)*sin(q3))/1000000 + (1369*dq1*dqr2*cos(q2)*sin(q3))/1000000 - (1369*dq1*dqr2*cos(q3)*sin(q2))/1000000 + (1369*dq2*dqr1*cos(q2)*sin(q3))/1000000 - (1369*dq2*dqr1*cos(q3)*sin(q2))/1000000 - (1073*dq1*dqr1*cos(q4)*sin(q3))/100000 + (1073*dq1*dqr2*cos(q2)*sin(q4))/100000 - (1369*dq1*dqr3*cos(q2)*sin(q3))/1000000 + (1369*dq1*dqr3*cos(q3)*sin(q2))/1000000 + (1073*dq2*dqr1*cos(q2)*sin(q4))/100000 - (1369*dq3*dqr1*cos(q2)*sin(q3))/1000000 + (1369*dq3*dqr1*cos(q3)*sin(q2))/1000000 - (1073*dq2*dqr2*cos(q4)*sin(q3))/100000 + (1073*dq1*dqr1*cos(q2)^2*cos(q4)*sin(q3))/100000 + (1369*dq1*dqr1*cos(q2)^2*cos(q4)*sin(q4))/1000000 - (1369*dq1*dqr2*cos(q2)*cos(q4)^2*sin(q3))/1000000 + (1369*dq1*dqr2*cos(q3)*cos(q4)^2*sin(q2))/1000000 - (1369*dq2*dqr1*cos(q2)*cos(q4)^2*sin(q3))/1000000 + (1369*dq2*dqr1*cos(q3)*cos(q4)^2*sin(q2))/1000000 + (1369*dq1*dqr1*cos(q3)^2*cos(q4)*sin(q4))/1000000 + (1369*dq1*dqr3*cos(q2)*cos(q4)^2*sin(q3))/1000000 - (1369*dq1*dqr3*cos(q3)*cos(q4)^2*sin(q2))/1000000 + (1369*dq3*dqr1*cos(q2)*cos(q4)^2*sin(q3))/1000000 - (1369*dq3*dqr1*cos(q3)*cos(q4)^2*sin(q2))/1000000 - (4329*dq1*dqr1*cos(q2)*cos(q4)*sin(q2))/625000 + (4329*dq1*dqr1*cos(q3)*cos(q4)*sin(q3))/625000 - (4329*dq1*dqr2*cos(q2)*cos(q3)*sin(q4))/625000 - (4329*dq2*dqr1*cos(q2)*cos(q3)*sin(q4))/625000 + (4329*dq1*dqr3*cos(q2)*cos(q3)*sin(q4))/625000 + (4329*dq3*dqr1*cos(q2)*cos(q3)*sin(q4))/625000 - (4329*dq1*dqr2*sin(q2)*sin(q3)*sin(q4))/625000 - (4329*dq2*dqr1*sin(q2)*sin(q3)*sin(q4))/625000 + (4329*dq1*dqr3*sin(q2)*sin(q3)*sin(q4))/625000 + (4329*dq3*dqr1*sin(q2)*sin(q3)*sin(q4))/625000 - (1369*dq1*dqr1*cos(q2)^2*cos(q3)^2*cos(q4)*sin(q4))/500000 - (1073*dq1*dqr1*cos(q2)*cos(q3)*cos(q4)*sin(q2))/100000 + (4329*dq1*dqr1*cos(q2)*cos(q3)^2*cos(q4)*sin(q2))/312500 - (4329*dq1*dqr1*cos(q2)^2*cos(q3)*cos(q4)*sin(q3))/312500 - (1369*dq1*dqr1*cos(q2)*cos(q3)*cos(q4)*sin(q2)*sin(q3)*sin(q4))/500000;
Y4_5_1=(1369*dq2*dqr1*cos(q2)*cos(q5)^2*sin(q3))/4000000 - (1369*dq2*dqr1*cos(q3)*cos(q5)^2*sin(q2))/4000000 - (1369*dq3*dqr1*cos(q2)*cos(q5)^2*sin(q3))/4000000 + (1369*dq3*dqr1*cos(q3)*cos(q5)^2*sin(q2))/4000000 + dq2*dqr1*cos(q2)*sin(q3)*((23717*3^(1/2))/10000000 + 1780243/400000000) - dq2*dqr1*cos(q3)*sin(q2)*((23717*3^(1/2))/10000000 + 1780243/400000000) - dq3*dqr1*cos(q2)*sin(q3)*((23717*3^(1/2))/10000000 + 1780243/400000000) + dq3*dqr1*cos(q3)*sin(q2)*((23717*3^(1/2))/10000000 + 1780243/400000000) + (1073*dq1*dqr1*cos(q4)*cos(q5)*sin(q3))/200000 - (1073*dq1*dqr1*sin(q3)*sin(q4)*sin(q5))/100000 - dq1*dqr1*cos(q4)*sin(q3)*((18589*3^(1/2))/2000000 + 1073/100000) + (1073*dq1*dqr1*cos(q2)^2*sin(q3)*sin(q4)*sin(q5))/100000 + (1369*3^(1/2)*dq5*dqr1*cos(q2)*cos(q4)*sin(q3))/2000000 - (1369*3^(1/2)*dq5*dqr1*cos(q3)*cos(q4)*sin(q2))/2000000 + dq1*dqr1*cos(q2)^2*cos(q4)*sin(q3)*((18589*3^(1/2))/2000000 + 1073/100000) + (1369*dq1*dqr1*cos(q2)^2*cos(q4)*cos(q5)^2*sin(q4))/800000 - (1369*dq2*dqr1*cos(q2)*cos(q4)^2*cos(q5)^2*sin(q3))/800000 + (1369*dq2*dqr1*cos(q3)*cos(q4)^2*cos(q5)^2*sin(q2))/800000 + (1369*dq3*dqr1*cos(q2)*cos(q4)^2*cos(q5)^2*sin(q3))/800000 - (1369*dq3*dqr1*cos(q3)*cos(q4)^2*cos(q5)^2*sin(q2))/800000 + dq1*dqr1*cos(q2)^2*cos(q4)*sin(q4)*((23717*3^(1/2))/10000000 + 1232643/400000000) - dq2*dqr1*cos(q2)*cos(q4)^2*sin(q3)*((23717*3^(1/2))/10000000 + 1232643/400000000) + dq2*dqr1*cos(q3)*cos(q4)^2*sin(q2)*((23717*3^(1/2))/10000000 + 1232643/400000000) + dq3*dqr1*cos(q2)*cos(q4)^2*sin(q3)*((23717*3^(1/2))/10000000 + 1232643/400000000) - dq3*dqr1*cos(q3)*cos(q4)^2*sin(q2)*((23717*3^(1/2))/10000000 + 1232643/400000000) - (32449*dq1*dqr1*cos(q2)*sin(q2)*sin(q4)*sin(q5))/4000000 + (32449*dq1*dqr1*cos(q3)*sin(q3)*sin(q4)*sin(q5))/4000000 + (32449*dq2*dqr1*cos(q4)*sin(q2)*sin(q3)*sin(q5))/4000000 - (32449*dq3*dqr1*cos(q4)*sin(q2)*sin(q3)*sin(q5))/4000000 + (4107*dq5*dqr1*cos(q5)*sin(q2)*sin(q3)*sin(q5))/4000000 - dq2*dqr1*cos(q2)*cos(q5)*sin(q3)*((23717*3^(1/2))/20000000 + 1369/1000000) + dq2*dqr1*cos(q3)*cos(q5)*sin(q2)*((23717*3^(1/2))/20000000 + 1369/1000000) + dq3*dqr1*cos(q2)*cos(q5)*sin(q3)*((23717*3^(1/2))/20000000 + 1369/1000000) - dq3*dqr1*cos(q3)*cos(q5)*sin(q2)*((23717*3^(1/2))/20000000 + 1369/1000000) - dq1*dqr1*cos(q2)*cos(q4)*sin(q2)*((562157*3^(1/2))/80000000 + 32449/4000000) + dq1*dqr1*cos(q3)*cos(q4)*sin(q3)*((562157*3^(1/2))/80000000 + 32449/4000000) - dq2*dqr1*cos(q2)*cos(q3)*sin(q4)*((562157*3^(1/2))/80000000 + 32449/4000000) + dq3*dqr1*cos(q2)*cos(q3)*sin(q4)*((562157*3^(1/2))/80000000 + 32449/4000000) - (1073*dq1*dqr1*cos(q2)^2*cos(q4)*cos(q5)*sin(q3))/200000 + dq5*dqr1*sin(q2)*sin(q3)*sin(q5)*((23717*3^(1/2))/40000000 + 1369/2000000) - dq2*dqr1*sin(q2)*sin(q3)*sin(q4)*((562157*3^(1/2))/80000000 + 32449/4000000) + dq3*dqr1*sin(q2)*sin(q3)*sin(q4)*((562157*3^(1/2))/80000000 + 32449/4000000) - dq1*dqr1*cos(q2)^2*cos(q4)*cos(q5)*sin(q4)*((23717*3^(1/2))/20000000 + 1369/1000000) + dq2*dqr1*cos(q2)*cos(q4)^2*cos(q5)*sin(q3)*((23717*3^(1/2))/20000000 + 1369/1000000) - dq2*dqr1*cos(q3)*cos(q4)^2*cos(q5)*sin(q2)*((23717*3^(1/2))/20000000 + 1369/1000000) - dq3*dqr1*cos(q2)*cos(q4)^2*cos(q5)*sin(q3)*((23717*3^(1/2))/20000000 + 1369/1000000) + dq3*dqr1*cos(q3)*cos(q4)^2*cos(q5)*sin(q2)*((23717*3^(1/2))/20000000 + 1369/1000000) + dq1*dqr1*cos(q2)*cos(q3)^2*cos(q4)*sin(q2)*((562157*3^(1/2))/40000000 + 32449/2000000) - dq1*dqr1*cos(q2)^2*cos(q3)*cos(q4)*sin(q3)*((562157*3^(1/2))/40000000 + 32449/2000000) + (1369*3^(1/2)*dq1*dqr1*cos(q2)*cos(q4)*cos(q5)^2*sin(q2))/4000000 - (1369*3^(1/2)*dq1*dqr1*cos(q3)*cos(q4)*cos(q5)^2*sin(q3))/4000000 + (1369*3^(1/2)*dq2*dqr1*cos(q2)*cos(q3)*cos(q5)^2*sin(q4))/4000000 - (1369*3^(1/2)*dq3*dqr1*cos(q2)*cos(q3)*cos(q5)^2*sin(q4))/4000000 - (1369*3^(1/2)*dq5*dqr1*cos(q2)*cos(q4)*cos(q5)^2*sin(q3))/2000000 + (1369*3^(1/2)*dq5*dqr1*cos(q3)*cos(q4)*cos(q5)^2*sin(q2))/2000000 + (1073*dq1*dqr1*cos(q2)*cos(q3)*cos(q4)*cos(q5)*sin(q2))/200000 + (1369*3^(1/2)*dq2*dqr1*cos(q5)^2*sin(q2)*sin(q3)*sin(q4))/4000000 - (1369*3^(1/2)*dq3*dqr1*cos(q5)^2*sin(q2)*sin(q3)*sin(q4))/4000000 - dq1*dqr1*cos(q2)^2*cos(q3)^2*cos(q4)*sin(q4)*((23717*3^(1/2))/5000000 + 1232643/200000000) - (1369*dq1*dqr1*cos(q2)^2*cos(q3)^2*cos(q4)*cos(q5)^2*sin(q4))/400000 - (1073*dq1*dqr1*cos(q2)*cos(q3)*sin(q2)*sin(q4)*sin(q5))/100000 - dq1*dqr1*cos(q2)*cos(q3)*cos(q4)*sin(q2)*((18589*3^(1/2))/2000000 + 1073/100000) - dq1*dqr1*cos(q2)*cos(q4)*cos(q5)*sin(q2)*((1369*3^(1/2))/2000000 - 45547/20000000) + dq1*dqr1*cos(q3)*cos(q4)*cos(q5)*sin(q3)*((1369*3^(1/2))/2000000 - 45547/20000000) - dq2*dqr1*cos(q2)*cos(q3)*cos(q5)*sin(q4)*((1369*3^(1/2))/2000000 - 45547/20000000) + dq3*dqr1*cos(q2)*cos(q3)*cos(q5)*sin(q4)*((1369*3^(1/2))/2000000 - 45547/20000000) - dq2*dqr1*cos(q5)*sin(q2)*sin(q3)*sin(q4)*((1369*3^(1/2))/2000000 - 45547/20000000) + dq3*dqr1*cos(q5)*sin(q2)*sin(q3)*sin(q4)*((1369*3^(1/2))/2000000 - 45547/20000000) - dq5*dqr1*cos(q2)*sin(q3)*sin(q4)*sin(q5)*((1369*3^(1/2))/2000000 + 71151/40000000) + dq5*dqr1*cos(q3)*sin(q2)*sin(q4)*sin(q5)*((1369*3^(1/2))/2000000 + 71151/40000000) + (32449*dq1*dqr1*cos(q2)*cos(q3)^2*sin(q2)*sin(q4)*sin(q5))/2000000 - (32449*dq1*dqr1*cos(q2)^2*cos(q3)*sin(q3)*sin(q4)*sin(q5))/2000000 + dq1*dqr1*cos(q2)^2*cos(q3)^2*cos(q4)*cos(q5)*sin(q4)*((23717*3^(1/2))/10000000 + 1369/500000) + (1369*dq1*dqr1*cos(q2)*cos(q3)*cos(q5)*sin(q2)*sin(q3)*sin(q5))/1000000 + (1369*dq2*dqr1*cos(q2)*cos(q4)*cos(q5)*sin(q3)*sin(q4)*sin(q5))/1000000 - (1369*dq2*dqr1*cos(q3)*cos(q4)*cos(q5)*sin(q2)*sin(q4)*sin(q5))/1000000 - (1369*dq3*dqr1*cos(q2)*cos(q4)*cos(q5)*sin(q3)*sin(q4)*sin(q5))/1000000 + (1369*dq3*dqr1*cos(q3)*cos(q4)*cos(q5)*sin(q2)*sin(q4)*sin(q5))/1000000 - (1369*3^(1/2)*dq1*dqr1*cos(q2)*cos(q3)^2*cos(q4)*cos(q5)^2*sin(q2))/2000000 + (1369*3^(1/2)*dq1*dqr1*cos(q2)^2*cos(q3)*cos(q4)*cos(q5)^2*sin(q3))/2000000 - dq1*dqr1*cos(q2)*cos(q3)*sin(q2)*sin(q3)*sin(q5)*((23717*3^(1/2))/10000000 + 1369/500000) - dq2*dqr1*cos(q2)*cos(q4)*sin(q3)*sin(q4)*sin(q5)*((23717*3^(1/2))/10000000 + 1369/500000) + dq2*dqr1*cos(q3)*cos(q4)*sin(q2)*sin(q4)*sin(q5)*((23717*3^(1/2))/10000000 + 1369/500000) + dq3*dqr1*cos(q2)*cos(q4)*sin(q3)*sin(q4)*sin(q5)*((23717*3^(1/2))/10000000 + 1369/500000) - dq3*dqr1*cos(q3)*cos(q4)*sin(q2)*sin(q4)*sin(q5)*((23717*3^(1/2))/10000000 + 1369/500000) + dq1*dqr1*cos(q2)*cos(q3)^2*cos(q4)*cos(q5)*sin(q2)*((1369*3^(1/2))/1000000 - 45547/10000000) - dq1*dqr1*cos(q2)^2*cos(q3)*cos(q4)*cos(q5)*sin(q3)*((1369*3^(1/2))/1000000 - 45547/10000000) - (1369*3^(1/2)*dq1*dqr1*cos(q2)*cos(q5)*sin(q2)*sin(q4)*sin(q5))/2000000 + (1369*3^(1/2)*dq1*dqr1*cos(q3)*cos(q5)*sin(q3)*sin(q4)*sin(q5))/2000000 + (1369*3^(1/2)*dq2*dqr1*cos(q4)*cos(q5)*sin(q2)*sin(q3)*sin(q5))/2000000 - (1369*3^(1/2)*dq3*dqr1*cos(q4)*cos(q5)*sin(q2)*sin(q3)*sin(q5))/2000000 + (1369*3^(1/2)*dq5*dqr1*cos(q2)*cos(q5)*sin(q3)*sin(q4)*sin(q5))/4000000 - (1369*3^(1/2)*dq5*dqr1*cos(q3)*cos(q5)*sin(q2)*sin(q4)*sin(q5))/4000000 + (1369*3^(1/2)*dq1*dqr1*cos(q2)*cos(q3)^2*cos(q5)*sin(q2)*sin(q4)*sin(q5))/1000000 - (1369*3^(1/2)*dq1*dqr1*cos(q2)^2*cos(q3)*cos(q5)*sin(q3)*sin(q4)*sin(q5))/1000000 - dq1*dqr1*cos(q2)*cos(q3)*cos(q4)*sin(q2)*sin(q3)*sin(q4)*((23717*3^(1/2))/5000000 + 1232643/200000000) - (1369*dq1*dqr1*cos(q2)*cos(q3)*cos(q4)*cos(q5)^2*sin(q2)*sin(q3)*sin(q4))/400000 - (1369*dq1*dqr1*cos(q2)*cos(q3)*cos(q4)^2*cos(q5)*sin(q2)*sin(q3)*sin(q5))/500000 + dq1*dqr1*cos(q2)*cos(q3)*cos(q4)^2*sin(q2)*sin(q3)*sin(q5)*((23717*3^(1/2))/5000000 + 1369/250000) + dq1*dqr1*cos(q2)*cos(q3)*cos(q4)*cos(q5)*sin(q2)*sin(q3)*sin(q4)*((23717*3^(1/2))/10000000 + 1369/500000);
Y4_5_2=(1369*dq2*dqr2*sin(2*q5))/4000000 - (1369*dq3*dqr2*sin(2*q5))/4000000 - dq1*dqr1*sin(q4)*((4487*3^(1/2))/20000000 + 259/1000000) - dq2*dqr2*sin(q5)*((23717*3^(1/2))/20000000 + 1369/1000000) + dq3*dqr2*sin(q5)*((23717*3^(1/2))/20000000 + 1369/1000000) + (1369*3^(1/2)*dq5*dqr2*sin(q4))/2000000 - dq2*dqr2*sin(2*q4)*((23717*3^(1/2))/20000000 + 1232643/800000000) + dq3*dqr2*sin(2*q4)*((23717*3^(1/2))/20000000 + 1232643/800000000) + (259*dq1*dqr1*cos(q4)*sin(q5))/1000000 + (259*dq1*dqr1*cos(q5)*sin(q4))/2000000 + dq5*dqr2*cos(q4)*sin(q5)*((1369*3^(1/2))/2000000 + 71151/40000000) + (1369*dq1*dqr2*cos(q2)*cos(q5)^2*sin(q3))/4000000 - (1369*dq1*dqr2*cos(q3)*cos(q5)^2*sin(q2))/4000000 - (1369*dq1*dqr1*cos(q2)^2*cos(q5)*sin(q5))/2000000 - (1369*dq1*dqr3*cos(q2)*cos(q5)^2*sin(q3))/4000000 + (1369*dq1*dqr3*cos(q3)*cos(q5)^2*sin(q2))/4000000 - (1369*dq1*dqr1*cos(q3)^2*cos(q5)*sin(q5))/2000000 - (1369*dq2*dqr2*cos(q4)*cos(q5)^2*sin(q4))/800000 - (1369*dq2*dqr2*cos(q4)^2*cos(q5)*sin(q5))/1000000 + (1369*dq3*dqr2*cos(q4)*cos(q5)^2*sin(q4))/800000 + (1369*dq3*dqr2*cos(q4)^2*cos(q5)*sin(q5))/1000000 + dq1*dqr2*cos(q2)*sin(q3)*((23717*3^(1/2))/10000000 + 1780243/400000000) - dq1*dqr2*cos(q3)*sin(q2)*((23717*3^(1/2))/10000000 + 1780243/400000000) - dq1*dqr3*cos(q2)*sin(q3)*((23717*3^(1/2))/10000000 + 1780243/400000000) + dq1*dqr3*cos(q3)*sin(q2)*((23717*3^(1/2))/10000000 + 1780243/400000000) + dq2*dqr2*cos(q4)^2*sin(q5)*((23717*3^(1/2))/10000000 + 1369/500000) - dq3*dqr2*cos(q4)^2*sin(q5)*((23717*3^(1/2))/10000000 + 1369/500000) + dq1*dqr1*cos(q2)^2*sin(q5)*((23717*3^(1/2))/20000000 + 1369/1000000) + dq1*dqr1*cos(q3)^2*sin(q5)*((23717*3^(1/2))/20000000 + 1369/1000000) - (1369*3^(1/2)*dq5*dqr2*cos(q5)^2*sin(q4))/2000000 - (1073*dq1*dqr2*cos(q2)*cos(q4)*sin(q5))/100000 - (1073*dq1*dqr2*cos(q2)*cos(q5)*sin(q4))/200000 - (1073*dq2*dqr1*cos(q2)*cos(q4)*sin(q5))/100000 - (1073*dq2*dqr1*cos(q2)*cos(q5)*sin(q4))/200000 + (1073*dq2*dqr2*cos(q4)*cos(q5)*sin(q3))/200000 - (1073*dq2*dqr2*sin(q3)*sin(q4)*sin(q5))/100000 + dq1*dqr2*cos(q2)*sin(q4)*((18589*3^(1/2))/2000000 + 1073/100000) + dq2*dqr1*cos(q2)*sin(q4)*((18589*3^(1/2))/2000000 + 1073/100000) - dq2*dqr2*cos(q4)*sin(q3)*((18589*3^(1/2))/2000000 + 1073/100000) - (1369*3^(1/2)*dq5*dqr2*cos(q4)*cos(q5)*sin(q5))/4000000 + (1369*dq1*dqr1*cos(q2)^2*cos(q3)^2*cos(q5)*sin(q5))/1000000 - (1369*dq1*dqr2*cos(q2)*cos(q4)^2*cos(q5)^2*sin(q3))/800000 + (1369*dq1*dqr2*cos(q3)*cos(q4)^2*cos(q5)^2*sin(q2))/800000 + (1369*dq1*dqr1*cos(q2)^2*cos(q4)^2*cos(q5)*sin(q5))/1000000 + (1369*dq1*dqr1*cos(q3)^2*cos(q4)*cos(q5)^2*sin(q4))/800000 + (1369*dq1*dqr3*cos(q2)*cos(q4)^2*cos(q5)^2*sin(q3))/800000 - (1369*dq1*dqr3*cos(q3)*cos(q4)^2*cos(q5)^2*sin(q2))/800000 + (1369*dq1*dqr1*cos(q3)^2*cos(q4)^2*cos(q5)*sin(q5))/1000000 - dq1*dqr2*cos(q2)*cos(q4)^2*sin(q3)*((23717*3^(1/2))/10000000 + 1232643/400000000) + dq1*dqr2*cos(q3)*cos(q4)^2*sin(q2)*((23717*3^(1/2))/10000000 + 1232643/400000000) + dq1*dqr1*cos(q3)^2*cos(q4)*sin(q4)*((23717*3^(1/2))/10000000 + 1232643/400000000) + dq1*dqr3*cos(q2)*cos(q4)^2*sin(q3)*((23717*3^(1/2))/10000000 + 1232643/400000000) - dq1*dqr3*cos(q3)*cos(q4)^2*sin(q2)*((23717*3^(1/2))/10000000 + 1232643/400000000) + (32449*dq1*dqr2*cos(q2)*cos(q3)*cos(q4)*sin(q5))/4000000 + (32449*dq2*dqr1*cos(q2)*cos(q3)*cos(q4)*sin(q5))/4000000 - (32449*dq3*dqr1*cos(q2)*cos(q3)*cos(q4)*sin(q5))/4000000 + (4107*dq5*dqr1*cos(q2)*cos(q3)*cos(q5)*sin(q5))/4000000 - dq1*dqr1*cos(q2)^2*cos(q3)^2*sin(q5)*((23717*3^(1/2))/10000000 + 1369/500000) - dq1*dqr1*cos(q2)^2*cos(q4)^2*sin(q5)*((23717*3^(1/2))/10000000 + 1369/500000) - dq1*dqr1*cos(q3)^2*cos(q4)^2*sin(q5)*((23717*3^(1/2))/10000000 + 1369/500000) + (32449*dq1*dqr2*cos(q4)*sin(q2)*sin(q3)*sin(q5))/4000000 - (32449*dq1*dqr3*cos(q4)*sin(q2)*sin(q3)*sin(q5))/4000000 - dq1*dqr2*cos(q2)*cos(q5)*sin(q3)*((23717*3^(1/2))/20000000 + 1369/1000000) + dq1*dqr2*cos(q3)*cos(q5)*sin(q2)*((23717*3^(1/2))/20000000 + 1369/1000000) + dq1*dqr3*cos(q2)*cos(q5)*sin(q3)*((23717*3^(1/2))/20000000 + 1369/1000000) - dq1*dqr3*cos(q3)*cos(q5)*sin(q2)*((23717*3^(1/2))/20000000 + 1369/1000000) + dq2*dqr2*cos(q4)*cos(q5)*sin(q4)*((23717*3^(1/2))/20000000 + 1369/1000000) - dq3*dqr2*cos(q4)*cos(q5)*sin(q4)*((23717*3^(1/2))/20000000 + 1369/1000000) + dq5*dqr1*cos(q2)*cos(q3)*sin(q5)*((23717*3^(1/2))/40000000 + 1369/2000000) - dq1*dqr2*cos(q2)*cos(q3)*sin(q4)*((562157*3^(1/2))/80000000 + 32449/4000000) - dq1*dqr2*sin(q2)*sin(q3)*sin(q4)*((562157*3^(1/2))/80000000 + 32449/4000000) + dq1*dqr3*sin(q2)*sin(q3)*sin(q4)*((562157*3^(1/2))/80000000 + 32449/4000000) + dq1*dqr2*cos(q2)*cos(q4)^2*cos(q5)*sin(q3)*((23717*3^(1/2))/20000000 + 1369/1000000) - dq1*dqr2*cos(q3)*cos(q4)^2*cos(q5)*sin(q2)*((23717*3^(1/2))/20000000 + 1369/1000000) - dq1*dqr1*cos(q3)^2*cos(q4)*cos(q5)*sin(q4)*((23717*3^(1/2))/20000000 + 1369/1000000) - dq1*dqr3*cos(q2)*cos(q4)^2*cos(q5)*sin(q3)*((23717*3^(1/2))/20000000 + 1369/1000000) + dq1*dqr3*cos(q3)*cos(q4)^2*cos(q5)*sin(q2)*((23717*3^(1/2))/20000000 + 1369/1000000) + (1369*3^(1/2)*dq1*dqr2*cos(q2)*cos(q3)*cos(q5)^2*sin(q4))/4000000 - (1369*3^(1/2)*dq1*dqr3*cos(q2)*cos(q3)*cos(q5)^2*sin(q4))/4000000 + (1369*3^(1/2)*dq1*dqr2*cos(q5)^2*sin(q2)*sin(q3)*sin(q4))/4000000 - (1369*3^(1/2)*dq1*dqr3*cos(q5)^2*sin(q2)*sin(q3)*sin(q4))/4000000 - (1369*dq1*dqr1*cos(q2)^2*cos(q3)^2*cos(q4)^2*cos(q5)*sin(q5))/500000 - dq1*dqr2*cos(q2)*cos(q3)*cos(q5)*sin(q4)*((1369*3^(1/2))/2000000 - 45547/20000000) + dq1*dqr3*cos(q2)*cos(q3)*cos(q5)*sin(q4)*((1369*3^(1/2))/2000000 - 45547/20000000) + dq1*dqr1*cos(q2)^2*cos(q3)^2*cos(q4)^2*sin(q5)*((23717*3^(1/2))/5000000 + 1369/250000) - dq1*dqr2*cos(q5)*sin(q2)*sin(q3)*sin(q4)*((1369*3^(1/2))/2000000 - 45547/20000000) + dq1*dqr3*cos(q5)*sin(q2)*sin(q3)*sin(q4)*((1369*3^(1/2))/2000000 - 45547/20000000) + (1369*dq1*dqr2*cos(q2)*cos(q4)*cos(q5)*sin(q3)*sin(q4)*sin(q5))/1000000 - (1369*dq1*dqr2*cos(q3)*cos(q4)*cos(q5)*sin(q2)*sin(q4)*sin(q5))/1000000 - (1369*dq1*dqr3*cos(q2)*cos(q4)*cos(q5)*sin(q3)*sin(q4)*sin(q5))/1000000 + (1369*dq1*dqr3*cos(q3)*cos(q4)*cos(q5)*sin(q2)*sin(q4)*sin(q5))/1000000 - dq1*dqr2*cos(q2)*cos(q4)*sin(q3)*sin(q4)*sin(q5)*((23717*3^(1/2))/10000000 + 1369/500000) + dq1*dqr2*cos(q3)*cos(q4)*sin(q2)*sin(q4)*sin(q5)*((23717*3^(1/2))/10000000 + 1369/500000) + dq1*dqr3*cos(q2)*cos(q4)*sin(q3)*sin(q4)*sin(q5)*((23717*3^(1/2))/10000000 + 1369/500000) - dq1*dqr3*cos(q3)*cos(q4)*sin(q2)*sin(q4)*sin(q5)*((23717*3^(1/2))/10000000 + 1369/500000) + (1369*3^(1/2)*dq1*dqr2*cos(q2)*cos(q3)*cos(q4)*cos(q5)*sin(q5))/2000000 + (1369*3^(1/2)*dq2*dqr1*cos(q2)*cos(q3)*cos(q4)*cos(q5)*sin(q5))/2000000 - (1369*3^(1/2)*dq3*dqr1*cos(q2)*cos(q3)*cos(q4)*cos(q5)*sin(q5))/2000000 + (1369*3^(1/2)*dq1*dqr2*cos(q4)*cos(q5)*sin(q2)*sin(q3)*sin(q5))/2000000 - (1369*3^(1/2)*dq1*dqr3*cos(q4)*cos(q5)*sin(q2)*sin(q3)*sin(q5))/2000000;
